simulink model "MATLAB_TEST"  (R2019b)
settings: Solver=FixedStepDiscrete  StartTime=0  StopTime=50  FixedStep=0.0025  RelTol=1e-3
undefined symbols (not defined in the file): BCM_COM_PROC_P20, BCM_COM_PROC_P20_SFW_R2018b, BCM_COM_PROC_P2_5, BCM_COM_PROC_P2_5_SFW_R2018b, BCM_COM_PROC_P5, BCM_COM_PROC_P5_SFW_R2018b, BCMA_ACCU_PT_Conf_Flt, BCMA_ACCU_PT_Unconf_Flt, BCMA_Antiskid_Off_Sanction, BCMA_Avionics_Conf_Flt, BCMA_BCM_CCDL_Conf_Flt, BCMA_BCM_CCDL_Unconf_Flt, BCMA_BCM_DBCU_INHIBITION_Conf_Flt, BCMA_BCM_DBCU_INHIBITION_Unconf_Flt, BCMA_BCP_ALT_Disp_Sw_Conf_Flt, BCMA_BCP_ALT_Disp_Sw_Unconf_Flt, BCMA_BCP_ALT_SW_ON_CMD_Conf_Flt, BCMA_BCP_ALT_SW_ON_CMD_Unconf_Flt, BCMA_BCP_PARK_OFF_SW_CMD_Conf_Flt, BCMA_BCP_PARK_OFF_SW_CMD_Unconf_Flt, BCMA_CF_BSELV_JCL, BCMA_CF_BSELV_JOP, BCMA_CF_BSELV_OC, BCMA_CF_BSELV_SC, BCMA_CF_LH_SV_JCL, BCMA_CF_LH_SV_JOP, BCMA_CF_LH_SV_OC, BCMA_CF_LH_SV_SC, BCMA_CF_PARK_BRK, BCMA_CF_RESIDUAL_PRESS, BCMA_CF_RH_SV_JCL, BCMA_CF_RH_SV_JOP, BCMA_CF_RH_SV_OC, BCMA_CF_RH_SV_SC, BCMA_CF_SELV_JCL, BCMA_CF_SELV_JOP, BCMA_CF_SELV_OC, BCMA_CF_SELV_SC, BCMA_CF_SV_DRIFT, BCMA_DBCU_ALT_MODE_Conf_Flt, BCMA_DBCU_ALT_MODE_Unconf_Flt, BCMA_DBCU_BRK_ORDER_FAIL_Conf_Flt, BCMA_DBCU_BRK_ORDER_FAIL_Unconf_Flt, BCMA_DBCU_Conf_Flt, BCMA_DBCU_DISPATCH_SW_ON_Conf_Flt, BCMA_DBCU_DISPATCH_SW_ON_Unconf_Flt, BCMA_DBCU_FAILED_Conf_Flt, BCMA_DBCU_FAILED_Unconf_Flt, BCMA_DFCS1_Capsule_Validity, BCMA_DFCS1_Label202_Corrupted, BCMA_DFCS1_Label202_Not_Refreshed, BCMA_DFCS1_Label204_Corrupted, BCMA_DFCS1_Label204_Not_Refreshed, BCMA_DFCS1_Label205_Corrupted, BCMA_DFCS1_Label205_Not_Refreshed, BCMA_DFCS1_Label206_Corrupted, BCMA_DFCS1_Label206_Not_Refreshed, BCMA_DFCS1_Label207_Corrupted, BCMA_DFCS1_Label207_Not_Refreshed, BCMA_DFCS3_Capsule_Validity ... (+762)
libraries: simulink x73, lib_MBD_Control x5
(part 2 of 16)

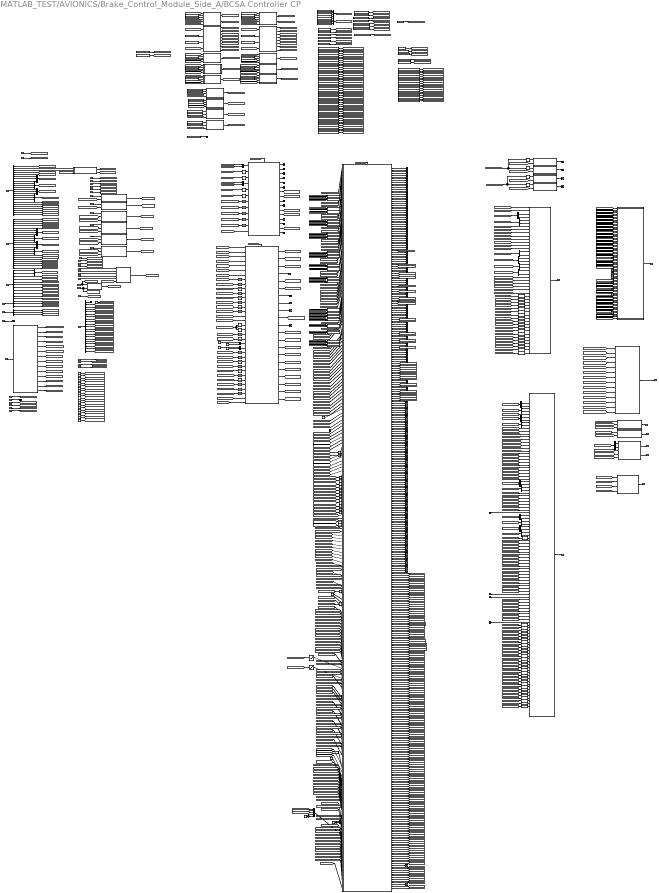
== system MATLAB_TEST/AVIONICS/Brake_Control_Module_Side_A/BCSA Controller CP ==
  note: Wheel speed order:
      | 1) Left outer
      | 2) Left inner
      | 3) Right inner
      | 4) Right outer
  note: MEX P2_5
  note: MEX P20
  note: Temporary
      | Flt computation
  note: Validity
  note: Temporary inputs
  note: Functional test
  note: MEX P5
  note: Outputs connected
  note: COM CAN MON
  note: INPUTS
  note: OUTPUTS
  note: LABEL202
  note: LABEL204
  note: LABEL205
  note: LABEL206
  note: LABEL207
  note: DFCS1
  note: DFCS3
  note: GenIO
  note: LABEL021
  note: LABEL022
  note: LABEL272
  note: LABEL273
  note: SOFTWARE
  note: Capsule validity
  note: DFCS
  note: GenIO
  note: Ethernet
  note: Only BCM A
  note: Only BCM A
  note: CAN
  note: ToDo 27439:
      | a temporary fix was implemented for MEX4
      | The data is transformed from mV into bar
      | To be deleted for future MEX release if relevant
  note: ToDo 27975
      | Fix to force the validity of SP to true inside CP
  note: MON CAN COM
  BCP_ALT_SW_ON_CMD_BCM_A_GND : Inport  Tag=ToConnect
  BCP_PARK_OFF_SW_CMD_BCM_A_GND : Inport  Tag=ToConnect  Port=2
  BUS_A429_DFCS1_BCMA : Inport  Tag=ToConnect  Port=3
  BUS_A429_DFCS3_BCMA : Inport  Tag=ToConnect  Port=4
  BUS_A429_GenIO_1A_GPHS : Inport  Tag=ToConnect  Port=5
  BUS_A429_LH_WRDC_BCM : Inport  Tag=ToConnect  Port=6
  BUS_A429_RH_WRDC_BCM : Inport  Tag=ToConnect  Port=7
  BUS_ETH_MMS_BCMA : Inport  Tag=ToConnect  Port=8
  BUS_CAN_BCM_CCDL_RX : Inport  Tag=ToConnect  Port=9
  LGCH_LG_LEVER_UP_1 : Inport  Tag=ToConnect  Port=10
  LH_ESC_WOnWdiscrete : Inport  Tag=ToConnect  Port=11
  LMLG_DOWN_LOCKED_BCM_1 : Inport  Tag=ToConnect  Port=12
  MP_MAINT_MODE_CMD_BCM_A_28V : Inport  Tag=ToConnect  Port=13
  MP_MAINT_MODE_CMD_BCM_A_GND : Inport  Tag=ToConnect  Port=14
  RMLG_DOWN_LOCKED_BCM_1 : Inport  Tag=ToConnect  Port=15
  ACCU_PT_PRESSURE : Inport  Tag=ToConnect  Port=16
  BCMB_DBCU_INHIBITION : Inport  Tag=ToConnect  Port=17
  DBCU_ALTERNATE_MODE_1 : Inport  Tag=ToConnect  Port=18
  DBCU_BRK_ORDER_FAIL_BCMA : Inport  Tag=ToConnect  Port=19
  DBCU_FAILED_BCMA : Inport  Tag=ToConnect  Port=20
  LH_DBCU_BRK_CMD_FEEDBACK : Inport  Tag=ToConnect  Port=21
  LH_HASV_PT_PRESSURE : Inport  Tag=ToConnect  Port=22
  LH_IN_WHEEL_SPEED_COIL1 : Inport  Tag=ToConnect  Port=23
  LH_OUT_BTS_TEMP : Inport  Tag=ToConnect  Port=24
  LH_OUT_WHEEL_SPEED_COIL1 : Inport  Tag=ToConnect  Port=25
  PBSELV_ON_POS : Inport  Tag=ToConnect  Port=26
  RH_DBCU_BRK_CMD_FEEDBACK : Inport  Tag=ToConnect  Port=27
  RH_HASV_PT_PRESSURE : Inport  Tag=ToConnect  Port=28
  RH_IN_WHEEL_SPEED_COIL1 : Inport  Tag=ToConnect  Port=29
  RH_OUT_BTS_TEMP : Inport  Tag=ToConnect  Port=30
  RH_OUT_WHEEL_SPEED_COIL1 : Inport  Tag=ToConnect  Port=31
  FTI_BCMA_switch_1 : Inport  Tag=ToConnect  Port=32
  FTI_BCMA_switch_2 : Inport  Tag=ToConnect  Port=33
  FTI_BCMA_switch_3 : Inport  Tag=ToConnect  Port=34
  FTI_BCMA_switch_4 : Inport  Tag=ToConnect  Port=35
  FTI_BCMA_switch_5 : Inport  Tag=ToConnect  Port=36
  PIN_PROG_BCMA_1 : Inport  Tag=ToConnect  Port=37
  PIN_PROG_BCMA_2 : Inport  Tag=ToConnect  Port=38
  PIN_PROG_BCMA_3 : Inport  Tag=ToConnect  Port=39
  MON_CAN_COM : Inport  Tag=ToConnect  Port=40
  Control_Path_Start_Up : Inport  Tag=ToConnect  Port=41
  LH_HASV_CURRENT_COIL1_Readback : Inport  Tag=ToConnect  Port=42  OutDataTypeStr=double
  RH_HASV_CURRENT_COIL1_Readback : Inport  Tag=ToConnect  Port=43  OutDataTypeStr=double
  HASELV_CMD_Readback : Inport  Tag=ToConnect  Port=44  OutDataTypeStr=double
  BCM Config Computation : Subsystem
  BCMA_COM_UF_LOCKED_WHEEL_W{1..4} (4 alike) : Constant  Value=0  OutDataTypeStr=boolean
  BCM_COM_PROC_P20 : Subsystem  SystemSampleTime=0.02
  BCM_COM_PROC_P2_5 : Subsystem  SystemSampleTime=0.0025
  BCM_COM_PROC_P5 : Subsystem  SystemSampleTime=0.005
  BUS_A429_BCMA_DFCS13_TX : Subsystem
  BUS_A429_BCMA_GenIO_2_TX : Subsystem
  BUS_CAN_BCM_CCDL_RX_ : Subsystem
  BUS_CAN_BCM_CCDL_TX : Subsystem
  BUS_ETH_BCMA_MMS_TX : Subsystem
  Bus Selector : BusSelector  OutputSignals=BUS_A429_DFCS1_BCMA_LABEL_206_Ground_Speed,BUS_A429_DFCS1_BCMA_LABEL_202_DFCS_LH_Braking_Cmd,BUS_A429_DFCS1_BCMA_LABEL_202_DFCS_RH_Braking_Cmd,BUS_A429_DFCS1_BCMA_LABEL_205_Longitudinal_Acceleration,BUS_A429_DFCS1_BCMA_LABEL_207_Pitch_Angle,BUS_A429_DFCS1_BCMA_LABEL_204_DATA_BIT_14_WOW1_Validity,BUS_A429_DFCS1_BCMA_LABEL_204_DATA_BIT_18_WOW2_Validity,BUS_A429_DFCS1_BCMA_LABEL_204_DATA_BIT_22_WOW3_Validity,BUS_A429_DFCS1_BCMA_LABEL_204_DATA_BIT_12_WOW1_LMLG,BUS_A429_DFCS1_BCMA_LABEL_204_DATA_BIT_16_WOW2_LMLG,BUS_A429_DFCS1_BCMA_LABEL_204_DATA_BIT_20_WOW3_LMLG,BUS_A429_DFCS1_BCMA_LABEL_204_DATA_BIT_13_WOW1_RMLG,BUS_A429_DFCS1_BCMA_LABEL_204_DATA_BIT_17_WOW2_RMLG,BUS_A429_DFCS1_BCMA_LABEL_204_DATA_BIT_21_WOW3_RMLG,BUS_A429_DFCS1_BCMA_LABEL_204_DATA_BIT_11_WOW1_NLG,BUS_A429_DFCS1_BCMA_LABEL_204_DATA_BIT_15_WOW2_NLG,BUS_A429_DFCS1_BCMA_LABEL_204_DATA_BIT_19_WOW3_NLG,BUS_A429_DFCS1_BCMA_LABEL_204_DATA_BIT_24_Decel_Law_Inhibition,BUS_A429_DFCS1_BCMA_LABEL_204_DATA_BIT_27_TLA_Above_Idle,BUS_A429_DFCS1_BCMA_LABEL_202_SSM,BUS_A429_DFCS1_BCMA_LABEL_204_SSM,BUS_A429_DFCS1_BCMA_LABEL_205_SSM,BUS_A429_DFCS1_BCMA_LABEL_206_SSM,BUS_A429_DFCS1_BCMA_LABEL_207_SSM
  Bus Selector1 : BusSelector  OutputSignals=BUS_A429_DFCS3_BCMA_LABEL_206_Ground_Speed,BUS_A429_DFCS3_BCMA_LABEL_202_DFCS_LH_Braking_Cmd,BUS_A429_DFCS3_BCMA_LABEL_202_DFCS_RH_Braking_Cmd,BUS_A429_DFCS3_BCMA_LABEL_205_Longitudinal_Acceleration,BUS_A429_DFCS3_BCMA_LABEL_207_Pitch_Angle,BUS_A429_DFCS3_BCMA_LABEL_204_DATA_BIT_14_WOW1_Validity,BUS_A429_DFCS3_BCMA_LABEL_204_DATA_BIT_18_WOW2_Validity,BUS_A429_DFCS3_BCMA_LABEL_204_DATA_BIT_22_WOW3_Validity,BUS_A429_DFCS3_BCMA_LABEL_204_DATA_BIT_12_WOW1_LMLG,BUS_A429_DFCS3_BCMA_LABEL_204_DATA_BIT_16_WOW2_LMLG,BUS_A429_DFCS3_BCMA_LABEL_204_DATA_BIT_20_WOW3_LMLG,BUS_A429_DFCS3_BCMA_LABEL_204_DATA_BIT_13_WOW1_RMLG,BUS_A429_DFCS3_BCMA_LABEL_204_DATA_BIT_17_WOW2_RMLG,BUS_A429_DFCS3_BCMA_LABEL_204_DATA_BIT_21_WOW3_RMLG,BUS_A429_DFCS3_BCMA_LABEL_204_DATA_BIT_11_WOW1_NLG,BUS_A429_DFCS3_BCMA_LABEL_204_DATA_BIT_15_WOW2_NLG,BUS_A429_DFCS3_BCMA_LABEL_204_DATA_BIT_19_WOW3_NLG,BUS_A429_DFCS3_BCMA_LABEL_204_DATA_BIT_24_Decel_Law_Inhibition,BUS_A429_DFCS3_BCMA_LABEL_204_DATA_BIT_27_TLA_Above_Idle,BUS_A429_DFCS3_BCMA_LABEL_202_SSM,BUS_A429_DFCS3_BCMA_LABEL_204_SSM,BUS_A429_DFCS3_BCMA_LABEL_205_SSM,BUS_A429_DFCS3_BCMA_LABEL_206_SSM,BUS_A429_DFCS3_BCMA_LABEL_207_SSM
  Bus Selector2 : BusSelector  OutputSignals=BUS_A429_GenIO_1A_GPHS_LABEL_272_ENG1_Engine_Running,BUS_A429_GenIO_1A_GPHS_LABEL_273_ENG2_Engine_Running,BUS_A429_GenIO_1A_GPHS_LABEL_022_HCM_SYS_A_PRESSURE,BUS_A429_GenIO_1A_GPHS_LABEL_021_HCM_SYS_B_PRESSURE,BUS_A429_GenIO_1A_GPHS_LABEL_150_UTC_time_hours_2,BUS_A429_GenIO_1A_GPHS_LABEL_150_UTC_time_minutes_2,BUS_A429_GenIO_1A_GPHS_LABEL_150_UTC_time_seconds_2,BUS_A429_GenIO_1A_GPHS_LABEL_021_SSM,BUS_A429_GenIO_1A_GPHS_LABEL_022_SSM,BUS_A429_GenIO_1A_GPHS_LABEL_272_SSM,BUS_A429_GenIO_1A_GPHS_LABEL_273_SSM
  Bus Selector3 : BusSelector  OutputSignals=V_BCMA_MON_BCM_Validity_SP,V_BCMA_MON_A429_SSM_DFCS_Label_121,V_BCMA_MON_A429_SSM_DFCS_Label_122,V_BCMA_MON_A429_SSM_DFCS_Label_123,V_BCMA_MON_A429_SSM_DFCS_Label_124,V_BCMA_MON_A429_SSM_DFCS_Label_125,V_BCMA_MON_A429_SSM_DFCS_Label_126,V_BCMA_MON_A429_SSM_DFCS_Label_127,V_BCMA_MON_A429_SSM_DFCS_Label_130,V_BCMA_MON_A429_SSM_DFCS_Label_131,V_BCMA_MON_A429_SSM_DFCS_Label_150,V_BCMA_MON_A429_SSM_DFCS_Label_151,V_BCMA_MON_A429_SP_Wheel_Speed_W12,V_BCMA_MON_A429_SP_Wheel_Speed_W34,V_BCMA_MON_A429_SP_SV_PT_PSI,V_BCMA_MON_A429_SP_LH_Brkg_Cmd_Fdbk,V_BCMA_MON_A429_SP_RH_Brkg_Cmd_Fdbk,V_BCMA_MON_A429_SP_DFCS_A_Caps_Fail,V_BCMA_MON_A429_SP_DFCS_B_Caps_Fail,V_BCMA_MON_A429_SP_BCM_Passivated,V_BCMA_MON_A429_SP_BCM_Failed
  Bus Selector4 : BusSelector  OutputSignals=BUS_A429_LH_WRDC_BCM_LABEL_300_TyrePressure_W_1_R_LN,BUS_A429_LH_WRDC_BCM_LABEL_301_TyrePressure_W_2_R_LN,BUS_A429_LH_WRDC_BCM_LABEL_302_TyrePressure_W_3_R_LN
  Bus Selector5 : BusSelector  OutputSignals=BUS_A429_RH_WRDC_BCM_LABEL_300_TyrePressure_W_1_R_LN,BUS_A429_RH_WRDC_BCM_LABEL_301_TyrePressure_W_2_R_LN,BUS_A429_RH_WRDC_BCM_LABEL_302_TyrePressure_W_3_R_LN
  COM_CAN_MON_TX : Subsystem
  Constant{,35..36,44,87,94,97,100..101,104,107..118} (22 alike) : Constant  Value=0  OutDataTypeStr=boolean
  Constant1 : Constant  Value=BCMA_DFCS1_Label206_Not_Refreshed  OutDataTypeStr=boolean  SampleTime=Inf
  Constant10 : Constant  Value=BCMA_DFCS1_Label202_Not_Refreshed  OutDataTypeStr=boolean  SampleTime=Inf
  Constant11 : Constant  Value=BCMA_DFCS1_Label204_Not_Refreshed  OutDataTypeStr=boolean  SampleTime=Inf
  Constant119 : Constant  Value=BCMA_UTC_Time_Seconds_Unconf_Flt
  Constant12 : Constant  Value=BCMA_DFCS1_Label205_Not_Refreshed  OutDataTypeStr=boolean  SampleTime=Inf
  Constant120 : Constant  Value=BCMA_DBCU_BRK_ORDER_FAIL_Conf_Flt
  Constant121 : Constant  Value=BCMA_DBCU_BRK_ORDER_FAIL_Unconf_Flt
  Constant122 : Constant  Value=BCMA_DBCU_DISPATCH_SW_ON_Conf_Flt
  Constant123 : Constant  Value=BCMA_DBCU_DISPATCH_SW_ON_Unconf_Flt
  Constant124 : Constant  Value=BCMA_LH_DBCU_BRK_CMD_FDBK_Conf_Flt
  Constant125 : Constant  Value=BCMA_LH_DBCU_BRK_CMD_FDBK_Unconf_Flt
  Constant126 : Constant  Value=BCMA_RH_DBCU_BRK_CMD_FDBK_Conf_Flt
  Constant127 : Constant  Value=BCMA_RH_DBCU_BRK_CMD_FDBK_Unconf_Flt
  Constant128 : Constant  Value=BCMA_DBCU_FAILED_Conf_Flt
  Constant129 : Constant  Value=BCMA_BCM_CCDL_Unconf_Flt
  Constant13 : Constant  Value=BCMA_DFCS1_Label205_Corrupted  OutDataTypeStr=boolean  SampleTime=Inf
  Constant130 : Constant  Value=BCMA_DBCU_FAILED_Unconf_Flt
  Constant131 : Constant  Value=BCMA_DBCU_ALT_MODE_Conf_Flt
  Constant132 : Constant  Value=BCMA_DBCU_ALT_MODE_Unconf_Flt
  Constant133 : Constant  Value=BCMA_ACCU_PT_Conf_Flt
  Constant134 : Constant  Value=BCMA_ACCU_PT_Unconf_Flt
  Constant135 : Constant  Value=BCMA_LH_BTS_Conf_Flt
  Constant136 : Constant  Value=BCMA_LH_BTS_Unconf_Flt
  Constant137 : Constant  Value=BCMA_RH_BTS_Conf_Flt
  Constant138 : Constant  Value=BCMA_RH_BTS_Unconf_Flt
  Constant139 : Constant  Value=BCMA_BCP_PARK_OFF_SW_CMD_Conf_Flt
  Constant14 : Constant  Value=BCMA_DFCS1_Label207_Not_Refreshed  OutDataTypeStr=boolean  SampleTime=Inf
  Constant140 : Constant  Value=BCMA_BCM_DBCU_INHIBITION_Conf_Flt
  Constant141 : Constant  Value=BCMA_BCP_PARK_OFF_SW_CMD_Unconf_Flt
  Constant142 : Constant  Value=BCMA_LNLG_Tire_Press_Conf_Flt
  Constant143 : Constant  Value=BCMA_LNLG_Tire_Press_Unconf_Flt
  Constant144 : Constant  Value=BCMA_RNLG_Tire_Press_Conf_Flt
  Constant145 : Constant  Value=BCMA_RNLG_Tire_Press_Unconf_Flt
  Constant146 : Constant  Value=BCMA_LMLG_Outboard_Tire_Press_Conf_Flt
  Constant147 : Constant  Value=BCMA_LMLG_Outboard_Tire_Press_Unconf_Flt
  Constant148 : Constant  Value=BCMA_LMLG_Inboard_Tire_Press_Conf_Flt
  Constant149 : Constant  Value=BCMA_LMLG_Inboard_Tire_Press_Unconf_Flt
  Constant15 : Constant  Value=BCMA_DFCS1_Label206_Corrupted  OutDataTypeStr=boolean  SampleTime=Inf
  Constant150 : Constant  Value=BCMA_RMLG_Inboard_Tire_Press_Conf_Flt
  Constant151 : Constant  Value=BCMA_BCM_DBCU_INHIBITION_Unconf_Flt
  Constant152 : Constant  Value=BCMA_RMLG_Inboard_Tire_Press_Unconf_Flt
  Constant153 : Constant  Value=BCMA_RMLG_Outboard_Tire_Press_Conf_Flt
  Constant154 : Constant  Value=BCMA_RMLG_Outboard_Tire_Press_Unconf_Flt
  Constant155 : Constant  Value=BCMA_Avionics_Conf_Flt
  Constant156 : Constant  Value=BCMA_DFCS_A_Conf_Flt
  Constant157 : Constant  Value=BCMA_DFCS_B_Conf_Flt
  Constant158 : Constant  Value=BCMA_DBCU_Conf_Flt
  Constant159 : Constant  Value=BCMA_LH_SV_PT_Conf_Flt
  Constant16 : Constant  Value=BCMA_Tacho1_Conf_Flt  OutDataTypeStr=boolean  SampleTime=Inf
  Constant160 : Constant  Value=BCMA_RH_SV_PT_Conf_Flt
  Constant161 : Constant  Value=BCMA_UTC_Time_Hours_Conf_Flt
  Constant162 : Constant  Value=BCMA_UTC_Time_Hours_Unconf_Flt
  Constant163 : Constant  Value=BCMA_UTC_Time_Minutes_Conf_Flt
  Constant164 : Constant  Value=BCMA_UTC_Time_Minutes_Unconf_Flt
  Constant165 : Constant  Value=BCMA_UTC_Time_Seconds_Conf_Flt
  Constant17 : Constant  Value=BCMA_DFCS1_Label207_Corrupted  OutDataTypeStr=boolean  SampleTime=Inf
  Constant18 : Constant  Value=BCMA_DFCS3_Label205_Corrupted  OutDataTypeStr=boolean  SampleTime=Inf
  Constant19 : Constant  Value=BCMA_DFCS3_Label202_Not_Refreshed  OutDataTypeStr=boolean  SampleTime=Inf
  Constant2 : Constant  Value=BCMA_Tacho1_Unconf_Flt  OutDataTypeStr=boolean  SampleTime=Inf
  Constant20 : Constant  Value=BCMA_DFCS3_Label206_Not_Refreshed  OutDataTypeStr=boolean  SampleTime=Inf
  Constant21 : Constant  Value=BCMA_DFCS3_Label202_Corrupted  OutDataTypeStr=boolean  SampleTime=Inf
  Constant22 : Constant  Value=BCMA_DFCS3_Label206_Corrupted  OutDataTypeStr=boolean  SampleTime=Inf
  Constant23 : Constant  Value=BCMA_DFCS3_Label207_Not_Refreshed  OutDataTypeStr=boolean  SampleTime=Inf
  Constant24 : Constant  Value=BCMA_DFCS3_Label207_Corrupted  OutDataTypeStr=boolean  SampleTime=Inf
  Constant25 : Constant  Value=BCMA_Off_Sanction  OutDataTypeStr=boolean  SampleTime=Inf
  Constant26 : Constant  OutDataTypeStr=boolean
  Constant27 : Constant  Value=BCMA_SP_TO_CP_Link_Validity  OutDataTypeStr=boolean  SampleTime=Inf
  Constant29 : Constant  Value=BCMA_BCP_ALT_SW_ON_CMD_Unconf_Flt  OutDataTypeStr=boolean  SampleTime=Inf
  Constant3 : Constant  Value=BCMA_DFCS3_Label204_Not_Refreshed  OutDataTypeStr=boolean  SampleTime=Inf
  Constant30 : Constant  Value=BCMA_BCM_CCDL_Conf_Flt
  Constant31 : Constant  Value=BCMA_GenIO_1A_Label021_Not_Refreshed  OutDataTypeStr=boolean  SampleTime=Inf
  Constant32 : Constant  Value=BCMA_GenIO_1A_Label021_Corrupted  OutDataTypeStr=boolean  SampleTime=Inf
  Constant33 : Constant  Value=BCMA_GenIO_1A_Label022_Not_Refreshed  OutDataTypeStr=boolean  SampleTime=Inf
  Constant34 : Constant  Value=BCMA_GenIO_1A_Label022_Corrupted  OutDataTypeStr=boolean  SampleTime=Inf
  Constant37 : Constant  Value=BCMA_GenIO_1A_Label272_Not_Refreshed  OutDataTypeStr=boolean  SampleTime=Inf
  Constant38 : Constant  Value=BCMA_LG_Lever_Up_Unconf_Flt  OutDataTypeStr=boolean  SampleTime=Inf
  Constant39 : Constant  Value=BCMA_LG_Lever_Up_Conf_Flt  OutDataTypeStr=boolean  SampleTime=Inf
  Constant4 : Constant  Value=BCMA_DFCS1_Label202_Corrupted  OutDataTypeStr=boolean  SampleTime=Inf
  Constant40 : Constant  Value=BCMA_LMLG_Downlock_Unconf_Flt  OutDataTypeStr=boolean  SampleTime=Inf
  Constant41 : Constant  Value=BCMA_LMLG_Downlock_Conf_Flt  OutDataTypeStr=boolean  SampleTime=Inf
  Constant42 : Constant  Value=BCMA_RMLG_Downlock_Unconf_Flt  OutDataTypeStr=boolean  SampleTime=Inf
  Constant43 : Constant  Value=BCMA_RMLG_Downlock_Conf_Flt  OutDataTypeStr=boolean  SampleTime=Inf
  Constant45 : Constant  Value=BCMA_CF_LH_SV_SC
  Constant46 : Constant  Value=BCMA_BCP_ALT_SW_ON_CMD_Conf_Flt  OutDataTypeStr=boolean  SampleTime=Inf
  Constant47 : Constant  Value=BCMA_BCP_ALT_Disp_Sw_Unconf_Flt  OutDataTypeStr=boolean  SampleTime=Inf
  Constant48 : Constant  Value=BCMA_BCP_ALT_Disp_Sw_Conf_Flt  OutDataTypeStr=boolean  SampleTime=Inf
  Constant49 : Constant  Value=BCMA_GenIO_1A_Label272_Corrupted  OutDataTypeStr=boolean  SampleTime=Inf
  Constant5 : Constant  Value=BCMA_DFCS3_Label204_Corrupted  OutDataTypeStr=boolean  SampleTime=Inf
  Constant50 : Constant  Value=BCMA_Antiskid_Off_Sanction  OutDataTypeStr=boolean  SampleTime=Inf
  Constant51 : Constant  Value=BCMA_Norm_Brk_Off_Sanction  OutDataTypeStr=boolean  SampleTime=Inf
  Constant52 : Constant  Value=0  OutDataTypeStr=int32  SampleTime=Inf
  Constant54 : Constant  Value=BCMA_Tacho2_Conf_Flt  OutDataTypeStr=boolean  SampleTime=Inf
  Constant55 : Constant  Value=BCMA_GenIO_1A_Label273_Not_Refreshed  OutDataTypeStr=boolean  SampleTime=Inf
  Constant56 : Constant  Value=BCMA_GenIO_1A_Label273_Corrupted  OutDataTypeStr=boolean  SampleTime=Inf
  Constant57 : Constant  Value=BCMA_CF_RESIDUAL_PRESS
  Constant58 : Constant  Value=BCMA_CF_BSELV_OC
  Constant59 : Constant  Value=BCMA_CF_BSELV_SC
  Constant6 : Constant  Value=BCMA_DFCS1_Label204_Corrupted  OutDataTypeStr=boolean  SampleTime=Inf
  Constant60 : Constant  Value=BCMA_CF_BSELV_JCL
  Constant61 : Constant  Value=BCMA_CF_BSELV_JOP
  Constant62 : Constant  Value=BCMA_PPRG_Fault
  Constant63 : Constant  Value=BCMA_CF_SV_DRIFT
  Constant64 : Constant  Value=BCMA_CF_LH_SV_JCL
  Constant65 : Constant  Value=BCMA_CF_LH_SV_JOP
  Constant67 : Constant  Value=BCMA_CF_LH_SV_OC
  Constant68 : Constant  Value=BCMA_CF_RH_SV_JCL
  Constant69 : Constant  Value=BCMA_CF_RH_SV_JOP
  Constant7 : Constant  Value=BCMA_DFCS3_Label205_Not_Refreshed  OutDataTypeStr=boolean  SampleTime=Inf
  Constant70 : Constant  Value=BCMA_CF_RH_SV_SC
  Constant71 : Constant  Value=BCMA_CF_RH_SV_OC
  Constant72 : Constant  Value=BCMA_Tacho3_Conf_Flt  OutDataTypeStr=boolean  SampleTime=Inf
  Constant73 : Constant  Value=BCMA_Tacho4_Conf_Flt  OutDataTypeStr=boolean  SampleTime=Inf
  Constant74 : Constant  Value=BCMA_Tacho2_Unconf_Flt  OutDataTypeStr=boolean  SampleTime=Inf
  Constant75 : Constant  Value=BCMA_Tacho3_Unconf_Flt  OutDataTypeStr=boolean  SampleTime=Inf
  Constant76 : Constant  Value=BCMA_Tacho4_Unconf_Flt  OutDataTypeStr=boolean  SampleTime=Inf
  Constant77 : Constant  Value=BCMA_CF_SELV_SC
  Constant78 : Constant  Value=BCMA_CF_SELV_OC
  Constant79 : Constant  Value=BCMA_CF_SELV_JOP
  Constant8 : Constant  Value=BCMA_DFCS1_Capsule_Validity  OutDataTypeStr=boolean  SampleTime=Inf
  Constant80 : Constant  Value=BCMA_LH_ALT_BRK_LOSS_Manual  OutDataTypeStr=boolean  SampleTime=Inf
  Constant81 : Constant  Value=BCMA_RH_ALT_BRK_LOSS_Manual  OutDataTypeStr=boolean  SampleTime=Inf
  Constant82 : Constant  Value=BCMA_PBSELV_ON_POS_Unconf_Flt  OutDataTypeStr=boolean  SampleTime=Inf
  Constant83 : Constant  Value=BCMA_PBSELV_ON_POS_Conf_Flt  OutDataTypeStr=boolean  SampleTime=Inf
  Constant84 : Constant  Value=BCMA_CF_SELV_JCL
  Constant85 : Constant  Value=BCMA_CF_PARK_BRK
  Constant88 : Constant  Value=BCMA_LH_SV_PT_Unconf_Flt  OutDataTypeStr=boolean  SampleTime=Inf
  Constant9 : Constant  Value=BCMA_DFCS3_Capsule_Validity  OutDataTypeStr=boolean  SampleTime=Inf
  Constant90 : Constant  Value=BCMA_RH_SV_PT_Unconf_Flt  OutDataTypeStr=boolean  SampleTime=Inf
  DBCU Inhibition Failure Mode : Subsystem
  DFCS1_Label204_Validity : Subsystem
  DFCS1_Label205_Validity : Subsystem
  DFCS1_Label206_Validity : Subsystem
  DFCS1_Label207_Validity : Subsystem
  DFCS3_Label204_Validity : Subsystem
  DFCS3_Label205_Validity : Subsystem
  DFCS3_Label206_Validity : Subsystem
  DFCS3_Label207_Validity : Subsystem
  DFCSA_DCL_Inhibition_Comp : Subsystem
  DFCSA_Ground_Speed_Comp : Subsystem
  DFCSA_LH_Braking_Cmd_Comp : Subsystem
  DFCSA_LMLG_WOWs_Comp : Subsystem
  DFCSA_Label202_Validity : Subsystem
  DFCSA_Long_Accel_Comp : Subsystem
  DFCSA_NLG_WOWs_Comp : Subsystem
  DFCSA_Pitch_Angle_Comp : Subsystem
  DFCSA_RH_Braking_Cmd_Comp : Subsystem
  DFCSA_RMLG_WOWs_Comp : Subsystem
  DFCSA_TLA_Above_Idle_Comp : Subsystem
  DFCSA_WOWs_Val_Comp : Subsystem
  DFCSB_DCL_Inhibition_Comp : Subsystem
  DFCSB_Ground_Speed_Comp : Subsystem
  DFCSB_LH_Braking_Cmd_Comp : Subsystem
  DFCSB_LMLG_WOWs_Comp : Subsystem
  DFCSB_Label202_Validity1 : Subsystem
  DFCSB_Long_Accel_Comp : Subsystem
  DFCSB_NLG_WOWs_Comp : Subsystem
  DFCSB_Pitch_Angle_Comp : Subsystem
  DFCSB_RH_Braking_Cmd_Comp : Subsystem
  DFCSB_RMLG_WOWs_Comp : Subsystem
  DFCSB_TLA_Above_Idle_Comp : Subsystem
  DFCSB_WOWs_Val_Comp : Subsystem
  Data Type Conversion{,1..49} (50 alike) : DataTypeConversion  OutDataTypeStr=uint32
  Demux{,1..16} (17 alike) : Demux  Outputs=2
  GenIO_Label021_Validity : Subsystem
  GenIO_Label022_Validity : Subsystem
  GenIO_Label272_Validity : Subsystem
  GenIO_Label273_Validity : Subsystem
  Ground{,1..7,76,87..91,105..108} (18 alike) : Ground
  Inadvertent Braking Order BSELV Failure Mode : Subsystem
  Inadvertent Braking Order DBSMA Failure Mode : Subsystem
  Inadvertent Braking Order Failure Mode : Subsystem
  Left Inner Wheel Speed Emission Failure Mode : Subsystem
  Left Inner Wheel Speed Failure Modes : Subsystem
  Left Outer Wheel Speed Emission Failure Mode : Subsystem
  Left Outer Wheel Speed Failure Modes : Subsystem
  Left Pressure Transducer Failure Mode : Subsystem
  Logical Operator1 : Logic  Operator=NOT  AllPortsSameDT=off  OutDataTypeStr=boolean
  Logical Operator2 : Logic  Operator=NOT  AllPortsSameDT=off  OutDataTypeStr=boolean
  Mux{,3,8..10,15,17} (7 alike) : Mux  Inputs=2
  Mux{1..2,4..5,11..14} (8 alike) : Mux  Inputs=3
  Mux16 : Mux  Inputs=5
  Mux24 : Mux
  Mux25 : Mux
  Pin_Prog : Constant  Value=0  OutDataTypeStr=boolean
  Right Inner Wheel Speed Emission Failure Mode : Subsystem
  Right Inner Wheel Speed Failure Modes : Subsystem
  Right Outer Wheel Speed Emission Failure Mode : Subsystem
  Right Outer Wheel Speed Failure Modes : Subsystem
  Right Pressure Transducer Failure Mode : Subsystem
  Selector : Selector  InputPortWidth=4  IndexOptions=Index vector (dialog)  Indices=[1 2]  OutputSizes=1
  Selector1 : Selector  InputPortWidth=4  IndexOptions=Index vector (dialog)  Indices=[3 4]  OutputSizes=1
  Selector2 : Selector  InputPortWidth=4  IndexOptions=Index vector (dialog)  Indices=[1 2]  OutputSizes=1
  Selector3 : Selector  InputPortWidth=4  IndexOptions=Index vector (dialog)  Indices=[3 4]  OutputSizes=1
  Selector4 : Selector  InputPortWidth=2  IndexOptions=Index vector (dialog)  Indices=2  OutputSizes=1
  Selector5 : Selector  InputPortWidth=2  IndexOptions=Index vector (dialog)  Indices=1  OutputSizes=1
  Selector6 : Selector  InputPortWidth=2  IndexOptions=Index vector (dialog)  Indices=1  OutputSizes=1
  Selector7 : Selector  InputPortWidth=2  IndexOptions=Index vector (dialog)  Indices=2  OutputSizes=1
  Selector8 : Selector  InputPortWidth=4  IndexOptions=Index vector (dialog)  Indices=[1 2]  OutputSizes=1
  Selector9 : Selector  InputPortWidth=4  IndexOptions=Index vector (dialog)  Indices=[3 4]  OutputSizes=1
  "Temperature Sensor Conversion Law mV -> °C" : Lookup_n-D  NumberOfTableDimensions=1  BreakpointsForDimension1=BRK_TEMP_Table_mV  Table=BRK_TEMP_Table_C  InternalRulePriority=Speed  RndMeth=Simplest  InputSameDT=on
  "Temperature Sensor Conversion Law mV -> °C1" : Lookup_n-D  NumberOfTableDimensions=1  BreakpointsForDimension1=BRK_TEMP_Table_mV  Table=BRK_TEMP_Table_C  InternalRulePriority=Speed  RndMeth=Simplest  InputSameDT=on
  Terminator{,1..24,26..28,30..36,38,40..78,80..81,83..84,86..111,113..120,122..226,254,388} (220 alike) : Terminator
  Tuning Management : Subsystem
  Unit Delay{,1..39,42} (41 alike) : UnitDelay  SampleTime=-1  HasFrameUpgradeWarning=on
  V_BCM_COM_SELV_High_Side_Readback_Val : Constant  OutDataTypeStr=boolean
  V_BCM_COM_SV_Current_Readback_Val : Constant  OutDataTypeStr=boolean
  BUS_A429_BCMA_DFCS13 : Outport  Tag=ToConnect  OutputWhenDisabled=reset  InitialOutput=0  VectorParamsAs1DForOutWhenUnconnected=off
      settings: AttributesFormatString=|
      | OutputWhenDisabled %<OutputWhenDisabled>
      | InitialOutput %<InitialOutput>
  BUS_A429_BCMA_GenIO_2 : Outport  Tag=ToConnect  Port=2  OutputWhenDisabled=reset  InitialOutput=0  VectorParamsAs1DForOutWhenUnconnected=off
      settings: AttributesFormatString=|
      | OutputWhenDisabled %<OutputWhenDisabled>
      | InitialOutput %<InitialOutput>
  BUS_ETH_BCMA_MMS : Outport  Tag=ToConnect  Port=3  OutputWhenDisabled=reset  InitialOutput=0  VectorParamsAs1DForOutWhenUnconnected=off
      settings: AttributesFormatString=|
      | OutputWhenDisabled %<OutputWhenDisabled>
      | InitialOutput %<InitialOutput>
  BUS_CAN_BCM_CCDL : Outport  Tag=ToConnect  Port=4  OutputWhenDisabled=reset  InitialOutput=0  VectorParamsAs1DForOutWhenUnconnected=off
      settings: AttributesFormatString=|
      | OutputWhenDisabled %<OutputWhenDisabled>
      | InitialOutput %<InitialOutput>
  BCMA_DBCU_INHIBITION : Outport  Tag=ToConnect  Port=5  OutputWhenDisabled=reset  InitialOutput=0  VectorParamsAs1DForOutWhenUnconnected=off
      settings: AttributesFormatString=|
      | OutputWhenDisabled %<OutputWhenDisabled>
      | InitialOutput %<InitialOutput>
  HASELV_CMD : Outport  Tag=ToConnect  Port=6  OutputWhenDisabled=reset  InitialOutput=0  VectorParamsAs1DForOutWhenUnconnected=off
      settings: AttributesFormatString=|
      | OutputWhenDisabled %<OutputWhenDisabled>
      | InitialOutput %<InitialOutput>
  LH_HASV_CURRENT : Outport  Tag=ToConnect  Port=7  OutputWhenDisabled=reset  InitialOutput=0  VectorParamsAs1DForOutWhenUnconnected=off
      settings: AttributesFormatString=|
      | OutputWhenDisabled %<OutputWhenDisabled>
      | InitialOutput %<InitialOutput>
  RH_HASV_CURRENT : Outport  Tag=ToConnect  Port=8  OutputWhenDisabled=reset  InitialOutput=0  VectorParamsAs1DForOutWhenUnconnected=off
      settings: AttributesFormatString=|
      | OutputWhenDisabled %<OutputWhenDisabled>
      | InitialOutput %<InitialOutput>
  COM_CAN_MON : Outport  Tag=ToConnect  Port=9  OutputWhenDisabled=reset  InitialOutput=0  VectorParamsAs1DForOutWhenUnconnected=off
      settings: AttributesFormatString=|
      | OutputWhenDisabled %<OutputWhenDisabled>
      | InitialOutput %<InitialOutput>
  wires:
  BCP_ALT_SW_ON_CMD_BCM_A_GND/1 -> [BCP_ALT_SW_ON_CMD]
  BCP_PARK_OFF_SW_CMD_BCM_A_GND/1 -> [BCP_PARK_OFF_SW_CMD]
  BUS_A429_DFCS1_BCMA/1 -> Bus Selector/1
  BUS_A429_GenIO_1A_GPHS/1 -> Bus Selector2/1
  LGCH_LG_LEVER_UP_1/1 -> [LG_Lever_Up]
  LH_ESC_WOnWdiscrete/1 -> Terminator6/1
  LMLG_DOWN_LOCKED_BCM_1/1 -> [LMLG_Downlock]
  MP_MAINT_MODE_CMD_BCM_A_28V/1 -> [MP_MAINT_MODE_CMD_BCM_28V]
  MP_MAINT_MODE_CMD_BCM_A_GND/1 -> [MP_MAINT_MODE_CMD_BCM_GND]
  RMLG_DOWN_LOCKED_BCM_1/1 -> [RMLG_Downlock]
  BCMB_DBCU_INHIBITION/1 -> [BCMB_DBCU_INHIBITION]
  DBCU_ALTERNATE_MODE_1/1 -> [DBCU_ALTERNATE_MODE]
  DBCU_BRK_ORDER_FAIL_BCMA/1 -> [DBCU_BRK_ORDER_FAIL]
  DBCU_FAILED_BCMA/1 -> [DBCU_FAILED]
  LH_DBCU_BRK_CMD_FEEDBACK/1 -> [LH_DBCU_BRK_CMD_FEEDBACK]
  LH_OUT_BTS_TEMP/1 -> [LH_BTS_TEMP]
  RH_DBCU_BRK_CMD_FEEDBACK/1 -> [RH_DBCU_BRK_CMD_FEEDBACK]
  ACCU_PT_PRESSURE/1 -> [ACCU_PT_PRESSURE]
  PBSELV_ON_POS/1 -> [PBSELV_ON_POS]
  RH_OUT_BTS_TEMP/1 -> [RH_BTS_TEMP]
  BUS_ETH_MMS_BCMA/1 -> Terminator27/1
  BUS_A429_BCMA_DFCS13_TX/1(BUS_A429_BCMA_DFCS13) -> BUS_A429_BCMA_DFCS13/1
  FTI_BCMA_switch_1/1 -> Tuning Management/1(FTI_switch_1)
  FTI_BCMA_switch_2/1 -> Tuning Management/2(FTI_switch_2)
  FTI_BCMA_switch_3/1 -> Tuning Management/3(FTI_switch_3)
  FTI_BCMA_switch_4/1 -> Tuning Management/4(FTI_switch_4)
  FTI_BCMA_switch_5/1 -> Tuning Management/5(FTI_switch_5)
  PIN_PROG_BCMA_1/1 -> [PIN_PROG_BCM_1], BCM Config Computation/1(PINPROG_BCM_1)
  PIN_PROG_BCMA_2/1 -> [PIN_PROG_BCM_2], BCM Config Computation/2(PINPROG_BCM_2)
  PIN_PROG_BCMA_3/1 -> [PIN_PROG_BCM_3]
  MON_CAN_COM/1 -> Bus Selector3/1
  BUS_A429_BCMA_GenIO_2_TX/1(BUS_A429_BCMA_GenIO_2) -> BUS_A429_BCMA_GenIO_2/1
  BUS_A429_LH_WRDC_BCM/1 -> Bus Selector4/1
  BUS_A429_RH_WRDC_BCM/1 -> Bus Selector5/1
  Mux/1 -> BCM_COM_PROC_P2_5/1(V_BCM_COM_Tacho_Acq_W12)
  Mux3/1 -> BCM_COM_PROC_P2_5/4(V_BCM_COM_Tacho_Acq_W34)
  [RH_OUT_WHEEL_SPEED] -> Mux3/2
  [RH_IN_WHEEL_SPEED] -> Mux3/1
  BCM_COM_PROC_P2_5/1(V_BCM_COM_Wheel_Speed_Cons_W12) -> Terminator22/1  "V_BCMA_COM_LG_Wheel_Speed_Cons_W12"
  BCM_COM_PROC_P2_5/2(V_BCM_COM_Wheel_Speed_W12) -> Terminator8/1  "V_BCMA_COM_Wheel_Speed_W12"
  BCM_COM_PROC_P2_5/3(V_BCM_COM_Wheel_Speed_Val_W12) -> Terminator17/1  "V_BCMA_COM_Wheel_Speed_Val_W12"
  BCM_COM_PROC_P2_5/4(V_BCM_COM_Wheel_Speed_Cons_W34) -> Terminator9/1  "V_BCMA_COM_Wheel_Speed_Cons_W34"
  BCM_COM_PROC_P2_5/5(V_BCM_COM_Wheel_Speed_W34) -> Terminator7/1  "V_BCMA_COM_Wheel_Speed_W34"
  BCM_COM_PROC_P2_5/6(V_BCM_COM_Wheel_Speed_Val_W34) -> Terminator10/1  "V_BCMA_COM_Wheel_Speed_Val_W34"
  BCM_COM_PROC_P2_5/7(V_BCM_COM_Whl_Filt_Spd_For_AS_W12) -> [LG_Whl_Filt_Spd_For_AS]  "V_BCMA_COM_Whl_Filt_Spd_For_AS_W12"
  BCM_COM_PROC_P2_5/8(V_BCM_COM_Wheel_Filtered_Speed_W12) -> [V_BCM_COM_Wheel_Filtered_Speed_W12]  "V_BCMA_COM_Wheel_Filtered_Speed_W12"
  BCM_COM_PROC_P2_5/9(V_BCM_COM_Min_Last_8_Whl_Spd_W12) -> Terminator44/1  "V_BCMA_COM_Min_Last_8_Whl_Spd_W12"
  BCM_COM_PROC_P2_5/10(V_BCM_COM_Max_Last_8_Whl_Spd_W12) -> Terminator45/1  "V_BCMA_COM_Max_Last_8_Whl_Spd_W12"
  BCM_COM_PROC_P2_5/11(V_BCM_COM_Whl_Filt_Spd_For_AS_W34) -> [RG_Whl_Filt_Spd_For_AS]  "V_BCMA_COM_Whl_Filt_Spd_For_AS_W34"
  BCM_COM_PROC_P2_5/12(V_BCM_COM_Wheel_Filtered_Speed_W34) -> [V_BCM_COM_Wheel_Filtered_Speed_W34]  "V_BCMA_COM_Wheel_Filtered_Speed_W34"
  BCM_COM_PROC_P2_5/13(V_BCM_COM_Min_Last_8_Whl_Spd_W34) -> Terminator48/1  "V_BCMA_COM_Min_Last_8_Whl_Spd_W34"
  BCM_COM_PROC_P2_5/14(V_BCM_COM_Max_Last_8_Whl_Spd_W34) -> Terminator49/1  "V_BCMA_COM_Max_Last_8_Whl_Spd_W34"
  [LH_OUT_WHEEL_SPEED] -> Mux/1
  [LH_IN_WHEEL_SPEED] -> Mux/2
  Mux24/1 -> [Tacho_Conf_Flt]
  [Tacho_Conf_Flt] -> Selector/1
  Selector/1 -> BCM_COM_PROC_P2_5/3(V_BCM_COM_Tacho_Conf_Flt_W12)
  [Tacho_Conf_Flt] -> Selector1/1
  Selector1/1 -> BCM_COM_PROC_P2_5/6(V_BCM_COM_Tacho_Conf_Flt_W34)
  [Tacho_Conf_Flt] -> BCM_COM_PROC_P20/1(V_BCM_COM_Tachometers_Conf_Flt)
  [Tacho_Unconf_Flt] -> Selector2/1
  Selector2/1 -> BCM_COM_PROC_P2_5/2(V_BCM_COM_Tacho_Unconf_Flt_W12)
  [Tacho_Unconf_Flt] -> Selector3/1
  Selector3/1 -> BCM_COM_PROC_P2_5/5(V_BCM_COM_Tacho_Unconf_Flt_W34)
  Bus Selector/1 -> [DFCSA_Gnd_Spd]  "<BUS_A429_DFCS1_BCMA_LABEL_206_Ground_Speed>"
  BUS_A429_DFCS3_BCMA/1 -> Bus Selector1/1
  Bus Selector1/1 -> [DFCSB_Gnd_Spd]  "<BUS_A429_DFCS3_BCMA_LABEL_206_Ground_Speed>"
  Bus Selector1/2 -> [DFCSB_LH_Braking_Cmd]  "<BUS_A429_DFCS3_BCMA_LABEL_202_DFCS_LH_Braking_Cmd>"
  Bus Selector1/3 -> [DFCSB_RH_Braking_Cmd]  "<BUS_A429_DFCS3_BCMA_LABEL_202_DFCS_RH_Braking_Cmd>"
  [DFCSA_Gnd_Spd_Val] -> BCM_COM_PROC_P20/4(V_BCM_COM_DFCS_A_Gnd_Spd_Val)
  [DFCSB_Gnd_Spd_Val] -> BCM_COM_PROC_P20/5(V_BCM_COM_DFCS_B_Gnd_Spd_Val)
  Bus Selector/4 -> [DFCSA_Long_Accel]  "<BUS_A429_DFCS1_BCMA_LABEL_205_Longitudinal_Acceleration>"
  Bus Selector1/4 -> [DFCSB_Long_Accel]  "<BUS_A429_DFCS3_BCMA_LABEL_205_Longitudinal_Acceleration>"
  [DFCSA_Long_Accel_Val] -> BCM_COM_PROC_P20/8(V_BCM_COM_DFCS_A_AC_Long_Accel_Val)
  [DFCSB_Long_Accel_Val] -> BCM_COM_PROC_P20/9(V_BCM_COM_DFCS_B_AC_Long_Accel_Val)
  Bus Selector/5 -> [DFCSA_Pitch_Ang]  "<BUS_A429_DFCS1_BCMA_LABEL_207_Pitch_Angle>"
  Bus Selector1/5 -> [DFCSB_Pitch_Ang]  "<BUS_A429_DFCS3_BCMA_LABEL_207_Pitch_Angle>"
  [DFCSB_Pitch_Ang_Val] -> BCM_COM_PROC_P20/13(V_BCM_COM_DFCS_B_AC_Pitch_Angle_Val)
  [DFCSA_Pitch_Ang_Val] -> BCM_COM_PROC_P20/12(V_BCM_COM_DFCS_A_AC_Pitch_Angle_Val)
  Bus Selector/6 -> Mux1/1  "<BUS_A429_DFCS1_BCMA_LABEL_204_DATA_BIT_14_WOW1_Validity>"
  Bus Selector/7 -> Mux1/2  "<BUS_A429_DFCS1_BCMA_LABEL_204_DATA_BIT_18_WOW2_Validity>"
  Bus Selector/8 -> Mux1/3  "<BUS_A429_DFCS1_BCMA_LABEL_204_DATA_BIT_22_WOW3_Validity>"
  Bus Selector/9 -> Mux2/1  "<BUS_A429_DFCS1_BCMA_LABEL_204_DATA_BIT_12_WOW1_LMLG>"
  Bus Selector/10 -> Mux2/2  "<BUS_A429_DFCS1_BCMA_LABEL_204_DATA_BIT_16_WOW2_LMLG>"
  Bus Selector/11 -> Mux2/3  "<BUS_A429_DFCS1_BCMA_LABEL_204_DATA_BIT_20_WOW3_LMLG>"
  Bus Selector/12 -> Mux4/1  "<BUS_A429_DFCS1_BCMA_LABEL_204_DATA_BIT_13_WOW1_RMLG>"
  Bus Selector/13 -> Mux4/2  "<BUS_A429_DFCS1_BCMA_LABEL_204_DATA_BIT_17_WOW2_RMLG>"
  Bus Selector/14 -> Mux4/3  "<BUS_A429_DFCS1_BCMA_LABEL_204_DATA_BIT_21_WOW3_RMLG>"
  Bus Selector/15 -> Mux5/1  "<BUS_A429_DFCS1_BCMA_LABEL_204_DATA_BIT_11_WOW1_NLG>"
  Bus Selector/16 -> Mux5/2  "<BUS_A429_DFCS1_BCMA_LABEL_204_DATA_BIT_15_WOW2_NLG>"
  Bus Selector/17 -> Mux5/3  "<BUS_A429_DFCS1_BCMA_LABEL_204_DATA_BIT_19_WOW3_NLG>"
  Mux1/1 -> [DFCSA_WOWs_Val_Acq]
  [DFCSB_WOWs_Val_Val] -> BCM_COM_PROC_P20/17(V_BCM_COM_DFCS_B_WOWs_Val_Val)
  [DFCSA_WOWs_Val_Val] -> BCM_COM_PROC_P20/16(V_BCM_COM_DFCS_A_WOWs_Val_Val)
  Mux2/1 -> [DFCSA_LMLG_WOWs]
  Mux4/1 -> [DFCSA_RMLG_WOWs]
  Mux5/1 -> [DFCSA_NLG_WOWs]
  DFCSA_RMLG_WOWs_Comp/1(RMLG_WOWs_out) -> BCM_COM_PROC_P20/24(V_BCM_COM_DFCS_A_RMLG_WOWs_Acq)
  DFCSA_NLG_WOWs_Comp/1(NLG_WOWs_out) -> BCM_COM_PROC_P20/28(V_BCM_COM_DFCS_A_NLG_WOWs_Acq)
  Bus Selector1/6 -> Mux11/1  "<BUS_A429_DFCS3_BCMA_LABEL_204_DATA_BIT_14_WOW1_Validity>"
  Bus Selector1/7 -> Mux11/2  "<BUS_A429_DFCS3_BCMA_LABEL_204_DATA_BIT_18_WOW2_Validity>"
  Bus Selector1/8 -> Mux11/3  "<BUS_A429_DFCS3_BCMA_LABEL_204_DATA_BIT_22_WOW3_Validity>"
  Bus Selector1/9 -> Mux12/1  "<BUS_A429_DFCS3_BCMA_LABEL_204_DATA_BIT_12_WOW1_LMLG>"
  Bus Selector1/10 -> Mux12/2  "<BUS_A429_DFCS3_BCMA_LABEL_204_DATA_BIT_16_WOW2_LMLG>"
  Bus Selector1/12 -> Mux13/1  "<BUS_A429_DFCS3_BCMA_LABEL_204_DATA_BIT_13_WOW1_RMLG>"
  Bus Selector1/11 -> Mux12/3  "<BUS_A429_DFCS3_BCMA_LABEL_204_DATA_BIT_20_WOW3_LMLG>"
  Bus Selector1/13 -> Mux13/2  "<BUS_A429_DFCS3_BCMA_LABEL_204_DATA_BIT_17_WOW2_RMLG>"
  Bus Selector1/14 -> Mux13/3  "<BUS_A429_DFCS3_BCMA_LABEL_204_DATA_BIT_21_WOW3_RMLG>"
  Bus Selector1/15 -> Mux14/1  "<BUS_A429_DFCS3_BCMA_LABEL_204_DATA_BIT_11_WOW1_NLG>"
  Bus Selector1/16 -> Mux14/2  "<BUS_A429_DFCS3_BCMA_LABEL_204_DATA_BIT_15_WOW2_NLG>"
  Bus Selector1/17 -> Mux14/3  "<BUS_A429_DFCS3_BCMA_LABEL_204_DATA_BIT_19_WOW3_NLG>"
  Mux11/1 -> [DFCSB_WOWs_Val_Acq]
  Mux12/1 -> [DFCSB_LMLG_WOWs]
  Mux13/1 -> [DFCSB_RMLG_WOWs]
  Mux14/1 -> [DFCSB_NLG_WOWs]
  DFCSB_LMLG_WOWs_Comp/1(LMLG_WOWs_out) -> BCM_COM_PROC_P20/21(V_BCM_COM_DFCS_B_LMLG_WOWs_Acq)
  DFCSB_RMLG_WOWs_Comp/1(RMLG_WOWs_out) -> BCM_COM_PROC_P20/25(V_BCM_COM_DFCS_B_RMLG_WOWs_Acq)
  DFCSB_NLG_WOWs_Comp/1(NLG_WOWs_out) -> BCM_COM_PROC_P20/29(V_BCM_COM_DFCS_B_NLG_WOWs_Acq)
  [DFCSA_LMLG_WOWs_Val] -> BCM_COM_PROC_P20/18(V_BCM_COM_DFCS_A_LMLG_WOWs_Val)  "DFCSA_LMLG_WOWs_Val"
  [DFCSB_LMLG_WOWs_Val] -> BCM_COM_PROC_P20/19(V_BCM_COM_DFCS_B_LMLG_WOWs_Val)
  [DFCSA_RMLG_WOWs_Val] -> BCM_COM_PROC_P20/22(V_BCM_COM_DFCS_A_RMLG_WOWs_Val)
  [DFCSB_RMLG_WOWs_Val] -> BCM_COM_PROC_P20/23(V_BCM_COM_DFCS_B_RMLG_WOWs_Val)
  [DFCSA_NLG_WOWs_Val] -> BCM_COM_PROC_P20/26(V_BCM_COM_DFCS_A_NLG_WOWs_Val)
  [DFCSB_NLG_WOWs_Val] -> BCM_COM_PROC_P20/27(V_BCM_COM_DFCS_B_NLG_WOWs_Val)
  [V_BCM_COM_RH_Decel_Law_Brkg_Press_Cmd] -> BCM_COM_PROC_P20/30(V_BCM_COM_RH_Decel_Law_Brkg_Press_Cmd)
  [V_BCM_COM_LH_Decel_Law_Brkg_Press_Cmd] -> BCM_COM_PROC_P20/31(V_BCM_COM_LH_Decel_Law_Brkg_Press_Cmd)
  [DFCSA_LH_Braking_Cmd_Val] -> BCM_COM_PROC_P20/34(V_BCM_COM_DFCS_A_LH_Braking_Cmd_Val)
  [DFCSA_RH_Braking_Cmd_Val] -> BCM_COM_PROC_P20/35(V_BCM_COM_DFCS_A_RH_Braking_Cmd_Val)
  [DFCSB_LH_Braking_Cmd_Val] -> BCM_COM_PROC_P20/36(V_BCM_COM_DFCS_B_LH_Braking_Cmd_Val)
  [DFCSB_RH_Braking_Cmd_Val] -> BCM_COM_PROC_P20/37(V_BCM_COM_DFCS_B_RH_Braking_Cmd_Val)
  DFCSB_LH_Braking_Cmd_Comp/1(Braking_Cmd_out) -> BCM_COM_PROC_P20/40(V_BCM_COM_DFCS_B_DFCS_LH_Braking_Cmd_Acq)
  DFCSB_RH_Braking_Cmd_Comp/1(Braking_Cmd_out) -> BCM_COM_PROC_P20/41(V_BCM_COM_DFCS_B_DFCS_RH_Braking_Cmd_Acq)
  Bus Selector/18 -> [DFCSA_DCL_Inhibition]  "<BUS_A429_DFCS1_BCMA_LABEL_204_DATA_BIT_24_Decel_Law_Inhibition>"
  Bus Selector/19 -> [DFCSA_TLA_Above_Idle]  "<BUS_A429_DFCS1_BCMA_LABEL_204_DATA_BIT_27_TLA_Above_Idle>"
  Bus Selector1/19 -> [DFCSB_TLA_Above_Idle]  "<BUS_A429_DFCS3_BCMA_LABEL_204_DATA_BIT_27_TLA_Above_Idle>"
  Bus Selector1/18 -> [DFCSB_DCL_Inhibition]  "<BUS_A429_DFCS3_BCMA_LABEL_204_DATA_BIT_24_Decel_Law_Inhibition>"
  DFCSB_DCL_Inhibition_Comp/1(DCL_Inhibition_out) -> BCM_COM_PROC_P20/45(V_BCM_COM_DFCS_B_Decel_Law_Inhib_Acq)
  [DFCSA_DCL_Inhibition_Val] -> BCM_COM_PROC_P20/42(V_BCM_COM_DFCS_A_Decel_Law_Inhib_Val)
  [DFCSB_DCL_Inhibition_Val] -> BCM_COM_PROC_P20/44(V_BCM_COM_DFCS_B_Decel_Law_Inhib_Val)
  [DFCSB_TLA_Above_Idle_Val] -> BCM_COM_PROC_P20/47(V_BCM_COM_DFCS_B_TLA_Above_Idle_Val)
  [DFCSA_TLA_Above_Idle_Val] -> BCM_COM_PROC_P20/46(V_BCM_COM_DFCS_A_TLA_Above_Idle_Val)
  [LG_Lever_Up] -> BCM_COM_PROC_P20/50(V_BCM_COM_LG_Lever_Up_Acq)
  Constant38/1 -> [LG_Lever_Up_Unconf_Flt]
  Constant39/1 -> [LG_Lever_Up_Conf_Flt]
  [LG_Lever_Up_Unconf_Flt] -> BCM_COM_PROC_P20/51(V_BCM_COM_LG_Lever_Up_Unconf_Flt)
  [LG_Lever_Up_Conf_Flt] -> BCM_COM_PROC_P20/52(V_BCM_COM_LG_Lever_Up_Conf_Flt)
  [LMLG_Downlock] -> BCM_COM_PROC_P20/53(V_BCM_COM_LMLG_Downlock_Acq)
  [RMLG_Downlock] -> BCM_COM_PROC_P20/54(V_BCM_COM_RMLG_Downlock_Acq)
  Constant41/1 -> [LMLG_Downlock_Conf_Flt]
  Constant40/1 -> [LMLG_Downlock_Unconf_Flt]
  Constant42/1 -> [RMLG_Downlock_Unconf_Flt]
  Constant43/1 -> [RMLG_Downlock_Conf_Flt]
  [LMLG_Downlock_Unconf_Flt] -> BCM_COM_PROC_P20/55(V_BCM_COM_LMLG_Dnlk_Unconf_Flt)
  [LMLG_Downlock_Conf_Flt] -> BCM_COM_PROC_P20/56(V_BCM_COM_LMLG_Dnlk_Conf_Flt)
  [RMLG_Downlock_Unconf_Flt] -> BCM_COM_PROC_P20/57(V_BCM_COM_RMLG_Dnlk_Unconf_Flt)
  [RMLG_Downlock_Conf_Flt] -> BCM_COM_PROC_P20/58(V_BCM_COM_RMLG_Dnlk_Conf_Flt)
  Bus Selector2/1 -> Mux15/1  "<BUS_A429_GenIO_1A_GPHS_LABEL_272_ENG1_Engine_Running>"
  Bus Selector2/2 -> Mux15/2  "<BUS_A429_GenIO_1A_GPHS_LABEL_273_ENG2_Engine_Running>"
  [Engine_Running] -> BCM_COM_PROC_P20/59(V_BCM_COM_Engine_Running_Acq)
  Bus Selector2/3 -> [Hyd_A_Press]  "<BUS_A429_GenIO_1A_GPHS_LABEL_022_HCM_SYS_A_PRESSURE>"
  [PBSELV_ON_POS] -> BCM_COM_PROC_P20/60(V_BCM_COM_PBSELV_ON_POS_Acq)
  [Maint_Itv_Function_Req] -> BCM_COM_PROC_P20/63(V_BCM_COM_Maint_Itv_Function_Req)
  [BCM_Config] -> BCM_COM_PROC_P20/64(V_BCM_COM_BCM_Config)
  Constant52/1 -> [Maint_Itv_Function_Req]
  BCM Config Computation/1(BCM_Config) -> [BCM_Config]  "BCMA_Config"
  Mux15/1 -> [Engine_Running]
  Constant16/1 -> Mux24/1
  Constant54/1 -> Mux24/2
  Constant72/1 -> Mux24/3
  Constant73/1 -> Mux24/4
  Constant76/1 -> Mux25/4
  Constant75/1 -> Mux25/3
  Constant74/1 -> Mux25/2
  Constant2/1 -> Mux25/1
  Mux25/1 -> [Tacho_Unconf_Flt]
  Bus Selector/2 -> Inadvertent Braking Order Failure Mode/1(DFCSA_LH_Braking_Cmd_in)  "<BUS_A429_DFCS1_BCMA_LABEL_202_DFCS_LH_Braking_Cmd>"
  Bus Selector/3 -> Inadvertent Braking Order Failure Mode/2(DFCSA_RH_Braking_Cmd_in)  "<BUS_A429_DFCS1_BCMA_LABEL_202_DFCS_RH_Braking_Cmd>"
  [BCM_Tuning] -> BCM_COM_PROC_P2_5/12(BCM_Tuning)
  [BCM_Tuning] -> BCM_COM_PROC_P20/213(BCM_Tuning)
  [BCM_Config] -> Tuning Management/6(BCM_Config)
  Tuning Management/1(BCM_Tuning) -> [BCM_Tuning]
  [BCM_Tuning] -> BCM_COM_PROC_P5/35(BCM_Tuning)
  Constant25/1 -> [BCM_Off_Sanction]
  [BCM_Off_Sanction] -> BCM_COM_PROC_P20/65(V_BCM_COM_BCM_Off_Sanction)
  [BCM_Validity_By_SP] -> BCM_COM_PROC_P20/66(V_BCM_COM_BCM_Validity_By_SP)
  [BCP_ALT_SW_ON_CMD] -> BCM_COM_PROC_P20/67(V_BCM_COM_BCP_BCM_Alt_Sw_On_Cmd_Acq)
  Constant46/1 -> [BCP_ALT_SW_ON_CMD_Conf_Flt]
  Constant29/1 -> [BCP_ALT_SW_ON_CMD_Unconf_Flt]
  [BCP_ALT_SW_ON_CMD_Unconf_Flt] -> BCM_COM_PROC_P20/69(V_BCM_COM_BCP_BCM_Alt_Sw_On_Cmd_Unconf_Flt)
  [BCP_ALT_SW_ON_CMD_Conf_Flt] -> BCM_COM_PROC_P20/68(V_BCM_COM_BCP_BCM_Alt_Sw_On_Cmd_Conf_Flt)
  Constant47/1 -> [BCP_ALT_SW_Disp_Sw_Unconf_Flt]
  Constant48/1 -> [BCP_ALT_SW_Disp_Sw_Conf_Flt]
  [BCP_ALT_SW_Disp_Sw_Unconf_Flt] -> BCM_COM_PROC_P20/71(V_BCM_COM_MP_BCMA_Alt_Disp_Sw_Unconf_Flt)
  [BCP_ALT_SW_Disp_Sw_Conf_Flt] -> BCM_COM_PROC_P20/70(V_BCM_COM_MP_BCMA_Alt_Disp_Sw_Conf_Flt)
  Constant/1 -> BCM_COM_PROC_P20/72(V_BCM_COM_MP_BCMA_Alt_Disp_Sw_Acq)
  Constant50/1 -> [Antiskid_Off_Sanction]
  [Antiskid_Off_Sanction] -> BCM_COM_PROC_P20/73(V_BCM_COM_Antiskid_Off_Sanction)
  Constant51/1 -> [Norm_Brk_Off_Sanction]
  [Norm_Brk_Off_Sanction] -> BCM_COM_PROC_P20/74(V_BCM_COM_Norm_Brkg_Off_Sanc)
  Constant80/1 -> [LH_ALT_BRK_LOSS]
  [LH_ALT_BRK_LOSS] -> BCM_COM_PROC_P20/75(V_BCM_COM_CF_LH_ALT_BRK_LOSS)
  [RH_ALT_BRK_LOSS] -> BCM_COM_PROC_P20/77(V_BCM_COM_CF_RH_ALT_BRK_LOSS)
  Constant81/1 -> [RH_ALT_BRK_LOSS]
  Ground/1 -> BCM_COM_PROC_P20/76(V_BCM_COM_CF_DBCU_FAILED)
  BCM_COM_PROC_P5/6(V_BCM_COM_SV_PT_Filt) -> [V_BCM_COM_SV_PT_Filt]  "V_BCMA_COM_SV_PT_Filt"
  [V_BCM_COM_SV_PT_Filt] -> BCM_COM_PROC_P20/78(V_BCM_COM_SV_PT_Filt)
  Constant83/1 -> [PBSELV_ON_POS_Conf_Flt]
  Constant82/1 -> [PBSELV_ON_POS_Unconf_Flt]
  [PBSELV_ON_POS_Unconf_Flt] -> BCM_COM_PROC_P20/61(V_BCM_COM_PBSELV_ON_POS_Unconf_Flt)
  [PBSELV_ON_POS_Conf_Flt] -> BCM_COM_PROC_P20/62(V_BCM_COM_PBSELV_ON_POS_Conf_Flt)
  Bus Selector2/4 -> [Hyd_B_Press]  "<BUS_A429_GenIO_1A_GPHS_LABEL_021_HCM_SYS_B_PRESSURE>"
  [LHSV_PT_PRESSURE] -> BCM_COM_PROC_P5/1(V_BCM_COM_LH_SV_PT_Acq)
  [RHSV_PT_PRESSURE] -> BCM_COM_PROC_P5/2(V_BCM_COM_RH_SV_PT_Acq)
  Constant88/1 -> [LH_SV_PT_Unconf_Flt]
  Constant90/1 -> [RH_SV_PT_Unconf_Flt]
  [LH_SV_PT_Unconf_Flt] -> BCM_COM_PROC_P5/3(V_BCM_COM_LH_SV_PT_Unconf_Flt)
  [LH_SV_PT_Conf_Flt] -> BCM_COM_PROC_P5/5(V_BCM_COM_LH_SV_PT_Conf_Flt)
  [RH_SV_PT_Unconf_Flt] -> BCM_COM_PROC_P5/4(V_BCM_COM_RH_SV_PT_Unconf_Flt)
  [RH_SV_PT_Conf_Flt] -> BCM_COM_PROC_P5/6(V_BCM_COM_RH_SV_PT_Conf_Flt)
  [BCM_Config] -> BCM_COM_PROC_P5/7(V_BCM_COM_BCM_Config)
  [Brkg_On_Wheels] -> Unit Delay7/1
  [SELV_High_Side_Cmd_Order] -> Unit Delay1/1
  [Press_Cmd_Rate_Lim] -> Unit Delay/1
  [PBSELV_State_Cons] -> Unit Delay2/1
  [Braking_State] -> Unit Delay3/1
  [LH_Press_Reg_FT_Act_Cond] -> Unit Delay4/1
  [RH_Press_Reg_FT_Act_Cond] -> Unit Delay5/1
  [Braking_Mode] -> Unit Delay6/1
  BCM_COM_PROC_P5/1(V_BCM_COM_SV_PT_Cons) -> [V_BCM_COM_SV_PT_Cons]  "V_BCMA_COM_SV_PT_Cons"
  BCM_COM_PROC_P5/2(V_BCM_COM_SV_PT_Cons_Val) -> [V_BCM_COM_SV_PT_Cons_Val]  "V_BCMA_COM_SV_PT_Cons_Val"
  BCM_COM_PROC_P5/4(V_BCM_COM_SV_Curr_AS_Protect) -> Terminator81/1  "V_BCMA_COM_SV_Curr_AS_Protect"
  BCM_COM_PROC_P5/5(V_BCM_COM_SV_Current_Order) -> [V_BCM_COM_SV_Current_Order]  "V_BCMA_COM_SV_Current_Order"
  BCM_COM_PROC_P5/3(V_BCM_COM_SV_Current) -> [V_BCM_COM_SV_Current]  "V_BCMA_COM_SV_Current"
  [V_BCM_COM_SV_Current_Order] -> Demux/1
  BCM_COM_PROC_P5/7(V_BCM_COM_Corr_Press_Cmd) -> Terminator97/1  "V_BCMA_COM_Corr_Press_Cmd"
  BCM_COM_PROC_P5/8(V_BCM_COM_SV_Drift) -> Terminator103/1  "V_BCMA_COM_SV_Drift"
  BCM_COM_PROC_P5/9(V_BCM_COM_PCL_State) -> Terminator111/1  "V_BCMA_COM_PCL_State"
  BCM_COM_PROC_P5/10(V_BCM_COM_Whl_AS_Activity) -> [V_BCM_COM_Whl_AS_Activity]  "V_BCMA_COM_Whl_AS_Activity"
  BCM_COM_PROC_P5/11(V_BCM_COM_Press_Reg_Act_Cond) -> Terminator122/1  "V_BCMA_COM_Press_Reg_Act_Cond"
  Unit Delay/1 -> BCM_COM_PROC_P5/9(V_BCM_COM_Press_Cmd_Rate_Lim)
  Unit Delay1/1 -> BCM_COM_PROC_P5/10(V_BCM_COM_SELV_High_Side_Cmd_Order)
  Unit Delay2/1 -> BCM_COM_PROC_P5/11(V_BCM_COM_PBSELV_State_Cons)
  Unit Delay3/1 -> BCM_COM_PROC_P5/12(V_BCM_COM_Braking_State)
  Unit Delay4/1 -> BCM_COM_PROC_P5/13(V_BCM_COM_LH_Press_Reg_FT_Act_Cond)
  Unit Delay5/1 -> BCM_COM_PROC_P5/14(V_BCM_COM_RH_Press_Reg_FT_Act_Cond)
  Unit Delay6/1 -> BCM_COM_PROC_P5/15(V_BCM_COM_Braking_Mode)
  Unit Delay7/1 -> BCM_COM_PROC_P5/8(V_BCM_COM_Brkg_On_Wheels)
  [Hyd_A_Press] -> BCM_COM_PROC_P20/32(V_BCM_COM_Hyd_A_Press_Acq)
  [Hyd_B_Press] -> BCM_COM_PROC_P20/33(V_BCM_COM_Hyd_B_Press_Acq)
  [V_BCM_COM_A429_LH_Brkg_Cmd_Fdbk] -> BUS_A429_BCMA_DFCS13_TX/1(BCMCP_LH_Braking_Cmd_Feedback)
  [V_BCM_COM_A429_RH_Brkg_Cmd_Fdbk] -> BUS_A429_BCMA_DFCS13_TX/2(BCMCP_RH_Braking_Cmd_Feedback)
  [V_BCM_COM_A429_Wheel_Speed_W34] -> Selector5/1, Selector7/1
  [V_BCM_COM_A429_Wheel_Speed_W12] -> Selector4/1, Selector6/1
  Demux3/1 -> BUS_A429_BCMA_DFCS13_TX/15(BCMCP_LH_Brake_Pressure)
  Demux3/2 -> BUS_A429_BCMA_DFCS13_TX/16(BCMCP_RH_Brake_Pressure)
  [CP_Inadvertent_Braking_Order_Acquisition] -> Inadvertent Braking Order Failure Mode/3(CP_Inadvertent_Braking_Order_Acquisition)
  Inadvertent Braking Order Failure Mode/2(DFCSA_RH_Braking_Cmd) -> [DFCSA_RH_Braking_Cmd]
  Inadvertent Braking Order Failure Mode/1(DFCSA_LH_Braking_Cmd) -> [DFCSA_LH_Braking_Cmd]
  Left Inner Wheel Speed Failure Modes/1(LH_IN_WHEEL_SPEED) -> [LH_IN_WHEEL_SPEED]
  LH_IN_WHEEL_SPEED_COIL1/1 -> Left Inner Wheel Speed Failure Modes/1(LH_IN_WHEEL_SPEED_in)
  LH_OUT_WHEEL_SPEED_COIL1/1 -> Left Outer Wheel Speed Failure Modes/1(LH_OUT_WHEEL_SPEED_in)
  Left Outer Wheel Speed Failure Modes/1(LH_OUT_WHEEL_SPEED) -> [LH_OUT_WHEEL_SPEED]
  RH_OUT_WHEEL_SPEED_COIL1/1 -> Right Outer Wheel Speed Failure Modes/1(RH_OUT_WHEEL_SPEED_in)
  RH_IN_WHEEL_SPEED_COIL1/1 -> Right Inner Wheel Speed Failure Modes/1(RH_IN_WHEEL_SPEED_in)
  Right Inner Wheel Speed Failure Modes/1(RH_IN_WHEEL_SPEED) -> [RH_IN_WHEEL_SPEED]
  [WheelSpeed1_Erroneous_Acquisition] -> Left Outer Wheel Speed Failure Modes/2(Wheel_Speed_1_Erroneous_Acquisition)
  [WheelSpeed2_Erroneous_Acquisition] -> Left Inner Wheel Speed Failure Modes/2(Wheel_Speed_2_Erroneous_Acquisition)
  [WheelSpeed3_Erroneous_Acquisition] -> Right Inner Wheel Speed Failure Modes/2(Wheel_Speed_3_Erroneous_Acquisition)
  [WheelSpeed4_Erroneous_Acquisition] -> Right Outer Wheel Speed Failure Modes/2(Wheel_Speed_4_Erroneous_Acquisition)
  Right Outer Wheel Speed Failure Modes/1(RH_OUT_WHEEL_SPEED) -> [RH_OUT_WHEEL_SPEED]
  [WheelSpeed2_Loss] -> Left Inner Wheel Speed Failure Modes/3(Wheel_Speed_2_Loss)
  [WheelSpeed1_Loss] -> Left Outer Wheel Speed Failure Modes/3(Wheel_Speed_1_Loss)
  [WheelSpeed3_Loss] -> Right Inner Wheel Speed Failure Modes/3(Wheel_Speed_3_Loss)
  [WheelSpeed4_Loss] -> Right Outer Wheel Speed Failure Modes/3(Wheel_Speed_4_Loss)
  LH_HASV_PT_PRESSURE/1 -> Left Pressure Transducer Failure Mode/1(LH_PT_PRESSURE_in)
  Left Pressure Transducer Failure Mode/1(LH_PT_PRESSURE) -> [LHSV_PT_PRESSURE]
  Right Pressure Transducer Failure Mode/1(RH_PT_PRESSURE) -> [RHSV_PT_PRESSURE]
  RH_HASV_PT_PRESSURE/1 -> Right Pressure Transducer Failure Mode/1(RH_PT_PRESSURE_in)
  [LHPT_Erroneous_Acquisition] -> Left Pressure Transducer Failure Mode/2(LH_PT_Erroneous_Acquisition)
  [RHPT_Erroneous_Acquisition] -> Right Pressure Transducer Failure Mode/2(RH_PT_Erroneous_Acquisition)
  [CP_Inadvertent_Braking_Order_BSELV_DBSMA] -> Inadvertent Braking Order BSELV Failure Mode/2(CP_Inadvertent_Braking_Order_BSELV_DBSMA)
  Inadvertent Braking Order BSELV Failure Mode/1(HASELV_CMD) -> HASELV_CMD/1
  [SELV_High_Side_Cmd_Order] -> Inadvertent Braking Order BSELV Failure Mode/1(SELV_High_Side_Cmd_Order)
  Demux/2 -> Inadvertent Braking Order DBSMA Failure Mode/2(RH_HASV_CURRENT_in)
  Demux/1 -> Inadvertent Braking Order DBSMA Failure Mode/1(LH_HASV_CURRENT_in)
  Inadvertent Braking Order DBSMA Failure Mode/2(RH_HASV_CURRENT) -> RH_HASV_CURRENT/1
  Inadvertent Braking Order DBSMA Failure Mode/1(LH_HASV_CURRENT) -> LH_HASV_CURRENT/1
  [CP_Inadvertent_Braking_Order_BSELV_DBSMA] -> Inadvertent Braking Order DBSMA Failure Mode/3(CP_Inadvertent_Braking_Order_BSELV_DBSMA)
  [CP_Erroneous_Current_LH] -> Inadvertent Braking Order DBSMA Failure Mode/4(CP_Erroneous_Current_To_LH)
  [CP_Erroneous_Current_RH] -> Inadvertent Braking Order DBSMA Failure Mode/5(CP_Erroneous_Current_To_RH)
  DBCU Inhibition Failure Mode/1(DBCU_INHIBITION) -> BCMA_DBCU_INHIBITION/1
  [DBCU_Inhib_Order] -> DBCU Inhibition Failure Mode/1(DBCU_Inhib_Order)
  [Erroneous_DBCU_Activation_Off] -> DBCU Inhibition Failure Mode/2(Erroneous_DBCU_Activation_Off)
  [Erroneous_DBCU_Activation_On] -> DBCU Inhibition Failure Mode/3(Erroneous_DBCU_Activation_On)
  Selector4/1 -> Left Inner Wheel Speed Emission Failure Mode/1(LHI_Wheel_Speed_in)
  Left Inner Wheel Speed Emission Failure Mode/1(LHI_Wheel_Speed) -> Terminator/1
  Selector6/1 -> Left Outer Wheel Speed Emission Failure Mode/1(LHO_Wheel_Speed_in)
  Left Outer Wheel Speed Emission Failure Mode/1(LHO_Wheel_Speed) -> Terminator1/1
  Selector5/1 -> Right Inner Wheel Speed Emission Failure Mode/1(RHI_Wheel_Speed_in)
  Selector7/1 -> Right Outer Wheel Speed Emission Failure Mode/1(RHO_Wheel_Speed_in)
  Right Inner Wheel Speed Emission Failure Mode/1(RHI_Wheel_Speed) -> Terminator11/1
  Right Outer Wheel Speed Emission Failure Mode/1(RHO_Wheel_Speed) -> Terminator12/1
  [WheelSpeed3_Erroneous_Emission] -> Right Inner Wheel Speed Emission Failure Mode/2(Wheel_Speed_3_Erroneous_Emission)
  [WheelSpeed4_Erroneous_Emission] -> Right Outer Wheel Speed Emission Failure Mode/2(Wheel_Speed_4_Erroneous_Emission)
  [WheelSpeed2_Erroneous_Emission] -> Left Inner Wheel Speed Emission Failure Mode/2(Wheel_Speed_2_Erroneous_Emission)
  [WheelSpeed1_Erroneous_Emission] -> Left Outer Wheel Speed Emission Failure Mode/2(Wheel_Speed_1_Erroneous_Emission)
  [V_BCM_COM_A429_SV_PT_In_PSI] -> Demux3/1
  Demux4/1 -> BUS_A429_BCMA_GenIO_2_TX/1(BCMCP_LH_outboard_wheel_speed)
  Demux4/2 -> BUS_A429_BCMA_GenIO_2_TX/2(BCMCP_LH_inboard_wheel_speed)
  Demux12/1 -> BUS_A429_BCMA_GenIO_2_TX/6(BCMCP_LH_outboard_tacho_fail)
  Demux12/2 -> BUS_A429_BCMA_GenIO_2_TX/7(BCMCP_LH_inboard_tacho_fail)
  Demux13/1 -> BUS_A429_BCMA_GenIO_2_TX/8(BCMCP_RH_inboard_tacho_fail)
  Demux13/2 -> BUS_A429_BCMA_GenIO_2_TX/9(BCMCP_RH_outboard_tacho_fail)
  [V_BCM_COM_A429_LH_Brake_Temp_Sensor_Fail] -> BUS_A429_BCMA_GenIO_2_TX/10(BCMCP_LH_outboard_brake_temp_sensor_fail)
  [V_BCM_COM_A429_RH_Brake_Temp_Sensor_Fail] -> BUS_A429_BCMA_GenIO_2_TX/11(BCMCP_RH_outboard_brake_temp_sensor_fail)
  [V_BCM_COM_A429_LNLG_Tire_Press_Sensor_Fail] -> BUS_A429_BCMA_GenIO_2_TX/12(BCMCP_left_nose_tire_press_sensor_fail)
  [V_BCM_COM_A429_RNLG_Tire_Press_Sensor_Fail] -> BUS_A429_BCMA_GenIO_2_TX/13(BCMCP_right_nose_tire_press_sensor_fail)
  [V_BCM_COM_A429_LMLG_Tire_Press_Sensor_Fail_W1] -> BUS_A429_BCMA_GenIO_2_TX/14(BCMCP_LH_outboard_tire_press_sensor_fail)
  [V_BCM_COM_A429_LMLG_Tire_Press_Sensor_Fail_W2] -> BUS_A429_BCMA_GenIO_2_TX/15(BCMCP_LH_inboard_tire_press_sensor_fail)
  [V_BCM_COM_A429_RMLG_Tire_Press_Sensor_Fail_W3] -> BUS_A429_BCMA_GenIO_2_TX/16(BCMCP_RH_inboard_tire_press_sensor_fail)
  [V_BCM_COM_A429_RMLG_Tire_Press_Sensor_Fail_W4] -> BUS_A429_BCMA_GenIO_2_TX/17(BCMCP_RH_outboard_tire_press_sensor_fail)
  [V_BCM_COM_A429_TPIS_Fail] -> BUS_A429_BCMA_GenIO_2_TX/18(BCMCP_TPIS_fail)
  [V_BCM_COM_LNLG_Tire_Press] -> BUS_A429_BCMA_GenIO_2_TX/21(LNLG_tire_press)
  [V_BCM_COM_RNLG_Tire_Press] -> BUS_A429_BCMA_GenIO_2_TX/22(RNLG_tire_press)
  [V_BCM_COM_LMLG_Tire_Press_W1] -> BUS_A429_BCMA_GenIO_2_TX/23(LMLG_outboard_tire_press)
  [V_BCM_COM_LMLG_Tire_Press_W2] -> BUS_A429_BCMA_GenIO_2_TX/24(LMLG_inboard_tire_press)
  [V_BCM_COM_RMLG_Tire_Press_W3] -> BUS_A429_BCMA_GenIO_2_TX/25(RMLG_inboard_tire_press)
  [V_BCM_COM_RMLG_Tire_Press_W4] -> BUS_A429_BCMA_GenIO_2_TX/26(RMLG_outboard_tire_press)
  [V_BCM_COM_A429_ACCU_PT] -> BUS_A429_BCMA_GenIO_2_TX/27(BCMCP_accu_press)
  [V_BCM_COM_A429_ACCU_PT_Fail] -> BUS_A429_BCMA_GenIO_2_TX/28(BCMCP_Accu_PT_fail)
  Demux15/1 -> BUS_A429_BCMA_GenIO_2_TX/29(BCMCP_LH_SV_fail)
  Demux15/2 -> BUS_A429_BCMA_GenIO_2_TX/30(BCMCP_RH_SV_fail)
  Demux16/1 -> BUS_A429_BCMA_GenIO_2_TX/31(BCMCP_LH_SVPT_fail)
  Demux16/2 -> BUS_A429_BCMA_GenIO_2_TX/32(BCMCP_RH_SVPT_fail)
  [V_BCM_COM_A429_SELV_Fail] -> BUS_A429_BCMA_GenIO_2_TX/33(BCMCP_SELV_fail)
  [V_BCM_COM_A429_Park_Brake_Fail] -> BUS_A429_BCMA_GenIO_2_TX/35(BCMCP_park_brake_fail)
  [V_BCM_COM_A429_SELV_Disc_Sts_Rdbk] -> BUS_A429_BCMA_GenIO_2_TX/37(BCMCP_SELV_discrete_status_readback)
  [V_BCM_COM_A429_SELV_Disc_Sts_Rdbk_Val] -> BUS_A429_BCMA_GenIO_2_TX/38(BCMCP_SELV_discrete_status_readback_validity)
  [V_BCM_COM_A429_Brk_Residual_Press] -> BUS_A429_BCMA_GenIO_2_TX/39(BCMCP_brake_residual_press)
  [V_BCM_COM_A429_PP_Channel_ID] -> Data Type Conversion38/1
  [V_BCM_COM_A429_Pinprog_4] -> BUS_A429_BCMA_GenIO_2_TX/53(BCMCP_pinprog_4)
  [V_BCM_COM_A429_Pinprog_5] -> BUS_A429_BCMA_GenIO_2_TX/54(BCMCP_pinprog_5)
  [V_BCM_COM_A429_Maint_Mode_Active] -> BUS_A429_BCMA_GenIO_2_TX/56(BCMCP_maintenance_mode_active)
  [V_BCM_COM_A429_Maint_Mode_Req_GND] -> BUS_A429_BCMA_GenIO_2_TX/57(BCMCP_maintenance_mode_request_GND)
  [V_BCM_COM_A429_LH_Brk_Pdl_Ord_Fail] -> BUS_A429_BCMA_GenIO_2_TX/63(BCMCP_DFCS_LH_brake_pedal_order_fail)
  [V_BCM_COM_A429_RH_Brk_Pdl_Ord_Fail] -> BUS_A429_BCMA_GenIO_2_TX/64(BCMCP_DFCS_RH_brake_pedal_order_fail)
  [V_BCM_COM_A429_DFCS_A_Comm_Fail_RX] -> BUS_A429_BCMA_GenIO_2_TX/65(BCMCP_DFCS1_comm_fail_RX)
  [V_BCM_COM_A429_DFCS_B_Comm_Fail_RX] -> BUS_A429_BCMA_GenIO_2_TX/66(BCMCP_DFCS2_comm_fail_RX)
  [V_BCM_COM_A429_Avionics_Comm_Fail_RX] -> BUS_A429_BCMA_GenIO_2_TX/67(BCMCP_Avionics_comm_fail_RX)
  [V_BCM_COM_A429_Norm_Brake_Fail] -> BUS_A429_BCMA_GenIO_2_TX/73(BCMCP_normal_brake_fail)
  [V_BCM_COM_A429_Alternate_Fail] -> BUS_A429_BCMA_GenIO_2_TX/75(BCMCP_alternate_fail)
  [V_BCM_COM_A429_DBCU_Fail] -> BUS_A429_BCMA_GenIO_2_TX/76(BCMCP_DBCU_fail)
  [V_BCM_COM_A429_DBCU_Dispatch_Conf] -> BUS_A429_BCMA_GenIO_2_TX/77(BCMCP_DBCU_dispatch_conf)
  [V_BCM_COM_A429_PLT_Not_Performed] -> BUS_A429_BCMA_GenIO_2_TX/78(BCMCP_PLT_not_performed)
  [V_BCM_COM_Whl_LP_AS_Curr_Order_W12] -> Unit Delay31/1
  BCM_COM_PROC_P5/12(V_BCM_COM_Whl_LP_AS_Curr_Order_W12) -> [V_BCM_COM_Whl_LP_AS_Curr_Order_W12]  "V_BCMA_COM_Whl_LP_AS_Curr_Order_W12"
  [Press_Cmd_Rate_Lim] -> Unit Delay32/1
  BCM_COM_PROC_P5/13(V_BCM_COM_Whl_LP_AS_Curr_Order_W34) -> [V_BCM_COM_Whl_LP_AS_Curr_Order_W34]  "V_BCMA_COM_Whl_LP_AS_Curr_Order_W34"
  [V_BCM_COM_Whl_LP_AS_Curr_Order_W34] -> Unit Delay33/1
  [V_BCM_COM_AC_State] -> Unit Delay8/1
  [V_BCM_COM_AC_Flight_Phase] -> Unit Delay9/1
  [LG_Whl_Filt_Spd_For_AS] -> BCM_COM_PROC_P5/16(V_BCM_COM_Whl_Filt_Spd_For_AS_W12)
  [RG_Whl_Filt_Spd_For_AS] -> BCM_COM_PROC_P5/17(V_BCM_COM_Whl_Filt_Spd_For_AS_W34)
  [V_BCM_COM_Wheel_Control_Speed_W12] -> Unit Delay10/1
  [V_BCM_COM_Wheel_Control_Speed_W34] -> Unit Delay11/1
  Unit Delay9/1 -> BCM_COM_PROC_P5/21(V_BCM_COM_AC_Flight_Phase)
  Unit Delay10/1 -> BCM_COM_PROC_P5/24(V_BCM_COM_Wheel_Control_Speed_W12)
  Unit Delay11/1 -> BCM_COM_PROC_P5/25(V_BCM_COM_Wheel_Control_Speed_W34)
  [V_BCM_COM_Whl_AS_Adp_Gain_W34] -> Unit Delay13/1
  [V_BCM_COM_Whl_AS_Adp_Gain_W12] -> Unit Delay12/1
  Unit Delay12/1 -> BCM_COM_PROC_P5/26(V_BCM_COM_Whl_AS_Adp_Gain_W12)
  Unit Delay13/1 -> BCM_COM_PROC_P5/27(V_BCM_COM_Whl_AS_Adp_Gain_W34)
  BCM_COM_PROC_P5/14(V_BCM_COM_Whl_AS_Inhib_Cond_W12) -> [V_BCM_COM_Whl_AS_Inhib_Cond_W12]  "V_BCMA_COM_Whl_AS_Inhib_Cond_W12"
  BCM_COM_PROC_P5/15(V_BCM_COM_Whl_AS_Inhib_Cond_W34) -> [V_BCM_COM_Whl_AS_Inhib_Cond_W34]  "V_BCMA_COM_Whl_AS_Inhib_Cond_W34"
  BCM_COM_PROC_P5/16(V_BCM_COM_Whl_LP_AS_Curr_Order) -> [V_BCM_COM_Whl_LP_AS_Curr_Order]  "V_BCMA_COM_Whl_LP_AS_Curr_Order"
  BCM_COM_PROC_P5/17(V_BCM_COM_Wheel_Speed_Error_W12) -> [V_BCM_COM_Wheel_Speed_Error_W12]  "V_BCMA_COM_Wheel_Speed_Error_W12"
  BCM_COM_PROC_P5/18(V_BCM_COM_Wheel_Speed_Error_W34) -> [V_BCM_COM_Wheel_Speed_Error_W34]  "V_BCMA_COM_Wheel_Speed_Error_W34"
  BCM_COM_PROC_P5/19(V_BCM_COM_Whl_AS_Curr_Order) -> [V_BCM_COM_Whl_AS_Curr_Order]  "V_BCMA_COM_Whl_AS_Curr_Order"
  [V_BCM_COM_Whl_AS_Inhib_Cond_W12] -> BCM_COM_PROC_P20/79(V_BCM_COM_Whl_AS_Inhib_Cond_W12)
  [V_BCM_COM_Whl_AS_Inhib_Cond_W34] -> BCM_COM_PROC_P20/80(V_BCM_COM_Whl_AS_Inhib_Cond_W34)
  [V_BCM_COM_Whl_LP_AS_Curr_Order] -> BCM_COM_PROC_P20/81(V_BCM_COM_Whl_LP_AS_Curr_Order)
  [V_BCM_COM_SV_PT_Cons] -> BCM_COM_PROC_P20/82(V_BCM_COM_SV_PT_Cons)
  [V_BCM_COM_Wheel_Speed_Error_W12] -> BCM_COM_PROC_P20/85(V_BCM_COM_Wheel_Speed_Error_W12)
  [V_BCM_COM_Wheel_Speed_Error_W34] -> BCM_COM_PROC_P20/86(V_BCM_COM_Wheel_Speed_Error_W34)
  [V_BCM_COM_Whl_LP_AS_Curr_Order_W12] -> BCM_COM_PROC_P20/87(V_BCM_COM_Whl_LP_AS_Curr_Order_W12)
  [V_BCM_COM_Whl_LP_AS_Curr_Order_W34] -> BCM_COM_PROC_P20/88(V_BCM_COM_Whl_LP_AS_Curr_Order_W34)
  [V_BCM_COM_SV_Current] -> BCM_COM_PROC_P20/89(V_BCM_COM_SV_Current)
  [V_BCM_COM_SV_PT_Cons_Val] -> BCM_COM_PROC_P20/90(V_BCM_COM_SV_PT_Cons_Val)
  BUS_CAN_BCM_CCDL_TX/1(BUS_CAN_BCM_CCDL) -> BUS_CAN_BCM_CCDL/1
  BUS_CAN_BCM_CCDL_RX/1 -> BUS_CAN_BCM_CCDL_RX_/1(BUS_CAN_BCM_CCDL_RX)
  BUS_CAN_BCM_CCDL_RX_/1(V_BCM_COM_Big_Gamma_Trig_Out_W12) -> [V_BCM_COM_Big_Gamma_Trig_Out_W12_Opposite]
  BUS_CAN_BCM_CCDL_RX_/2(V_BCM_COM_Big_Gamma_Trig_Out_W34) -> [V_BCM_COM_Big_Gamma_Trig_Out_W34_Opposite]
  BUS_CAN_BCM_CCDL_RX_/3(V_BCM_COM_Big_Slip_Trig_Out_W12) -> [V_BCM_COM_Big_Slip_Trig_Out_W12_Opposite]
  BUS_CAN_BCM_CCDL_RX_/4(V_BCM_COM_Big_Slip_Trig_Out_W34) -> [V_BCM_COM_Big_Slip_Trig_Out_W34_Opposite]
  BUS_CAN_BCM_CCDL_RX_/5(V_BCM_COM_Big_Slip_WD_In_Mon_W12) -> [V_BCM_COM_Big_Slip_WD_Trig_Out_W12_Opposite]
  BUS_CAN_BCM_CCDL_RX_/6(V_BCM_COM_Big_Slip_WD_In_Mon_W34) -> [V_BCM_COM_Big_Slip_WD_Trig_Out_W34_Opposite]
  BUS_CAN_BCM_CCDL_RX_/7(V_BCM_COM_Small_Slip_Trig_Out_W12) -> [V_BCM_COM_Small_Slip_Trig_Out_W12_Opposite]
  BUS_CAN_BCM_CCDL_RX_/8(V_BCM_COM_Small_Slip_Trig_Out_W34) -> [V_BCM_COM_Small_Slip_Trig_Out_W34_Opposite]
  BUS_CAN_BCM_CCDL_RX_/9(V_BCM_COM_Target_Speed_Out_W12) -> [V_BCM_COM_Target_Speed_Out_W12_Opposite]
  BUS_CAN_BCM_CCDL_RX_/10(V_BCM_COM_Target_Speed_Out_W34) -> [V_BCM_COM_Target_Speed_Out_W34_Opposite]
  BUS_CAN_BCM_CCDL_RX_/11(V_BCM_COM_Adhesion_Out_W12) -> [V_BCM_COM_Adhesion_Out_W12_Opposite]
  BUS_CAN_BCM_CCDL_RX_/12(V_BCM_COM_Adhesion_Out_W34) -> [V_BCM_COM_Adhesion_Out_W34_Opposite]
  BUS_CAN_BCM_CCDL_RX_/13(V_BCM_COM_Opt_Adhesion_Out_W12) -> [V_BCM_COM_Opt_Adhesion_Out_W12_Opposite]
  BUS_CAN_BCM_CCDL_RX_/14(V_BCM_COM_Opt_Adhesion_Out_W34) -> [V_BCM_COM_Opt_Adhesion_Out_W34_Opposite]
  [V_BCM_COM_Big_Gamma_Trig_Out_W12_Opposite] -> Unit Delay22/1
  [V_BCM_COM_Big_Gamma_Trig_Out_W34_Opposite] -> Unit Delay23/1
  [V_BCM_COM_Small_Slip_Trig_Out_W12_Opposite] -> Unit Delay24/1
  [V_BCM_COM_Small_Slip_Trig_Out_W34_Opposite] -> Unit Delay25/1
  [V_BCM_COM_Big_Slip_WD_Trig_Out_W12_Opposite] -> Unit Delay20/1
  [V_BCM_COM_Big_Slip_WD_Trig_Out_W34_Opposite] -> Unit Delay21/1
  [V_BCM_COM_Target_Speed_Out_W12_Opposite] -> Unit Delay18/1
  [V_BCM_COM_Target_Speed_Out_W34_Opposite] -> Unit Delay19/1
  [V_BCM_COM_Opt_Adhesion_Out_W12_Opposite] -> Unit Delay14/1
  [V_BCM_COM_Opt_Adhesion_Out_W34_Opposite] -> Unit Delay15/1
  [V_BCM_COM_Adhesion_Out_W12_Opposite] -> Unit Delay16/1
  [V_BCM_COM_Adhesion_Out_W34_Opposite] -> Unit Delay17/1
  [V_BCM_COM_Big_Slip_Trig_Out_W34_Opposite] -> Unit Delay27/1
  [V_BCM_COM_Big_Slip_Trig_Out_W12_Opposite] -> Unit Delay26/1
  [V_BCM_COM_Wheel_Filtered_Speed_W34] -> Unit Delay29/1
  [V_BCM_COM_Wheel_Filtered_Speed_W12] -> Unit Delay28/1
  Selector8/1 -> BCM_COM_PROC_P5/18(V_BCM_COM_Tacho_Conf_Flt_W12)
  Selector9/1 -> BCM_COM_PROC_P5/19(V_BCM_COM_Tacho_Conf_Flt_W34)
  BCMA_COM_UF_LOCKED_WHEEL_W1/1 -> Mux8/1
  BCMA_COM_UF_LOCKED_WHEEL_W2/1 -> Mux8/2
  Mux8/1 -> BCM_COM_PROC_P5/22(V_BCM_COM_UF_LOCKED_WHEEL_W12)
  BCMA_COM_UF_LOCKED_WHEEL_W3/1 -> Mux9/1
  BCMA_COM_UF_LOCKED_WHEEL_W4/1 -> Mux9/2
  Mux9/1 -> BCM_COM_PROC_P5/23(V_BCM_COM_UF_LOCKED_WHEEL_W34)
  Unit Delay14/1 -> BCM_COM_PROC_P20/91(V_BCM_COM_Opt_Adhesion_In_Acq_W12)
  Unit Delay15/1 -> BCM_COM_PROC_P20/92(V_BCM_COM_Opt_Adhesion_In_Acq_W34)
  Unit Delay16/1 -> BCM_COM_PROC_P20/93(V_BCM_COM_Adhesion_In_Acq_W12)
  Unit Delay17/1 -> BCM_COM_PROC_P20/94(V_BCM_COM_Adhesion_In_Acq_W34)
  Unit Delay18/1 -> BCM_COM_PROC_P20/95(V_BCM_COM_Target_Speed_In_Acq_W12)
  Unit Delay19/1 -> BCM_COM_PROC_P20/96(V_BCM_COM_Target_Speed_In_Acq_W34)
  Unit Delay20/1 -> BCM_COM_PROC_P20/105(V_BCM_COM_Big_Slip_WD_Trig_In_Acq_W12)
  Unit Delay21/1 -> BCM_COM_PROC_P20/106(V_BCM_COM_Big_Slip_WD_Trig_In_Acq_W34)
  Unit Delay22/1 -> BCM_COM_PROC_P20/97(V_BCM_COM_Big_Gamma_Trig_In_Acq_W12)
  Unit Delay23/1 -> BCM_COM_PROC_P20/98(V_BCM_COM_Big_Gamma_Trig_In_Acq_W34)
  Unit Delay24/1 -> BCM_COM_PROC_P20/99(V_BCM_COM_Small_Slip_Trig_In_Acq_W12)
  Unit Delay25/1 -> BCM_COM_PROC_P20/100(V_BCM_COM_Small_Slip_Trig_In_Acq_W34)
  Unit Delay26/1 -> BCM_COM_PROC_P20/101(V_BCM_COM_Big_Slip_Trig_In_Acq_W12)
  Unit Delay27/1 -> BCM_COM_PROC_P20/102(V_BCM_COM_Big_Slip_Trig_In_Acq_W34)
  Unit Delay29/1 -> BCM_COM_PROC_P20/84(V_BCM_COM_Wheel_Filtered_Speed_W34)
  Unit Delay28/1 -> BCM_COM_PROC_P20/83(V_BCM_COM_Wheel_Filtered_Speed_W12)
  Unit Delay31/1 -> BCM_COM_PROC_P2_5/7(V_BCM_COM_Whl_LP_AS_Curr_Order_W12)
  Unit Delay32/1 -> BCM_COM_PROC_P2_5/8(V_BCM_COM_Press_Cmd_Rate_Lim)
  Unit Delay33/1 -> BCM_COM_PROC_P2_5/9(V_BCM_COM_Whl_LP_AS_Curr_Order_W34)
  [V_BCM_COM_A429_Wheel_Speed_W12] -> Demux4/1
  Demux1/1 -> BUS_A429_BCMA_GenIO_2_TX/3(BCMCP_RH_inboard_wheel_speed)
  Demux1/2 -> BUS_A429_BCMA_GenIO_2_TX/4(BCMCP_RH_outboard_wheel_speed)
  [V_BCM_COM_A429_Global_Wheel_Spd] -> BUS_A429_BCMA_GenIO_2_TX/5(BCMCP_global_wheel_speed)
  [V_BCM_COM_A429_Park_Brake_ON] -> BUS_A429_BCMA_GenIO_2_TX/34(BCMCP_park_brake_ON)
  [V_BCM_COM_A429_Antiskid_Activity] -> BUS_A429_BCMA_GenIO_2_TX/36(BCMCP_antiskid_activity)
  Demux6/1 -> BUS_A429_BCMA_GenIO_2_TX/41(BCMCP_LH_current_order_before_antiskid)
  Demux6/2 -> BUS_A429_BCMA_GenIO_2_TX/42(BCMCP_RH_current_order_before_antiskid)
  [V_BCM_COM_A429_Curr_Ord_Before_AS] -> Demux6/1
  [V_BCM_COM_A429_SV_Current_Readback] -> Demux8/1
  Demux8/1 -> BUS_A429_BCMA_GenIO_2_TX/45(BCMCP_LH_SV_current_readback)
  Demux8/2 -> BUS_A429_BCMA_GenIO_2_TX/46(BCMCP_RH_SV_current_readback)
  [V_BCM_COM_A429_SV_PT_In_Bar] -> Demux9/1
  [V_BCM_COM_A429_Pinprog_1] -> BUS_A429_BCMA_GenIO_2_TX/50(BCMCP_pinprog_1)
  [V_BCM_COM_A429_Pinprog_2] -> BUS_A429_BCMA_GenIO_2_TX/51(BCMCP_pinprog_2)
  [V_BCM_COM_A429_Pinprog_3] -> BUS_A429_BCMA_GenIO_2_TX/52(BCMCP_pinprog_3)
  [V_BCM_COM_A429_Maint_Mode_Req_28V] -> BUS_A429_BCMA_GenIO_2_TX/58(BCMCP_maintenance_mode_request_28V)
  [V_BCM_COM_A429_DBCU_LH_Brk_Cmd_Fdbk] -> BUS_A429_BCMA_GenIO_2_TX/60(BCMCP_DBCU_LH_brake_command_feedback)
  [V_BCM_COM_A429_DBCU_RH_Brk_Cmd_Fdbk] -> BUS_A429_BCMA_GenIO_2_TX/61(BCMCP_DBCU_RH_brake_command_feedback)
  [V_BCM_COM_A429_DBCU_Alt_Mode] -> BUS_A429_BCMA_GenIO_2_TX/59(BCMCP_DBCU_alternate_mode)
  [V_BCM_COM_A429_DBCU_Inhib_Opp_Side] -> BUS_A429_BCMA_GenIO_2_TX/62(BCMCP_DBCU_inhibition_opposite_side)
  [V_BCM_COM_A429_DFCS_Decel_Law_Inhib] -> BUS_A429_BCMA_GenIO_2_TX/68(DFCS_Decel_Law_Inhibition)
  [V_BCM_COM_A429_BCM_Fail] -> BUS_A429_BCMA_GenIO_2_TX/74(BCMCP_BCM_fail)
  [V_BCM_COM_A429_Antiskid_Activity] -> BUS_A429_BCMA_DFCS13_TX/14(BCMCP_Antiskid_Active)
  Demux5/1 -> BUS_A429_BCMA_DFCS13_TX/5(BCMCP_RHI_Wheel_Speed)
  Demux5/2 -> BUS_A429_BCMA_DFCS13_TX/6(BCMCP_RHO_Wheel_Speed)
  Control_Path_Start_Up/1 -> [Control_Path_Start_Up]
  [Control_Path_Start_Up] -> BCM_COM_PROC_P2_5/Enable
  [Control_Path_Start_Up] -> BCM_COM_PROC_P5/Enable
  [Control_Path_Start_Up] -> BCM_COM_PROC_P20/Enable
  Ground1/1 -> BUS_A429_BCMA_GenIO_2_TX/79(BCMCP_Minor_Fault)
  Ground4/1 -> BUS_A429_BCMA_GenIO_2_TX/70(BCMCP_Alternate_Switch)
  Ground2/1 -> BUS_A429_BCMA_GenIO_2_TX/69(BCMCP_Park_Switch)
  Ground3/1 -> BUS_A429_BCMA_GenIO_2_TX/40(BCMCP_Engine_Run_Up)
  Constant8/1 -> [DFCSA_Capsule_Validity]
  Constant9/1 -> [DFCSB_Capsule_Validity]
  DFCS1_Label204_Validity/2(LMLG_WOWs_Val) -> [DFCSA_LMLG_WOWs_Val]
  DFCS1_Label204_Validity/1(WOWs_Val_Val) -> [DFCSA_WOWs_Val_Val]
  DFCS1_Label204_Validity/3(RMLG_WOWs_Val) -> [DFCSA_RMLG_WOWs_Val]
  DFCS1_Label204_Validity/4(NLG_WOWs_Val) -> [DFCSA_NLG_WOWs_Val]
  DFCS1_Label204_Validity/5(TLA_Above_Idle_Val) -> [DFCSA_TLA_Above_Idle_Val]
  DFCS1_Label204_Validity/6(DCL_Inhibition_Val) -> [DFCSA_DCL_Inhibition_Val]
  [DFCSA_Capsule_Validity] -> DFCS1_Label204_Validity/1(Capsule_Validity)
  Constant11/1 -> DFCS1_Label204_Validity/2(Label204_Not_Refreshed)
  DFCSA_Label202_Validity/2(RH_Braking_Cmd_Val) -> [DFCSA_RH_Braking_Cmd_Val]
  DFCSA_Label202_Validity/1(LH_Braking_Cmd_Val) -> [DFCSA_LH_Braking_Cmd_Val]
  [DFCSA_Capsule_Validity] -> DFCSA_Label202_Validity/1(Capsule_Validity)
  Constant10/1 -> DFCSA_Label202_Validity/2(Label202_Not_Refreshed)
  DFCS1_Label205_Validity/1(Long_Accel_Val) -> [DFCSA_Long_Accel_Val]
  [DFCSA_Capsule_Validity] -> DFCS1_Label205_Validity/1(Capsule_Validity)
  Constant12/1 -> DFCS1_Label205_Validity/2(Label205_Not_Refreshed)
  DFCS1_Label207_Validity/1(Pitch_Ang_Val) -> [DFCSA_Pitch_Ang_Val]
  [DFCSA_Capsule_Validity] -> DFCS1_Label206_Validity/1(Capsule_Validity)
  Constant1/1 -> DFCS1_Label206_Validity/2(Label206_Not_Refreshed)
  Constant14/1 -> DFCS1_Label207_Validity/2(Label207_Not_Refreshed)
  [DFCSA_Capsule_Validity] -> DFCS1_Label207_Validity/1(Capsule_Validity)
  Constant4/1 -> DFCSA_Label202_Validity/3(Label202_Corrupted)
  Constant6/1 -> DFCS1_Label204_Validity/3(Label204_Corrupted)
  Constant13/1 -> DFCS1_Label205_Validity/3(Label205_Corrupted)
  Constant15/1 -> DFCS1_Label206_Validity/3(Label206_Corrupted)
  Constant17/1 -> DFCS1_Label207_Validity/3(Label207_Corrupted)
  Bus Selector/20 -> [DFCSA_Label202_SSM]  "<BUS_A429_DFCS1_BCMA_LABEL_202_SSM>"
  Bus Selector/21 -> [DFCSA_Label204_SSM]  "<BUS_A429_DFCS1_BCMA_LABEL_204_SSM>"
  Bus Selector/22 -> [DFCSA_Label205_SSM]  "<BUS_A429_DFCS1_BCMA_LABEL_205_SSM>"
  Bus Selector/23 -> [DFCSA_Label206_SSM]  "<BUS_A429_DFCS1_BCMA_LABEL_206_SSM>"
  Bus Selector/24 -> [DFCSA_Label207_SSM]  "<BUS_A429_DFCS1_BCMA_LABEL_207_SSM>"
  [DFCSA_Label202_SSM] -> DFCSA_Label202_Validity/4(Label202_SSM)
  [DFCSA_Label204_SSM] -> DFCS1_Label204_Validity/4(Label204_SSM)
  [DFCSA_Label205_SSM] -> DFCS1_Label205_Validity/4(Label205_SSM)
  [DFCSA_Label206_SSM] -> DFCS1_Label206_Validity/4(Label206_SSM)
  [DFCSA_Label207_SSM] -> DFCS1_Label207_Validity/4(Label207_SSM)
  [DFCSB_Label202_SSM] -> DFCSB_Label202_Validity1/4(Label202_SSM)
  Constant21/1 -> DFCSB_Label202_Validity1/3(Label202_Corrupted)
  Constant19/1 -> DFCSB_Label202_Validity1/2(Label202_Not_Refreshed)
  [DFCSB_Capsule_Validity] -> DFCSB_Label202_Validity1/1(Capsule_Validity)
  DFCSB_Label202_Validity1/1(LH_Braking_Cmd_Val) -> [DFCSB_LH_Braking_Cmd_Val]
  DFCSB_Label202_Validity1/2(RH_Braking_Cmd_Val) -> [DFCSB_RH_Braking_Cmd_Val]
  Bus Selector1/20 -> [DFCSB_Label202_SSM]  "<BUS_A429_DFCS3_BCMA_LABEL_202_SSM>"
  Bus Selector1/21 -> [DFCSB_Label204_SSM]  "<BUS_A429_DFCS3_BCMA_LABEL_204_SSM>"
  Bus Selector1/22 -> [DFCSB_Label205_SSM]  "<BUS_A429_DFCS3_BCMA_LABEL_205_SSM>"
  Bus Selector1/23 -> [DFCSB_Label206_SSM]  "<BUS_A429_DFCS3_BCMA_LABEL_206_SSM>"
  Bus Selector1/24 -> [DFCSB_Label207_SSM]  "<BUS_A429_DFCS3_BCMA_LABEL_207_SSM>"
  [DFCSB_Label204_SSM] -> DFCS3_Label204_Validity/4(Label204_SSM)
  Constant5/1 -> DFCS3_Label204_Validity/3(Label204_Corrupted)
  Constant3/1 -> DFCS3_Label204_Validity/2(Label204_Not_Refreshed)
  [DFCSB_Capsule_Validity] -> DFCS3_Label204_Validity/1(Capsule_Validity)
  DFCS3_Label204_Validity/1(WOWs_Val_Val) -> [DFCSB_WOWs_Val_Val]
  DFCS3_Label204_Validity/2(LMLG_WOWs_Val) -> [DFCSB_LMLG_WOWs_Val]
  DFCS3_Label204_Validity/3(RMLG_WOWs_Val) -> [DFCSB_RMLG_WOWs_Val]
  DFCS3_Label204_Validity/4(NLG_WOWs_Val) -> [DFCSB_NLG_WOWs_Val]
  DFCS3_Label204_Validity/5(TLA_Above_Idle_Val) -> [DFCSB_TLA_Above_Idle_Val]
  DFCS3_Label204_Validity/6(DCL_Inhibition_Val) -> [DFCSB_DCL_Inhibition_Val]
  [DFCSB_Label205_SSM] -> DFCS3_Label205_Validity/4(Label205_SSM)
  Constant18/1 -> DFCS3_Label205_Validity/3(Label205_Corrupted)
  Constant7/1 -> DFCS3_Label205_Validity/2(Label205_Not_Refreshed)
  [DFCSB_Capsule_Validity] -> DFCS3_Label205_Validity/1(Capsule_Validity)
  DFCS3_Label205_Validity/1(Long_Accel_Val) -> [DFCSB_Long_Accel_Val]
  [DFCSB_Label206_SSM] -> DFCS3_Label206_Validity/4(Label206_SSM)
  Constant22/1 -> DFCS3_Label206_Validity/3(Label206_Corrupted)
  Constant20/1 -> DFCS3_Label206_Validity/2(Label206_Not_Refreshed)
  [DFCSB_Capsule_Validity] -> DFCS3_Label206_Validity/1(Capsule_Validity)
  [DFCSB_Label207_SSM] -> DFCS3_Label207_Validity/4(Label207_SSM)
  Constant24/1 -> DFCS3_Label207_Validity/3(Label207_Corrupted)
  [DFCSB_Capsule_Validity] -> DFCS3_Label207_Validity/1(Capsule_Validity)
  Constant23/1 -> DFCS3_Label207_Validity/2(Label207_Not_Refreshed)
  DFCS3_Label207_Validity/1(Pitch_Ang_Val) -> [DFCSB_Pitch_Ang_Val]
  Constant31/1 -> GenIO_Label021_Validity/1(Label021_Not_Refreshed)
  Constant32/1 -> GenIO_Label021_Validity/2(Label021_Corrupted)
  Bus Selector2/8 -> [GenIO_Label021_SSM]  "<BUS_A429_GenIO_1A_GPHS_LABEL_021_SSM>"
  Bus Selector2/9 -> [GenIO_Label022_SSM]  "<BUS_A429_GenIO_1A_GPHS_LABEL_022_SSM>"
  Bus Selector2/10 -> [GenIO_Label272_SSM]  "<BUS_A429_GenIO_1A_GPHS_LABEL_272_SSM>"
  Bus Selector2/11 -> [GenIO_Label273_SSM]  "<BUS_A429_GenIO_1A_GPHS_LABEL_273_SSM>"
  [GenIO_Label021_SSM] -> GenIO_Label021_Validity/3(Label021_SSM)
  GenIO_Label021_Validity/1(Hyd_B_Press_Val) -> [Hyd_B_Press_Val]
  [GenIO_Label022_SSM] -> GenIO_Label022_Validity/3(Label022_SSM)
  Constant34/1 -> GenIO_Label022_Validity/2(Label022_Corrupted)
  Constant33/1 -> GenIO_Label022_Validity/1(Label022_Not_Refreshed)
  GenIO_Label022_Validity/1(Hyd_A_Press_Val) -> [Hyd_A_Press_Val]
  GenIO_Label272_Validity/1(Engine1_Running_Val) -> [Engine1_Running_Val]
  [GenIO_Label272_SSM] -> GenIO_Label272_Validity/3(Label272_SSM)
  Constant49/1 -> GenIO_Label272_Validity/2(Label272_Corrupted)
  Constant37/1 -> GenIO_Label272_Validity/1(Label272_Not_Refreshed)
  Constant55/1 -> GenIO_Label273_Validity/1(Label273_Not_Refreshed)
  Constant56/1 -> GenIO_Label273_Validity/2(Label273_Corrupted)
  [GenIO_Label273_SSM] -> GenIO_Label273_Validity/3(Label273_SSM)
  GenIO_Label273_Validity/1(Engine2_Running_Val) -> [Engine2_Running_Val]
  [Hyd_A_Press] -> GenIO_Label022_Validity/4(Hyd_A_Press)
  [Hyd_B_Press] -> GenIO_Label021_Validity/4(Hyd_B_Press)
  [DFCSA_LH_Braking_Cmd] -> DFCSA_Label202_Validity/5(DFCSA_LH_Braking_Cmd)
  [DFCSA_RH_Braking_Cmd] -> DFCSA_Label202_Validity/6(DFCSA_RH_Braking_Cmd)
  [DFCSB_LH_Braking_Cmd] -> DFCSB_Label202_Validity1/5(DFCSB_LH_Braking_Cmd)
  [DFCSB_RH_Braking_Cmd] -> DFCSB_Label202_Validity1/6(DFCSB_RH_Braking_Cmd)
  [DFCSA_Gnd_Spd] -> DFCS1_Label206_Validity/5(DFCSA_Gnd_Spd)
  [DFCSB_Gnd_Spd] -> DFCS3_Label206_Validity/5(DFCSB_Gnd_Spd)
  [DFCSA_Pitch_Ang] -> DFCS1_Label207_Validity/5(DFCSA_Pitch_Ang)
  [DFCSB_Pitch_Ang] -> DFCS3_Label207_Validity/5(DFCSB_Pitch_Ang)
  [DFCSA_Long_Accel] -> DFCS1_Label205_Validity/5(DFCSA_Long_Accel)
  [DFCSB_Long_Accel] -> DFCS3_Label205_Validity/5(DFCSB_Long_Accel)
  DFCSA_LH_Braking_Cmd_Comp/1(Braking_Cmd_out) -> BCM_COM_PROC_P20/38(V_BCM_COM_DFCS_A_DFCS_LH_Braking_Cmd_Acq)
  [DFCSA_LH_Braking_Cmd] -> DFCSA_LH_Braking_Cmd_Comp/1(Braking_Cmd)
  [DFCSA_LH_Braking_Cmd_Val] -> DFCSA_LH_Braking_Cmd_Comp/2(Braking_Cmd_Val)
  DFCSA_RH_Braking_Cmd_Comp/1(Braking_Cmd_out) -> BCM_COM_PROC_P20/39(V_BCM_COM_DFCS_A_DFCS_RH_Braking_Cmd_Acq)
  [DFCSA_RH_Braking_Cmd] -> DFCSA_RH_Braking_Cmd_Comp/1(Braking_Cmd)
  [DFCSA_RH_Braking_Cmd_Val] -> DFCSA_RH_Braking_Cmd_Comp/2(Braking_Cmd_Val)
  [DFCSB_LH_Braking_Cmd] -> DFCSB_LH_Braking_Cmd_Comp/1(Braking_Cmd)
  [DFCSB_LH_Braking_Cmd_Val] -> DFCSB_LH_Braking_Cmd_Comp/2(Braking_Cmd_Val)
  [DFCSB_RH_Braking_Cmd] -> DFCSB_RH_Braking_Cmd_Comp/1(Braking_Cmd)
  [DFCSB_RH_Braking_Cmd_Val] -> DFCSB_RH_Braking_Cmd_Comp/2(Braking_Cmd_Val)
  DFCSA_Ground_Speed_Comp/1(Ground_Speed_out) -> BCM_COM_PROC_P20/2(V_BCM_COM_DFCS_A_Gnd_Spd_Acq)
  [DFCSA_Gnd_Spd_Val] -> DFCSA_Ground_Speed_Comp/2(Ground_Speed_Val)
  [DFCSA_Gnd_Spd] -> DFCSA_Ground_Speed_Comp/1(Ground_Speed)
  DFCSB_Ground_Speed_Comp/1(Ground_Speed_out) -> BCM_COM_PROC_P20/3(V_BCM_COM_DFCS_B_Gnd_Spd_Acq)
  [DFCSB_Gnd_Spd_Val] -> DFCSB_Ground_Speed_Comp/2(Ground_Speed_Val)
  [DFCSB_Gnd_Spd] -> DFCSB_Ground_Speed_Comp/1(Ground_Speed)
  DFCSA_Long_Accel_Comp/1(Long_Accel_out) -> BCM_COM_PROC_P20/6(V_BCM_COM_DFCS_A_Long_Accel_Acq)
  [DFCSA_Long_Accel_Val] -> DFCSA_Long_Accel_Comp/2(Long_Accel_Val)
  [DFCSA_Long_Accel] -> DFCSA_Long_Accel_Comp/1(Long_Accel)
  DFCSB_Long_Accel_Comp/1(Long_Accel_out) -> BCM_COM_PROC_P20/7(V_BCM_COM_DFCS_B_Long_Accel_Acq)
  [DFCSB_Long_Accel_Val] -> DFCSB_Long_Accel_Comp/2(Long_Accel_Val)
  [DFCSB_Long_Accel] -> DFCSB_Long_Accel_Comp/1(Long_Accel)
  DFCSA_Pitch_Angle_Comp/1(Pitch_Angle_out) -> BCM_COM_PROC_P20/10(V_BCM_COM_DFCS_A_Pitch_Ang_Acq)
  [DFCSA_Pitch_Ang_Val] -> DFCSA_Pitch_Angle_Comp/2(Pitch_Angle_Val)
  [DFCSA_Pitch_Ang] -> DFCSA_Pitch_Angle_Comp/1(Pitch_Angle)
  DFCSB_Pitch_Angle_Comp/1(Pitch_Angle_out) -> BCM_COM_PROC_P20/11(V_BCM_COM_DFCS_B_Pitch_Ang_Acq)
  [DFCSB_Pitch_Ang_Val] -> DFCSB_Pitch_Angle_Comp/2(Pitch_Angle_Val)
  [DFCSB_Pitch_Ang] -> DFCSB_Pitch_Angle_Comp/1(Pitch_Angle)
  DFCSA_WOWs_Val_Comp/1(WOWs_Val_Acq_out) -> BCM_COM_PROC_P20/14(V_BCM_COM_DFCS_A_WOWs_Val_Acq)
  [DFCSA_WOWs_Val_Val] -> DFCSA_WOWs_Val_Comp/2(WOWs_Val_Val)
  [DFCSA_WOWs_Val_Acq] -> DFCSA_WOWs_Val_Comp/1(WOWs_Val_Acq)
  DFCSB_WOWs_Val_Comp/1(WOWs_Val_Acq_out) -> BCM_COM_PROC_P20/15(V_BCM_COM_DFCS_B_WOWs_Val_Acq)
  [DFCSB_WOWs_Val_Val] -> DFCSB_WOWs_Val_Comp/2(WOWs_Val_Val)
  [DFCSB_WOWs_Val_Acq] -> DFCSB_WOWs_Val_Comp/1(WOWs_Val_Acq)
  [DFCSA_LMLG_WOWs] -> DFCSA_LMLG_WOWs_Comp/1(LMLG_WOWs)
  [DFCSA_LMLG_WOWs_Val] -> DFCSA_LMLG_WOWs_Comp/2(LMLG_WOWs_Val)
  DFCSA_LMLG_WOWs_Comp/1(LMLG_WOWs_out) -> BCM_COM_PROC_P20/20(V_BCM_COM_DFCS_A_LMLG_WOWs_Acq)
  [DFCSB_LMLG_WOWs] -> DFCSB_LMLG_WOWs_Comp/1(LMLG_WOWs)
  [DFCSB_LMLG_WOWs_Val] -> DFCSB_LMLG_WOWs_Comp/2(LMLG_WOWs_Val)
  [DFCSB_RMLG_WOWs_Val] -> DFCSB_RMLG_WOWs_Comp/2(RMLG_WOWs_Val)
  [DFCSA_RMLG_WOWs] -> DFCSA_RMLG_WOWs_Comp/1(RMLG_WOWs)
  [DFCSB_RMLG_WOWs] -> DFCSB_RMLG_WOWs_Comp/1(RMLG_WOWs)
  [DFCSA_RMLG_WOWs_Val] -> DFCSA_RMLG_WOWs_Comp/2(RMLG_WOWs_Val)
  [DFCSA_NLG_WOWs_Val] -> DFCSA_NLG_WOWs_Comp/2(NLG_WOWs_Val)
  [DFCSB_NLG_WOWs] -> DFCSB_NLG_WOWs_Comp/1(NLG_WOWs)
  [DFCSA_NLG_WOWs] -> DFCSA_NLG_WOWs_Comp/1(NLG_WOWs)
  [DFCSB_NLG_WOWs_Val] -> DFCSB_NLG_WOWs_Comp/2(NLG_WOWs_Val)
  DFCSA_DCL_Inhibition_Comp/1(DCL_Inhibition_out) -> BCM_COM_PROC_P20/43(V_BCM_COM_DFCS_A_Decel_Law_Inhib_Acq)
  [DFCSA_DCL_Inhibition] -> DFCSA_DCL_Inhibition_Comp/1(DCL_Inhibition)
  [DFCSA_DCL_Inhibition_Val] -> DFCSA_DCL_Inhibition_Comp/2(DCL_Inhibition_Val)
  [DFCSB_DCL_Inhibition_Val] -> DFCSB_DCL_Inhibition_Comp/2(DCL_Inhibition_Val)
  [DFCSB_DCL_Inhibition] -> DFCSB_DCL_Inhibition_Comp/1(DCL_Inhibition)
  [DFCSA_TLA_Above_Idle_Val] -> DFCSA_TLA_Above_Idle_Comp/2(TLA_Above_Idle_Val)
  [DFCSA_TLA_Above_Idle] -> DFCSA_TLA_Above_Idle_Comp/1(TLA_Above_Idle)
  DFCSA_TLA_Above_Idle_Comp/1(TLA_Above_Idle_out) -> BCM_COM_PROC_P20/48(V_BCM_COM_DFCS_A_TLA_Above_Idle_Acq)
  [DFCSB_TLA_Above_Idle] -> DFCSB_TLA_Above_Idle_Comp/1(TLA_Above_Idle)
  [DFCSB_TLA_Above_Idle_Val] -> DFCSB_TLA_Above_Idle_Comp/2(TLA_Above_Idle_Val)
  DFCSB_TLA_Above_Idle_Comp/1(TLA_Above_Idle_out) -> BCM_COM_PROC_P20/49(V_BCM_COM_DFCS_B_TLA_Above_Idle_Acq)
  BUS_ETH_BCMA_MMS_TX/1(BUS_ETH_BCMA_MMS) -> BUS_ETH_BCMA_MMS/1
  [ETH_AC_State] -> BUS_ETH_BCMA_MMS_TX/1(AC_state)
  [ETH_AC_Flight_Phase] -> BUS_ETH_BCMA_MMS_TX/2(AC_flight_phase)
  [ETH_Braking_Mode] -> BUS_ETH_BCMA_MMS_TX/3(Braking_mode)
  [ETH_Braking_Norm_FT_Seq] -> BUS_ETH_BCMA_MMS_TX/4(Sequence_preland_test)
  [ETH_Braking_Alt_FT_Seq] -> BUS_ETH_BCMA_MMS_TX/5(Sequence_alternate_test)
  [ETH_FB_BCM_FAIL] -> BUS_ETH_BCMA_MMS_TX/6(BCM_FAIL)
  [ETH_FB_BCM_DBCU_MODE_DIS] -> BUS_ETH_BCMA_MMS_TX/7(BCM_DBCU_MODE_DIS)
  [ETH_FB_DBCU_SIMULT_ACT] -> BUS_ETH_BCMA_MMS_TX/8(BCM_DBCU_SIMULTANEOUS_ACTIVITY)
  [ETH_FB_DBCU_FAIL] -> BUS_ETH_BCMA_MMS_TX/9(DBCU_FAIL)
  [ETH_FB_DBCU_BRK_ORDER_FAIL] -> BUS_ETH_BCMA_MMS_TX/10(DBCU_BRK_ORDER_FAIL)
  [ETH_FB_INHIB_FAIL] -> BUS_ETH_BCMA_MMS_TX/11(DBCU_INHIBITION_FAIL)
  [ETH_FB_HYD_A_LOW_PRESS] -> BUS_ETH_BCMA_MMS_TX/12(HYD_A_LOW_PRESSURE)
  [ETH_FB_HYD_B_LOW_PRESS] -> BUS_ETH_BCMA_MMS_TX/13(HYD_B_LOW_PRESSURE)
  [ETH_FB_ACCU_LOW_PRESS] -> BUS_ETH_BCMA_MMS_TX/14(ACCU_LOW_PRESSURE)
  [ETH_FB_ACCU_PT_FAIL] -> BUS_ETH_BCMA_MMS_TX/15(ACCU_PT_FAIL)
  [ETH_FB_DFCS_A_RX] -> BUS_ETH_BCMA_MMS_TX/16(DFCS_A_RX)
  [ETH_FB_DFCS_B_RX] -> BUS_ETH_BCMA_MMS_TX/17(DFCS_B_RX)
  [ETH_FB_BSELV_CMD_FAIL] -> BUS_ETH_BCMA_MMS_TX/18(BSELV_CMD_FAIL)
  [ETH_FB_BSELV_JCL] -> BUS_ETH_BCMA_MMS_TX/19(BSELV_JCL)
  [ETH_FB_BSELV_JOP] -> BUS_ETH_BCMA_MMS_TX/20(BSELV_JOP)
  [ETH_FB_LH_SV_PT_FAIL] -> BUS_ETH_BCMA_MMS_TX/21(LH_SV_PT_FAIL)
  [ETH_FB_LH_SV_CMD_FAIL] -> BUS_ETH_BCMA_MMS_TX/22(LH_SV_CMD_FAIL)
  [ETH_FB_LH_SV_JCL] -> BUS_ETH_BCMA_MMS_TX/23(LH_SV_JCL)
  [ETH_FB_LH_SV_JOP] -> BUS_ETH_BCMA_MMS_TX/24(LH_SV_JOP)
  [ETH_FB_RH_SV_PT_FAIL] -> BUS_ETH_BCMA_MMS_TX/25(RH_SV_PT_FAIL)
  [ETH_FB_RH_SV_CMD_FAIL] -> BUS_ETH_BCMA_MMS_TX/26(RH_SV_CMD_FAIL)
  [ETH_FB_RH_SV_JCL] -> BUS_ETH_BCMA_MMS_TX/27(RH_SV_JCL)
  [ETH_FB_RH_SV_JOP] -> BUS_ETH_BCMA_MMS_TX/28(RH_SV_JOP)
  [ETH_FB_LH_OUT_TACHO_FAIL] -> BUS_ETH_BCMA_MMS_TX/29(LH_OUT_TACHO_FAIL)
  [ETH_FB_LH_IN_TACHO_FAIL] -> BUS_ETH_BCMA_MMS_TX/30(LH_IN_TACHO_FAIL)
  [ETH_FB_RH_IN_TACHO_FAIL] -> BUS_ETH_BCMA_MMS_TX/31(RH_IN_TACHO_FAIL)
  [ETH_FB_RH_OUT_TACHO_FAIL] -> BUS_ETH_BCMA_MMS_TX/32(RH_OUT_TACHO_FAIL)
  [ETH_FB_LG_LEVER_FAIL] -> BUS_ETH_BCMA_MMS_TX/33(LG_LEVER_FAIL)
  [ETH_FB_LMLG_DWNLOCK_FAIL] -> BUS_ETH_BCMA_MMS_TX/34(LMLG_DWNLOCK_FAIL)
  [ETH_FB_RMLG_DWNLOCK_FAIL] -> BUS_ETH_BCMA_MMS_TX/35(RMLG_DWNLOCK_FAIL)
  Ground76/1 -> BUS_ETH_BCMA_MMS_TX/36(ESC_WOW_FAIL)
  [ETH_FB_PARK_BRK_STATUS_DIS] -> BUS_ETH_BCMA_MMS_TX/37(PARK_BRK_STATUS_DIS)
  [ETH_FB_MAINT_MODE_DIS] -> BUS_ETH_BCMA_MMS_TX/38(MAINTENANCE_MODE_DIS)
  [ETH_TT_in_progress_id] -> BUS_ETH_BCMA_MMS_TX/39(TT_inprogress_id)
  [ETH_TT_rejection_cause] -> BUS_ETH_BCMA_MMS_TX/40(TT_rejection_cause)
  [ETH_TT_rejected] -> BUS_ETH_BCMA_MMS_TX/41(TT_rejected)
  [ETH_TT_completed] -> BUS_ETH_BCMA_MMS_TX/42(TT_completed)
  [ETH_TT_result_significant] -> BUS_ETH_BCMA_MMS_TX/43(TT_result_significant)
  Ground88/1 -> BUS_ETH_BCMA_MMS_TX/44(LH_HASV_CURRENT_TEST_ENABLED_ECHO)
  Ground89/1 -> BUS_ETH_BCMA_MMS_TX/45(LH_HASV_CURRENT_TEST_CMD_ECHO)
  Ground90/1 -> BUS_ETH_BCMA_MMS_TX/46(RH_HASV_CURRENT_TEST_ENABLED_ECHO)
  Ground91/1 -> BUS_ETH_BCMA_MMS_TX/47(RH_HASV_CURRENT_TEST_CMD_ECHO)
  Ground87/1 -> BUS_ETH_BCMA_MMS_TX/48(HASELV_CMD_TEST_ENABLED_ECHO)
  Ground105/1 -> BUS_ETH_BCMA_MMS_TX/49(HASELV_CMD_TEST_CMD_ECHO)
  Ground106/1 -> BUS_ETH_BCMA_MMS_TX/50(BCMA_DBCU_INHIBITION_TEST_ENABLED_ECHO)
  Ground107/1 -> BUS_ETH_BCMA_MMS_TX/51(BCMA_DBCU_INHIBITION_TEST_CMD_ECHO)
  [ETH_Invalid_Config] -> BUS_ETH_BCMA_MMS_TX/52(DEFAULT_BECAUSE_WRONG_PIN_PROG)
  Ground108/1 -> BUS_ETH_BCMA_MMS_TX/53(DEFAULT_BECAUSE_SWAP)
  BCM_COM_PROC_P20/33(V_BCM_COM_LH_Braking_Cmd_Cons) -> Terminator21/1  "V_BCMA_COM_LH_Braking_Cmd_Cons"
  BCM_COM_PROC_P20/34(V_BCM_COM_RH_Braking_Cmd_Cons) -> Terminator15/1  "V_BCMA_COM_RH_Braking_Cmd_Cons"
  BCM_COM_PROC_P20/35(V_BCM_COM_Decel_Law_Inhib_Cons) -> Terminator20/1  "V_BCMA_COM_Decel_Law_Inhib_Cons"
  BCM_COM_PROC_P20/48(V_BCM_COM_SELV_High_Side_Cmd_Order) -> [SELV_High_Side_Cmd_Order]  "V_BCMA_COM_SELV_High_Side_Cmd_Order"
  BCM_COM_PROC_P20/58(V_BCM_COM_Global_Wheel_Spd) -> Terminator226/1  "V_BCMA_COM_Global_Wheel_Spd"
  BCM_COM_PROC_P20/61(V_BCM_COM_AC_State) -> [V_BCM_COM_AC_State]  "V_BCMA_COM_AC_State"
  BCM_COM_PROC_P20/62(V_BCM_COM_AC_Flight_Phase) -> [V_BCM_COM_AC_Flight_Phase]  "V_BCMA_COM_AC_Flight_Phase"
  BCM_COM_PROC_P20/63(V_BCM_COM_Braking_Mode) -> [Braking_Mode]  "V_BCMA_COM_Braking_Mode"
  BCM_COM_PROC_P20/71(V_BCM_COM_Braking_Alt_FT_Seq) -> [V_BCM_COM_Braking_Alt_FT_Seq]  "V_BCMA_COM_Braking_Alt_FT_Seq"
  BCM_COM_PROC_P20/75(V_BCM_COM_LH_Press_Reg_FT_Act_Cond) -> [LH_Press_Reg_FT_Act_Cond]  "V_BCMA_COM_LH_Press_Reg_FT_Act_Cond"
  BCM_COM_PROC_P20/76(V_BCM_COM_RH_Press_Reg_FT_Act_Cond) -> [RH_Press_Reg_FT_Act_Cond]  "V_BCMA_COM_RH_Press_Reg_FT_Act_Cond"
  BCM_COM_PROC_P20/88(V_BCM_COM_BCM_Validity) -> [V_BCM_COM_BCM_Validity]  "V_BCMA_COM_BCM_Validity"
  BCM_COM_PROC_P20/87(V_BCM_COM_DBCU_Inhib_Order) -> [DBCU_Inhib_Order]  "V_BCMA_COM_DBCU_Inhib_Order"
  BCM_COM_PROC_P20/95(V_BCM_COM_Braking_State) -> [Braking_State]  "V_BCMA_COM_Braking_State"
  BCM_COM_PROC_P20/94(V_BCM_COM_BCP_BCM_Alt_Sw_On_Cmd_Conf) -> Terminator225/1  "V_BCMA_COM_BCP_BCM_Alt_Sw_On_Cmd_Conf"
  BCM_COM_PROC_P20/99(V_BCM_COM_Press_Cmd) -> [Press_Cmd_Rate_Lim]  "V_BCMA_COM_Press_Cmd"
  BCM_COM_PROC_P20/100(V_BCM_COM_Brkg_On_Wheels) -> [Brkg_On_Wheels]  "V_BCMA_COM_Brkg_On_Wheels"
  BCM_COM_PROC_P20/103(V_BCM_COM_PBSELV_State_Cons) -> [PBSELV_State_Cons]  "V_BCMA_COM_PBSELV_State_Cons"
  BCM_COM_PROC_P20/112(V_BCM_COM_Wheel_Control_Speed_W12) -> [V_BCM_COM_Wheel_Control_Speed_W12]  "V_BCMA_COM_Wheel_Control_Speed_W12"
  BCM_COM_PROC_P20/113(V_BCM_COM_Wheel_Control_Speed_W34) -> [V_BCM_COM_Wheel_Control_Speed_W34]  "V_BCMA_COM_Wheel_Control_Speed_W34"
  BCM_COM_PROC_P20/114(V_BCM_COM_Big_Gamma_Trig_Out_W12) -> [V_BCM_COM_Big_Gamma_Trig_Out_W12]  "V_BCMA_COM_Big_Gamma_Trig_Out_W12"
  BCM_COM_PROC_P20/115(V_BCM_COM_Big_Gamma_Trig_Out_W34) -> [V_BCM_COM_Big_Gamma_Trig_Out_W34]  "V_BCMA_COM_Big_Gamma_Trig_Out_W34"
  BCM_COM_PROC_P20/116(V_BCM_COM_Big_Slip_Trig_Out_W12) -> [V_BCM_COM_Big_Slip_Trig_Out_W12]  "V_BCMA_COM_Big_Slip_Trig_Out_W12"
  BCM_COM_PROC_P20/117(V_BCM_COM_Big_Slip_Trig_Out_W34) -> [V_BCM_COM_Big_Slip_Trig_Out_W34]  "V_BCMA_COM_Big_Slip_Trig_Out_W34"
  BCM_COM_PROC_P20/118(V_BCM_COM_Big_Slip_WD_Trig_Out_W12) -> [V_BCM_COM_Big_Slip_WD_Trig_Out_W12]  "V_BCMA_COM_Big_Slip_WD_Trig_Out_W12"
  BCM_COM_PROC_P20/119(V_BCM_COM_Big_Slip_WD_Trig_Out_W34) -> [V_BCM_COM_Big_Slip_WD_Trig_Out_W34]  "V_BCMA_COM_Big_Slip_WD_Trig_Out_W34"
  BCM_COM_PROC_P20/120(V_BCM_COM_Small_Slip_Trig_Out_W12) -> [V_BCM_COM_Small_Slip_Trig_Out_W12]  "V_BCMA_COM_Small_Slip_Trig_Out_W12"
  BCM_COM_PROC_P20/121(V_BCM_COM_Small_Slip_Trig_Out_W34) -> [V_BCM_COM_Small_Slip_Trig_Out_W34]  "V_BCMA_COM_Small_Slip_Trig_Out_W34"
  BCM_COM_PROC_P20/124(V_BCM_COM_Target_Speed_Out_W12) -> [V_BCM_COM_Target_Speed_Out_W12]  "V_BCMA_COM_Target_Speed_Out_W12"
  BCM_COM_PROC_P20/125(V_BCM_COM_Target_Speed_Out_W34) -> [V_BCM_COM_Target_Speed_Out_W34]  "V_BCMA_COM_Target_Speed_Out_W34"
  BCM_COM_PROC_P20/128(V_BCM_COM_Adhesion_Out_W12) -> [V_BCM_COM_Adhesion_Out_W12]  "V_BCMA_COM_Adhesion_Out_W12"
  BCM_COM_PROC_P20/129(V_BCM_COM_Adhesion_Out_W34) -> [V_BCM_COM_Adhesion_Out_W34]  "V_BCMA_COM_Adhesion_Out_W34"
  BCM_COM_PROC_P20/130(V_BCM_COM_Opt_Adhesion_Out_W12) -> [V_BCM_COM_Opt_Adhesion_Out_W12]  "V_BCMA_COM_Opt_Adhesion_Out_W12"
  BCM_COM_PROC_P20/131(V_BCM_COM_Opt_Adhesion_Out_W34) -> [V_BCM_COM_Opt_Adhesion_Out_W34]  "V_BCMA_COM_Opt_Adhesion_Out_W34"
  BCM_COM_PROC_P20/132(V_BCM_COM_Whl_AS_Adp_Gain_W12) -> [V_BCM_COM_Whl_AS_Adp_Gain_W12]  "V_BCMA_COM_Whl_AS_Adp_Gain_W12"
  BCM_COM_PROC_P20/133(V_BCM_COM_Whl_AS_Adp_Gain_W34) -> [V_BCM_COM_Whl_AS_Adp_Gain_W34]  "V_BCMA_COM_Whl_AS_Adp_Gain_W34"
  BCM_COM_PROC_P20/1(V_BCM_COM_Whl_Spun_Up_State_W12) -> Terminator34/1  "V_BCMA_COM_Whl_Spun_Up_State_W12"
  BCM_COM_PROC_P20/2(V_BCM_COM_Whl_Ref_Speed_W12) -> Terminator16/1  "V_BCMA_COM_Whl_Ref_Speed_W12"
  BCM_COM_PROC_P20/3(V_BCM_COM_Whl_Spun_Up_State_W34) -> Terminator35/1  "V_BCMA_COM_Whl_Spun_Up_State_W34"
  BCM_COM_PROC_P20/4(V_BCM_COM_Whl_Ref_Speed_W34) -> Terminator24/1  "V_BCMA_COM_Whl_Ref_Speed_W34"
  BCM_COM_PROC_P20/5(V_BCM_COM_DFCS_A_Gnd_Spd_Conv) -> Terminator23/1  "V_BCMA_COM_DFCS_A_Gnd_Spd_Conv"
  BCM_COM_PROC_P20/6(V_BCM_COM_DFCS_B_Gnd_Spd_Conv) -> Terminator26/1  "V_BCMA_COM_DFCS_B_Gnd_Spd_Conv"
  BCM_COM_PROC_P20/7(V_BCM_COM_AC_Gnd_Spd_Cons) -> Terminator42/1  "V_BCMA_COM_AC_Gnd_Spd_Cons"
  BCM_COM_PROC_P20/8(V_BCM_COM_AC_Gnd_Spd_Cons_Val) -> Terminator28/1  "V_BCMA_COM_AC_Gnd_Spd_Cons_Val"
  BCM_COM_PROC_P20/9(V_BCM_COM_DFCS_A_Long_Accel_Conv) -> Terminator43/1  "V_BCMA_COM_DFCS_A_Long_Accel_Conv"
  BCM_COM_PROC_P20/10(V_BCM_COM_DFCS_B_Long_Accel_Conv) -> Terminator40/1  "V_BCMA_COM_DFCS_B_Long_Accel_Conv"
  BCM_COM_PROC_P20/11(V_BCM_COM_AC_Long_Accel_Cons) -> Terminator36/1  "V_BCMA_COM_AC_Long_Accel_Cons"
  BCM_COM_PROC_P20/12(V_BCM_COM_AC_Long_Accel_Cons_Val) -> Terminator41/1  "V_BCMA_COM_AC_Long_Accel_Cons_Val"
  BCM_COM_PROC_P20/13(V_BCM_COM_AC_Long_Accel_Filt_Corr) -> Terminator53/1  "V_BCMA_COM_AC_Long_Accel_Filt_Corr"
  BCM_COM_PROC_P20/14(V_BCM_COM_AC_Pitch_Ang_Cons_Val) -> Terminator46/1  "V_BCMA_COM_AC_Pitch_Ang_Cons_Val"
  BCM_COM_PROC_P20/15(V_BCM_COM_AC_Pitch_Ang_Filt) -> Terminator54/1  "V_BCMA_COM_AC_Pitch_Ang_Filt"
  BCM_COM_PROC_P20/16(V_BCM_COM_AC_Pitch_Ang_Cons) -> Terminator50/1  "V_BCMA_COM_AC_Pitch_Ang_Cons"
  BCM_COM_PROC_P20/17(V_BCM_COM_DFCS_A_WOWs_Val_Cons) -> Terminator47/1  "V_BCMA_COM_DFCS_A_WOWs_Val_Cons"
  BCM_COM_PROC_P20/18(V_BCM_COM_DFCS_B_WOWs_Val_Cons) -> Terminator51/1  "V_BCMA_COM_DFCS_B_WOWs_Val_Cons"
  BCM_COM_PROC_P20/19(V_BCM_COM_LMLG_WOWs_Cons) -> Terminator58/1  "V_BCMA_COM_LMLG_WOWs_Cons"
  BCM_COM_PROC_P20/20(V_BCM_COM_LMLG_WOWs_Cons_Val) -> Terminator52/1  "V_BCMA_COM_LMLG_WOWs_Cons_Val"
  BCM_COM_PROC_P20/21(V_BCM_COM_RMLG_WOWs_Cons) -> Terminator59/1  "V_BCMA_COM_RMLG_WOWs_Cons"
  BCM_COM_PROC_P20/22(V_BCM_COM_RMLG_WOWs_Cons_Val) -> Terminator56/1  "V_BCMA_COM_RMLG_WOWs_Cons_Val"
  BCM_COM_PROC_P20/23(V_BCM_COM_NLG_WOWs_Cons) -> Terminator55/1  "V_BCMA_COM_NLG_WOWs_Cons"
  BCM_COM_PROC_P20/24(V_BCM_COM_NLG_WOWs_Cons_Val) -> Terminator57/1  "V_BCMA_COM_NLG_WOWs_Cons_Val"
  BCM_COM_PROC_P20/25(V_BCM_COM_LMLG_On_Gnd_State) -> Terminator65/1  "V_BCMA_COM_LMLG_On_Gnd_State"
  BCM_COM_PROC_P20/26(V_BCM_COM_RMLG_On_Gnd_State) -> Terminator60/1  "V_BCMA_COM_RMLG_On_Gnd_State"
  BCM_COM_PROC_P20/27(V_BCM_COM_LMLG_On_Gnd_State_Val) -> Terminator66/1  "V_BCMA_COM_LMLG_On_Gnd_State_Val"
  BCM_COM_PROC_P20/28(V_BCM_COM_RMLG_On_Gnd_State_Val) -> Terminator62/1  "V_BCMA_COM_RMLG_On_Gnd_State_Val"
  BCM_COM_PROC_P20/29(V_BCM_COM_MLG_On_Gnd_State) -> Terminator61/1  "V_BCMA_COM_MLG_On_Gnd_State"
  BCM_COM_PROC_P20/30(V_BCM_COM_NLG_On_Gnd_State) -> Terminator63/1  "V_BCMA_COM_NLG_On_Gnd_State"
  BCM_COM_PROC_P20/31(V_BCM_COM_NLG_On_Gnd_State_Val) -> Terminator70/1  "V_BCMA_COM_NLG_On_Gnd_State_Val"
  BCM_COM_PROC_P20/32(V_BCM_COM_NLG_On_Gnd_State_Cons) -> Terminator64/1  "V_BCMA_COM_NLG_On_Gnd_State_Cons"
  BCM_COM_PROC_P20/36(V_BCM_COM_Decel_Law_Inhib_Cons_Val) -> Terminator69/1  "V_BCMA_COM_Decel_Law_Inhib_Cons_Val"
  BCM_COM_PROC_P20/37(V_BCM_COM_TLA_State_Cons) -> Terminator90/1  "V_BCMA_COM_TLA_State_Cons"
  BCM_COM_PROC_P20/38(V_BCM_COM_TLA_State_Cons_Val) -> Terminator72/1  "V_BCMA_COM_TLA_State_Cons_Val"
  BCM_COM_PROC_P20/39(V_BCM_COM_LG_Lever_Up_Conf) -> Terminator96/1  "V_BCMA_COM_LG_Lever_Up_Conf"
  BCM_COM_PROC_P20/40(V_BCM_COM_LG_Lever_State_Cons) -> Terminator86/1  "V_BCMA_COM_LG_Lever_State_Cons"
  BCM_COM_PROC_P20/41(V_BCM_COM_LG_Lever_Ste_Cons_Val) -> Terminator73/1  "V_BCMA_COM_LG_Lever_Ste_Cons_Val"
  BCM_COM_PROC_P20/42(V_BCM_COM_LMLG_Downlock_Conf) -> Terminator87/1  "V_BCMA_COM_LMLG_Downlock_Conf"
  BCM_COM_PROC_P20/43(V_BCM_COM_RMLG_Downlock_Conf) -> Terminator110/1  "V_BCMA_COM_RMLG_Downlock_Conf"
  BCM_COM_PROC_P20/44(V_BCM_COM_LMLG_Downlock_State) -> Terminator88/1  "V_BCMA_COM_LMLG_Downlock_State"
  BCM_COM_PROC_P20/45(V_BCM_COM_LMLG_Dnlk_State_Val) -> Terminator119/1  "V_BCMA_COM_LMLG_Dnlk_State_Val"
  BCM_COM_PROC_P20/46(V_BCM_COM_RMLG_Downlock_State) -> Terminator106/1  "V_BCMA_COM_RMLG_Downlock_State"
  BCM_COM_PROC_P20/47(V_BCM_COM_RMLG_Dnlk_State_Val) -> Terminator102/1  "V_BCMA_COM_RMLG_Dnlk_State_Val"
  BCM_COM_PROC_P20/49(V_BCM_COM_SELV_Low_Speed_Logic) -> Terminator143/1  "V_BCMA_COM_SELV_Low_Speed_Logic"
  BCM_COM_PROC_P20/50(V_BCM_COM_Engine_State) -> Terminator67/1  "V_BCMA_COM_Engine_State"
  BCM_COM_PROC_P20/51(V_BCM_COM_Engine_State_Val) -> Terminator146/1  "V_BCMA_COM_Engine_State_Val"
  BCM_COM_PROC_P20/52(V_BCM_COM_LH_Braking_Cmd_State) -> Terminator71/1  "V_BCMA_COM_LH_Braking_Cmd_State"
  BCM_COM_PROC_P20/53(V_BCM_COM_RH_Braking_Cmd_State) -> Terminator68/1  "V_BCMA_COM_RH_Braking_Cmd_State"
  BCM_COM_PROC_P20/54(V_BCM_COM_LH_Regular_Brkg_Press_Cmd) -> Terminator109/1  "V_BCMA_COM_LH_Regular_Brkg_Press_Cmd"
  BCM_COM_PROC_P20/55(V_BCM_COM_RH_Regular_Brkg_Press_Cmd) -> Terminator147/1  "V_BCMA_COM_RH_Regular_Brkg_Press_Cmd"
  BCM_COM_PROC_P20/56(V_BCM_COM_Wheels_Global_Spun_Up_Ste) -> [V_BCM_COM_Wheels_Global_Spun_Up_Ste]  "V_BCMA_COM_Wheels_Global_Spun_Up_Ste"
  BCM_COM_PROC_P20/57(V_BCM_COM_Global_Reference_Spd) -> [V_BCM_COM_Global_Reference_Spd]  "V_BCMA_COM_Global_Reference_Spd"
  BCM_COM_PROC_P20/59(V_BCM_COM_LMLG_Global_Wheel_Spd) -> Terminator30/1  "V_BCMA_COM_LMLG_Global_Wheel_Spd"
  BCM_COM_PROC_P20/60(V_BCM_COM_RMLG_Global_Wheel_Spd) -> Terminator76/1  "V_BCMA_COM_RMLG_Global_Wheel_Spd"
  BCM_COM_PROC_P20/64(v_BCM_COM_FT_Seq) -> Terminator33/1  "V_BCMA_COM_FT_Seq"
  BCM_COM_PROC_P20/65(V_BCM_COM_Start_Norm_FT_Cond) -> Terminator31/1  "V_BCMA_COM_Start_Norm_FT_Cond"
  BCM_COM_PROC_P20/66(V_BCM_COM_Brkg_Norm_FT_Prog_Sts) -> Terminator75/1  "V_BCMA_COM_Brkg_Norm_FT_Prog_Sts"
  BCM_COM_PROC_P20/67(V_BCM_COM_Brkg_Norm_FT_Cond) -> Terminator74/1  "V_BCMA_COM_Brkg_Norm_FT_Cond"
  BCM_COM_PROC_P20/68(V_BCM_COM_Braking_Norm_FT_Seq) -> [V_BCM_COM_Braking_Norm_FT_Seq]  "V_BCMA_COM_Braking_Norm_FT_Seq"
  BCM_COM_PROC_P20/69(V_BCM_COM_Abort_Norm_FT_Cond) -> Terminator32/1  "V_BCMA_COM_Abort_Norm_FT_Cond"
  BCM_COM_PROC_P20/70(V_BCM_COM_Brkg_Alt_FT_Prog_Sts) -> Terminator19/1  "V_BCMA_COM_Brkg_Alt_FT_Prog_Sts"
  BCM_COM_PROC_P20/74(V_BCM_COM_Brkg_Alt_FT_Cond) -> Terminator91/1  "V_BCMA_COM_Brkg_Alt_FT_Cond"
  BCM_COM_PROC_P20/72(V_BCM_COM_Abort_Alt_FT_Cond) -> Terminator89/1  "V_BCMA_COM_Abort_Alt_FT_Cond"
  BCM_COM_PROC_P20/73(V_BCM_COM_Start_Alt_FT_Cond) -> Terminator92/1  "V_BCMA_COM_Start_Alt_FT_Cond"
  BCM_COM_PROC_P20/77(V_BCM_COM_LH_Press_Law_Brkg_Press_Cmd) -> [V_BCM_COM_LH_Press_Law_Brkg_Press_Cmd]  "V_BCMA_COM_LH_Press_Law_Brkg_Press_Cmd"
  BCM_COM_PROC_P20/78(V_BCM_COM_RH_Press_Law_Brkg_Press_Cmd) -> [V_BCM_COM_RH_Press_Law_Brkg_Press_Cmd]  "V_BCMA_COM_RH_Press_Law_Brkg_Press_Cmd"
  BCM_COM_PROC_P20/79(V_BCM_COM_LH_FT_Press_Cmd) -> Terminator84/1  "V_BCMA_COM_LH_FT_Press_Cmd"
  BCM_COM_PROC_P20/80(V_BCM_COM_RH_FT_Press_Cmd) -> Terminator83/1  "V_BCMA_COM_RH_FT_Press_Cmd"
  BCM_COM_PROC_P20/81(V_BCM_COM_LH_Ret_Brkg_Press_Cmd) -> Terminator77/1  "V_BCMA_COM_LH_Ret_Brkg_Press_Cmd"
  BCM_COM_PROC_P20/82(V_BCM_COM_RH_Ret_Brkg_Press_Cmd) -> Terminator80/1  "V_BCMA_COM_RH_Ret_Brkg_Press_Cmd"
  BCM_COM_PROC_P20/83(V_BCM_COM_LH_Eng_Run_Press_Cmd) -> Terminator78/1  "V_BCMA_COM_LH_Eng_Run_Press_Cmd"
  BCM_COM_PROC_P20/84(V_BCM_COM_RH_Eng_Run_Press_Cmd) -> Terminator94/1  "V_BCMA_COM_RH_Eng_Run_Press_Cmd"
  BCM_COM_PROC_P20/85(V_BCM_COM_Brkg_SELV_High_Side_FT_Cmd_Order) -> Terminator93/1  "V_BCMA_COM_Brkg_SELV_High_Side_FT_Cmd_Order"
  BCM_COM_PROC_P20/86(V_BCM_COM_DBCU_FT_Inhib_Order) -> Terminator95/1  "V_BCMA_COM_DBCU_FT_Inhib_Order"
  BCM_COM_PROC_P20/89(V_BCM_COM_Alt_Sw_Cmd_Cons) -> Terminator104/1  "V_BCMA_COM_Alt_Sw_Cmd_Cons"
  BCM_COM_PROC_P20/90(V_BCM_COM_Alt_Sw_Cmd_Cons_Val) -> Terminator100/1  "V_BCMA_COM_Alt_Sw_Cmd_Cons_Val"
  BCM_COM_PROC_P20/91(V_BCM_COM_Disp_Sw_Cmd_Cons) -> Terminator107/1  "V_BCMA_COM_Disp_Sw_Cmd_Cons"
  BCM_COM_PROC_P20/92(V_BCM_COM_Disp_Sw_Cmd_Cons_Val) -> Terminator105/1  "V_BCMA_COM_Disp_Sw_Cmd_Cons_Val"
  BCM_COM_PROC_P20/93(V_BCM_COM_MP_BCMA_Alt_Disp_Sw_Conf) -> Terminator98/1  "V_BCMA_COM_MP_BCMA_Alt_Disp_Sw_Conf"
  BCM_COM_PROC_P20/96(V_BCM_COM_Norm_Brkg_Availability) -> [V_BCM_COM_Norm_Brkg_Availability]  "V_BCMA_COM_Norm_Brkg_Availability"
  BCM_COM_PROC_P20/97(V_BCM_COM_Alt_Brkg_Availability) -> Terminator108/1  "V_BCMA_COM_Alt_Brkg_Availability"
  BCM_COM_PROC_P20/98(V_BCM_COM_Braking_Type) -> Terminator113/1  "V_BCMA_COM_Braking_Type"
  BCM_COM_PROC_P20/102(V_BCM_COM_PBSELV_ON_POS_Conf) -> Terminator101/1  "V_BCMA_COM_PBSELV_ON_POS_Conf"
  BCM_COM_PROC_P20/101(V_BCM_COM_Press_Cmd_Rate_Lim) -> Terminator99/1  "V_BCMA_COM_Press_Cmd_Rate_Lim"
  BCM_COM_PROC_P20/104(V_BCM_COM_PBSELV_State_Cons_Val) -> Terminator118/1  "V_BCMA_COM_PBSELV_State_Cons_Val"
  BCM_COM_PROC_P20/105(V_BCM_COM_Hyd_A_Press_Cons) -> Terminator116/1  "V_BCMA_COM_Hyd_A_Press_Cons"
  BCM_COM_PROC_P20/106(V_BCM_COM_Hyd_B_Press_Cons) -> Terminator123/1  "V_BCMA_COM_Hyd_B_Press_Cons"
  BCM_COM_PROC_P20/107(V_BCM_COM_Hyd_A_Press_Cons_Val) -> Terminator120/1  "V_BCMA_COM_Hyd_A_Press_Cons_Val"
  BCM_COM_PROC_P20/108(V_BCM_COM_Hyd_B_Press_Cons_Val) -> Terminator114/1  "V_BCMA_COM_Hyd_B_Press_Cons_Val"
  BCM_COM_PROC_P20/109(V_BCM_COM_Hyd_A_Press_State) -> Terminator117/1  "V_BCMA_COM_Hyd_A_Press_State"
  BCM_COM_PROC_P20/110(V_BCM_COM_Hyd_B_Press_State) -> Terminator115/1  "V_BCMA_COM_Hyd_B_Press_State"
  BCM_COM_PROC_P20/111(V_BCM_COM_Sys_Sanc_Inhib_During_FT) -> Terminator125/1  "V_BCMA_COM_Sys_Sanc_Inhib_During_FT"
  BCM_COM_PROC_P20/123(V_BCM_COM_Automate_State_W34) -> Terminator126/1  "V_BCMA_COM_Automate_State_W34"
  BCM_COM_PROC_P20/122(V_BCM_COM_Automate_State_W12) -> Terminator124/1  "V_BCMA_COM_Automate_State_W12"
  BCM_COM_PROC_P20/127(V_BCM_COM_Target_Decel_Out_W34) -> Terminator128/1  "V_BCMA_COM_Target_Decel_Out_W34"
  BCM_COM_PROC_P20/126(V_BCM_COM_Target_Decel_Out_W12) -> Terminator127/1  "V_BCMA_COM_Target_Decel_Out_W12"
  BCM_COM_PROC_P20/166(V_BCM_COM_DFCS_A_RMLG_WOWs_Val1) -> Terminator164/1  "V_BCMA_COM_DFCS_A_RMLG_WOWs_Val"
  BCM_COM_PROC_P20/167(V_BCM_COM_DFCS_A_NLG_WOWs_Val1) -> Terminator4/1  "V_BCMA_COM_DFCS_A_NLG_WOWs_Val"
  BCM_COM_PROC_P20/168(V_BCM_COM_DFCS_A_WOWs_Val_Val1) -> Terminator166/1  "V_BCMA_COM_DFCS_A_WOWs_Val_Val"
  BCM_COM_PROC_P20/169(V_BCM_COM_DFCS_B_LMLG_WOWs_Val1) -> Terminator165/1  "V_BCMA_COM_DFCS_B_LMLG_WOWs_Val"
  BCM_COM_PROC_P20/170(V_BCM_COM_DFCS_B_RMLG_WOWs_Val1) -> Terminator2/1  "V_BCMA_COM_DFCS_B_RMLG_WOWs_Val"
  BCM_COM_PROC_P20/171(V_BCM_COM_DFCS_B_NLG_WOWs_Val1) -> Terminator5/1  "V_BCMA_COM_DFCS_B_NLG_WOWs_Val"
  BCM_COM_PROC_P20/172(V_BCM_COM_DFCS_B_WOWs_Val_Val1) -> Terminator3/1  "V_BCMA_COM_DFCS_B_WOWs_Val_Val"
  BCM_COM_PROC_P20/173(V_BCM_COM_DFCS_A_LH_Braking_Cmd_Val1) -> Terminator167/1  "V_BCMA_COM_DFCS_A_LH_Braking_Cmd_Val"
  BCM_COM_PROC_P20/174(V_BCM_COM_DFCS_A_RH_Braking_Cmd_Val1) -> Terminator172/1  "V_BCMA_COM_DFCS_A_RH_Braking_Cmd_Val"
  BCM_COM_PROC_P20/175(V_BCM_COM_DFCS_B_LH_Braking_Cmd_Val1) -> Terminator170/1  "V_BCMA_COM_DFCS_B_LH_Braking_Cmd_Val"
  BCM_COM_PROC_P20/176(V_BCM_COM_DFCS_B_RH_Braking_Cmd_Val1) -> Terminator174/1  "V_BCMA_COM_DFCS_B_RH_Braking_Cmd_Val"
  BCM_COM_PROC_P20/177(V_BCM_COM_DFCS_A_DBCU_Alt_Mode_1_Val) -> Terminator173/1  "V_BCMA_COM_DFCS_A_DBCU_Alt_Mode_1_Val"
  BCM_COM_PROC_P20/178(V_BCM_COM_DFCS_A_DBCU_Alt_Mode_2_Val) -> Terminator168/1  "V_BCMA_COM_DFCS_A_DBCU_Alt_Mode_2_Val"
  BCM_COM_PROC_P20/179(V_BCM_COM_DFCS_B_DBCU_Alt_Mode_1_Val) -> Terminator171/1  "V_BCMA_COM_DFCS_B_DBCU_Alt_Mode_1_Val"
  BCM_COM_PROC_P20/180(V_BCM_COM_DFCS_B_DBCU_Alt_Mode_2_Val) -> Terminator169/1  "V_BCMA_COM_DFCS_B_DBCU_Alt_Mode_2_Val"
  BCM_COM_PROC_P20/181(V_BCM_COM_DFCS_A_TLA_Above_Idle_Val1) -> Terminator175/1  "V_BCMA_COM_DFCS_A_TLA_Above_Idle_Val"
  BCM_COM_PROC_P20/182(V_BCM_COM_DFCS_B_TLA_Above_Idle_Val1) -> Terminator180/1  "V_BCMA_COM_DFCS_B_TLA_Above_Idle_Val"
  BCM_COM_PROC_P20/183(V_BCM_COM_UTC_Time_Hours_Cons) -> Terminator178/1  "V_BCMA_COM_UTC_Time_Hours_Cons"
  BCM_COM_PROC_P20/184(V_BCM_COM_UTC_Time_Hours_Cons_Val) -> Terminator182/1  "V_BCMA_COM_UTC_Time_Hours_Cons_Val"
  BCM_COM_PROC_P20/185(V_BCM_COM_UTC_Time_Minutes_Cons) -> Terminator181/1  "V_BCMA_COM_UTC_Time_Minutes_Cons"
  BCM_COM_PROC_P20/186(V_BCM_COM_UTC_Time_Minutes_Cons_Val) -> Terminator176/1  "V_BCMA_COM_UTC_Time_Minutes_Cons_Val"
  BCM_COM_PROC_P20/187(V_BCM_COM_UTC_Time_Seconds_Cons) -> Terminator179/1  "V_BCMA_COM_UTC_Time_Seconds_Cons"
  BCM_COM_PROC_P20/188(V_BCM_COM_UTC_Time_Seconds_Cons_Val) -> Terminator177/1  "V_BCMA_COM_UTC_Time_Seconds_Cons_Val"
  BCM_COM_PROC_P20/189(V_BCM_COM_DBCU_BRK_ORDER_FAIL_Conf) -> Terminator183/1  "V_BCMA_COM_DBCU_BRK_ORDER_FAIL_Conf"
  BCM_COM_PROC_P20/190(V_BCM_COM_DBCU_DISPATCH_SW_ON_Conf) -> Terminator188/1  "V_BCMA_COM_DBCU_DISPATCH_SW_ON_Conf"
  BCM_COM_PROC_P20/191(V_BCM_COM_LH_DBCU_BRK_CMD_FDBK_Conf) -> Terminator186/1  "V_BCMA_COM_LH_DBCU_BRK_CMD_FDBK_Conf"
  BCM_COM_PROC_P20/192(V_BCM_COM_RH_DBCU_BRK_CMD_FDBK_Conf) -> Terminator190/1  "V_BCMA_COM_RH_DBCU_BRK_CMD_FDBK_Conf"
  BCM_COM_PROC_P20/193(V_BCM_COM_DBCU_FAILED_Conf) -> Terminator189/1  "V_BCMA_COM_DBCU_FAILED_Conf"
  BCM_COM_PROC_P20/194(V_BCM_COM_DBCU_ALT_MODE_Conf) -> Terminator184/1  "V_BCMA_COM_DBCU_ALT_MODE_Conf"
  BCM_COM_PROC_P20/195(V_BCM_COM_DBCU_BRK_ORDER_FAIL_Cons) -> Terminator187/1  "V_BCMA_COM_DBCU_BRK_ORDER_FAIL_Cons"
  BCM_COM_PROC_P20/196(V_BCM_COM_DBCU_BRK_ORDER_FAIL_Cons_Val) -> Terminator185/1  "V_BCMA_COM_DBCU_BRK_ORDER_FAIL_Cons_Val"
  BCM_COM_PROC_P20/197(V_BCM_COM_DBCU_DISPATCH_SW_ON_Cons) -> Terminator191/1  "V_BCMA_COM_DBCU_DISPATCH_SW_ON_Cons"
  BCM_COM_PROC_P20/134(V_BCM_COM_Adhesion_In_Cons_W12) -> Terminator133/1  "V_BCMA_COM_Adhesion_In_Cons_W12"
  BCM_COM_PROC_P20/135(V_BCM_COM_Adhesion_In_Cons_W34) -> Terminator131/1  "V_BCMA_COM_Adhesion_In_Cons_W34"
  BCM_COM_PROC_P20/136(V_BCM_COM_Opt_Adhesion_In_Cons_W12) -> Terminator135/1  "V_BCMA_COM_Opt_Adhesion_In_Cons_W12"
  BCM_COM_PROC_P20/137(V_BCM_COM_Opt_Adhesion_In_Cons_W34) -> Terminator134/1  "V_BCMA_COM_Opt_Adhesion_In_Cons_W34"
  BCM_COM_PROC_P20/138(V_BCM_COM_Target_Speed_In_Cons_W12) -> Terminator129/1  "V_BCMA_COM_Target_Speed_In_Cons_W12"
  BCM_COM_PROC_P20/139(V_BCM_COM_Target_Speed_In_Cons_W34) -> Terminator132/1  "V_BCMA_COM_Target_Speed_In_Cons_W34"
  BCM_COM_PROC_P20/140(V_BCM_COM_Big_Slip_WD_Trig_In_Cons_W12) -> Terminator130/1  "V_BCMA_COM_Big_Slip_WD_Trig_In_Cons_W12"
  BCM_COM_PROC_P20/141(V_BCM_COM_Big_Slip_WD_Trig_In_Cons_W34) -> Terminator136/1  "V_BCMA_COM_Big_Slip_WD_Trig_In_Cons_W34"
  BCM_COM_PROC_P20/142(V_BCM_COM_Big_Gamma_Trig_In_Cons_W12) -> Terminator141/1  "V_BCMA_COM_Big_Gamma_Trig_In_Cons_W12"
  BCM_COM_PROC_P20/143(V_BCM_COM_Big_Gamma_Trig_In_Cons_W34) -> Terminator139/1  "V_BCMA_COM_Big_Gamma_Trig_In_Cons_W34"
  BCM_COM_PROC_P20/144(V_BCM_COM_Small_Slip_Trig_In_Cons_W12) -> Terminator144/1  "V_BCMA_COM_Small_Slip_Trig_In_Cons_W12"
  BCM_COM_PROC_P20/145(V_BCM_COM_Small_Slip_Trig_In_Cons_W34) -> Terminator142/1  "V_BCMA_COM_Small_Slip_Trig_In_Cons_W34"
  BCM_COM_PROC_P20/146(V_BCM_COM_Big_Slip_Trig_In_Cons_W12) -> Terminator137/1  "V_BCMA_COM_Big_Slip_Trig_In_Cons_W12"
  BCM_COM_PROC_P20/147(V_BCM_COM_Big_Slip_Trig_In_Cons_W34) -> Terminator140/1  "V_BCMA_COM_Big_Slip_Trig_In_Cons_W34"
  BCM_COM_PROC_P20/148(V_BCM_COM_CCDL_Data_From_Opp_BCM_Val) -> Terminator138/1  "V_BCMA_COM_CCDL_Data_From_Opp_BCM_Val"
  BCM_COM_PROC_P20/149(V_BCM_COM_DBCU_Inhibition_Order_From_Opp_BCM_Cons) -> Terminator145/1  "V_BCMA_COM_DBCU_Inhibition_Order_From_Opp_BCM_Cons"
  BCM_COM_PROC_P20/150(V_BCM_COM_DBCU_Inhibition_Order_From_Opp_BCM_Cons_Val) -> Terminator152/1  "V_BCMA_COM_DBCU_Inhibition_Order_From_Opp_BCM_Cons_Val"
  BCM_COM_PROC_P20/151(V_BCM_COM_Engine_Running_Conf_Flt) -> Terminator150/1  "V_BCMA_COM_Engine_Running_Conf_Flt"
  BCM_COM_PROC_P20/152(V_BCM_COM_Engine_Running_Unconf_Flt) -> Terminator154/1  "V_BCMA_COM_Engine_Running_Unconf_Flt"
  BCM_COM_PROC_P20/153(V_BCM_COM_Hyd_A_Press_Conf_Flt) -> Terminator153/1  "V_BCMA_COM_Hyd_A_Press_Conf_Flt"
  BCM_COM_PROC_P20/154(V_BCM_COM_Hyd_B_Press_Conf_Flt) -> Terminator148/1  "V_BCMA_COM_Hyd_B_Press_Conf_Flt"
  BCM_COM_PROC_P20/155(V_BCM_COM_Hyd_A_Press_Unconf_Flt) -> Terminator151/1  "V_BCMA_COM_Hyd_A_Press_Unconf_Flt"
  BCM_COM_PROC_P20/156(V_BCM_COM_Hyd_B_Press_Unconf_Flt) -> Terminator149/1  "V_BCMA_COM_Hyd_B_Press_Unconf_Flt"
  BCM_COM_PROC_P20/157(V_BCM_COM_DFCS_A_AC_Gnd_Spd_Val) -> Terminator155/1  "V_BCMA_COM_DFCS_A_AC_Gnd_Spd_Val"
  BCM_COM_PROC_P20/158(V_BCM_COM_DFCS_A_AC_Long_Accel_Val1) -> Terminator160/1  "V_BCMA_COM_DFCS_A_AC_Long_Accel_Val"
  BCM_COM_PROC_P20/159(V_BCM_COM_DFCS_A_AC_Pitch_Angle_Val1) -> Terminator158/1  "V_BCMA_COM_DFCS_A_AC_Pitch_Angle_Val"
  BCM_COM_PROC_P20/160(V_BCM_COM_DFCS_A_Decel_Law_Inhib_Val1) -> Terminator162/1  "V_BCMA_COM_DFCS_A_Decel_Law_Inhib_Val"
  BCM_COM_PROC_P20/161(V_BCM_COM_DFCS_B_Decel_Law_Inhib_Val1) -> Terminator161/1  "V_BCMA_COM_DFCS_B_Decel_Law_Inhib_Val"
  BCM_COM_PROC_P20/162(V_BCM_COM_DFCS_B_AC_Gnd_Spd_Val) -> Terminator156/1  "V_BCMA_COM_DFCS_B_AC_Gnd_Spd_Val"
  BCM_COM_PROC_P20/163(V_BCM_COM_DFCS_B_AC_Long_Accel_Val1) -> Terminator159/1  "V_BCMA_COM_DFCS_B_AC_Long_Accel_Val"
  BCM_COM_PROC_P20/164(V_BCM_COM_DFCS_B_AC_Pitch_Angle_Val1) -> Terminator157/1  "V_BCMA_COM_DFCS_B_AC_Pitch_Angle_Val"
  BCM_COM_PROC_P20/165(V_BCM_COM_DFCS_A_LMLG_WOWs_Val1) -> Terminator163/1  "V_BCMA_COM_DFCS_A_LMLG_WOWs_Val"
  BCM_COM_PROC_P20/230(V_BCM_COM_RMLG_Outboard_Tire_Press_Cons) -> Terminator224/1  "V_BCMA_COM_RMLG_Outboard_Tire_Press_Cons"
  BCM_COM_PROC_P20/231(V_BCM_COM_RMLG_Outboard_Tire_Press_Cons_Val) -> Terminator254/1  "V_BCMA_COM_RMLG_Outboard_Tire_Press_Cons_Val"
  BCM_COM_PROC_P20/232(V_BCM_COM_A429_SSM_Avionics_Label_005) -> [V_BCM_COM_A429_SSM_Avionics_Label_005]  "V_BCMA_COM_A429_SSM_Avionics_Label_005"
  BCM_COM_PROC_P20/233(V_BCM_COM_A429_SSM_Avionics_Label_006) -> [V_BCM_COM_A429_SSM_Avionics_Label_006]  "V_BCMA_COM_A429_SSM_Avionics_Label_006"
  BCM_COM_PROC_P20/234(V_BCM_COM_A429_SSM_Avionics_Label_021) -> [V_BCM_COM_A429_SSM_Avionics_Label_021]  "V_BCMA_COM_A429_SSM_Avionics_Label_021"
  BCM_COM_PROC_P20/235(V_BCM_COM_A429_SSM_Avionics_Label_022) -> [V_BCM_COM_A429_SSM_Avionics_Label_022]  "V_BCMA_COM_A429_SSM_Avionics_Label_022"
  BCM_COM_PROC_P20/236(V_BCM_COM_A429_SSM_Avionics_Label_030) -> [V_BCM_COM_A429_SSM_Avionics_Label_030]  "V_BCMA_COM_A429_SSM_Avionics_Label_030"
  BCM_COM_PROC_P20/237(V_BCM_COM_A429_SSM_Avionics_Label_031) -> [V_BCM_COM_A429_SSM_Avionics_Label_031]  "V_BCMA_COM_A429_SSM_Avionics_Label_031"
  BCM_COM_PROC_P20/238(V_BCM_COM_A429_SSM_Avionics_Label_032) -> [V_BCM_COM_A429_SSM_Avionics_Label_032]  "V_BCMA_COM_A429_SSM_Avionics_Label_032"
  BCM_COM_PROC_P20/239(V_BCM_COM_A429_SSM_Avionics_Label_033) -> [V_BCM_COM_A429_SSM_Avionics_Label_033]  "V_BCMA_COM_A429_SSM_Avionics_Label_033"
  BCM_COM_PROC_P20/240(V_BCM_COM_A429_SSM_Avionics_Label_040) -> [V_BCM_COM_A429_SSM_Avionics_Label_040]  "V_BCMA_COM_A429_SSM_Avionics_Label_040"
  BCM_COM_PROC_P20/241(V_BCM_COM_A429_SSM_Avionics_Label_041) -> [V_BCM_COM_A429_SSM_Avionics_Label_041]  "V_BCMA_COM_A429_SSM_Avionics_Label_041"
  BCM_COM_PROC_P20/242(V_BCM_COM_A429_SSM_Avionics_Label_042) -> [V_BCM_COM_A429_SSM_Avionics_Label_042]  "V_BCMA_COM_A429_SSM_Avionics_Label_042"
  BCM_COM_PROC_P20/243(V_BCM_COM_A429_SSM_Avionics_Label_043) -> [V_BCM_COM_A429_SSM_Avionics_Label_043]  "V_BCMA_COM_A429_SSM_Avionics_Label_043"
  BCM_COM_PROC_P20/244(V_BCM_COM_A429_SSM_Avionics_Label_050) -> [V_BCM_COM_A429_SSM_Avionics_Label_050]  "V_BCMA_COM_A429_SSM_Avionics_Label_050"
  BCM_COM_PROC_P20/245(V_BCM_COM_A429_SSM_DFCS_Label_105) -> [V_BCM_COM_A429_SSM_DFCS_Label_105]  "V_BCMA_COM_A429_SSM_DFCS_Label_105"
  BCM_COM_PROC_P20/246(V_BCM_COM_A429_Wheel_Speed_W12) -> [V_BCM_COM_A429_Wheel_Speed_W12]  "V_BCMA_COM_A429_Wheel_Speed_W12"
  BCM_COM_PROC_P20/247(V_BCM_COM_A429_Wheel_Speed_W34) -> [V_BCM_COM_A429_Wheel_Speed_W34]  "V_BCMA_COM_A429_Wheel_Speed_W34"
  BCM_COM_PROC_P20/248(V_BCM_COM_A429_TACHO_Fail_W12) -> [V_BCM_COM_A429_TACHO_Fail_W12]  "V_BCMA_COM_A429_TACHO_Fail_W12"
  BCM_COM_PROC_P20/249(V_BCM_COM_A429_TACHO_Fail_W34) -> [V_BCM_COM_A429_TACHO_Fail_W34]  "V_BCMA_COM_A429_TACHO_Fail_W34"
  BCM_COM_PROC_P20/250(V_BCM_COM_A429_SSM_Avionics_Label_001) -> [V_BCM_COM_A429_SSM_Avionics_Label_001]  "V_BCMA_COM_A429_SSM_Avionics_Label_001"
  BCM_COM_PROC_P20/251(V_BCM_COM_A429_SSM_Avionics_Label_002) -> [V_BCM_COM_A429_SSM_Avionics_Label_002]  "V_BCMA_COM_A429_SSM_Avionics_Label_002"
  BCM_COM_PROC_P20/252(V_BCM_COM_A429_SSM_Avionics_Label_003) -> [V_BCM_COM_A429_SSM_Avionics_Label_003]  "V_BCMA_COM_A429_SSM_Avionics_Label_003"
  BCM_COM_PROC_P20/253(V_BCM_COM_A429_SSM_Avionics_Label_004) -> [V_BCM_COM_A429_SSM_Avionics_Label_004]  "V_BCMA_COM_A429_SSM_Avionics_Label_004"
  BCM_COM_PROC_P20/254(V_BCM_COM_A429_SSM_DFCS_Label_101) -> [V_BCM_COM_A429_SSM_DFCS_Label_101]  "V_BCMA_COM_A429_SSM_DFCS_Label_101"
  BCM_COM_PROC_P20/255(V_BCM_COM_A429_SSM_DFCS_Label_102) -> [V_BCM_COM_A429_SSM_DFCS_Label_102]  "V_BCMA_COM_A429_SSM_DFCS_Label_102"
  BCM_COM_PROC_P20/256(V_BCM_COM_A429_SSM_DFCS_Label_103) -> [V_BCM_COM_A429_SSM_DFCS_Label_103]  "V_BCMA_COM_A429_SSM_DFCS_Label_103"
  BCM_COM_PROC_P20/257(V_BCM_COM_A429_SSM_DFCS_Label_104) -> [V_BCM_COM_A429_SSM_DFCS_Label_104]  "V_BCMA_COM_A429_SSM_DFCS_Label_104"
  BCM_COM_PROC_P20/258(V_BCM_COM_A429_LH_Brake_Temp) -> [V_BCM_COM_A429_LH_Brake_Temp]  "V_BCMA_COM_A429_LH_Brake_Temp"
  BCM_COM_PROC_P20/259(V_BCM_COM_A429_RH_Brake_Temp) -> [V_BCM_COM_A429_RH_Brake_Temp]  "V_BCMA_COM_A429_RH_Brake_Temp"
  BCM_COM_PROC_P20/260(V_BCM_COM_A429_LH_Brake_Temp_Sensor_Fail) -> [V_BCM_COM_A429_LH_Brake_Temp_Sensor_Fail]  "V_BCMA_COM_A429_LH_Brake_Temp_Sensor_Fail"
  BCM_COM_PROC_P20/261(V_BCM_COM_A429_RH_Brake_Temp_Sensor_Fail) -> [V_BCM_COM_A429_RH_Brake_Temp_Sensor_Fail]  "V_BCMA_COM_A429_RH_Brake_Temp_Sensor_Fail"
  BCM_COM_PROC_P20/294(V_BCM_COM_A429_SELV_Disc_Sts_Rdbk_Val) -> [V_BCM_COM_A429_SELV_Disc_Sts_Rdbk_Val]  "V_BCMA_COM_A429_SELV_Disc_Sts_Rdbk_Val"
  BCM_COM_PROC_P20/295(V_BCM_COM_A429_SELV_Fail) -> [V_BCM_COM_A429_SELV_Fail]  "V_BCMA_COM_A429_SELV_Fail"
  BCM_COM_PROC_P20/296(V_BCM_COM_A429_SSM_Avionics_Label_020) -> [V_BCM_COM_A429_SSM_Avionics_Label_020]  "V_BCMA_COM_A429_SSM_Avionics_Label_020"
  BCM_COM_PROC_P20/297(V_BCM_COM_A429_SSM_Avionics_Label_036) -> [V_BCM_COM_A429_SSM_Avionics_Label_036]  "V_BCMA_COM_A429_SSM_Avionics_Label_036"
  BCM_COM_PROC_P20/298(V_BCM_COM_A429_SSM_Avionics_Label_037) -> [V_BCM_COM_A429_SSM_Avionics_Label_037]  "V_BCMA_COM_A429_SSM_Avionics_Label_037"
  BCM_COM_PROC_P20/299(V_BCM_COM_A429_SSM_DFCS_Label_106) -> [V_BCM_COM_A429_SSM_DFCS_Label_106]  "V_BCMA_COM_A429_SSM_DFCS_Label_106"
  BCM_COM_PROC_P20/300(V_BCM_COM_A429_SSM_DFCS_Label_107) -> [V_BCM_COM_A429_SSM_DFCS_Label_107]  "V_BCMA_COM_A429_SSM_DFCS_Label_107"
  BCM_COM_PROC_P20/301(V_BCM_COM_A429_SSM_Avionics_Label_034) -> [V_BCM_COM_A429_SSM_Avionics_Label_034]  "V_BCMA_COM_A429_SSM_Avionics_Label_034"
  BCM_COM_PROC_P20/302(V_BCM_COM_A429_SSM_Avionics_Label_035) -> [V_BCM_COM_A429_SSM_Avionics_Label_035]  "V_BCMA_COM_A429_SSM_Avionics_Label_035"
  BCM_COM_PROC_P20/303(V_BCM_COM_A429_Park_Brake_ON) -> [V_BCM_COM_A429_Park_Brake_ON]  "V_BCMA_COM_A429_Park_Brake_ON"
  BCM_COM_PROC_P20/304(V_BCM_COM_A429_Park_Brake_Fail) -> [V_BCM_COM_A429_Park_Brake_Fail]  "V_BCMA_COM_A429_Park_Brake_Fail"
  BCM_COM_PROC_P20/305(V_BCM_COM_A429_Norm_FT_In_Progress) -> [V_BCM_COM_A429_Norm_FT_In_Progress]  "V_BCMA_COM_A429_Norm_FT_In_Progress"
  BCM_COM_PROC_P20/306(V_BCM_COM_A429_Alt_FT_In_Progress) -> [V_BCM_COM_A429_Alt_FT_In_Progress]  "V_BCMA_COM_A429_Alt_FT_In_Progress"
  BCM_COM_PROC_P20/307(V_BCM_COM_A429_Alt_FT_DFCS_Brkg_Req) -> [V_BCM_COM_A429_Alt_FT_DFCS_Brkg_Req]  "V_BCMA_COM_A429_Alt_FT_DFCS_Brkg_Req"
  BCM_COM_PROC_P20/308(V_BCM_COM_A429_Brk_Residual_Press) -> [V_BCM_COM_A429_Brk_Residual_Press]  "V_BCMA_COM_A429_Brk_Residual_Press"
  BCM_COM_PROC_P20/309(V_BCM_COM_A429_PLT_Not_Performed) -> [V_BCM_COM_A429_PLT_Not_Performed]  "V_BCMA_COM_A429_PLT_Not_Performed"
  BCM_COM_PROC_P20/310(V_BCM_COM_A429_Avionics_Comm_Fail_RX) -> [V_BCM_COM_A429_Avionics_Comm_Fail_RX]  "V_BCMA_COM_A429_Avionics_Comm_Fail_RX"
  BCM_COM_PROC_P20/311(V_BCM_COM_A429_DFCS_Decel_Law_Inhib) -> [V_BCM_COM_A429_DFCS_Decel_Law_Inhib]  "V_BCMA_COM_A429_DFCS_Decel_Law_Inhib"
  BCM_COM_PROC_P20/312(V_BCM_COM_A429_LH_Brkg_Cmd_Fdbk) -> [V_BCM_COM_A429_LH_Brkg_Cmd_Fdbk]  "V_BCMA_COM_A429_LH_Brkg_Cmd_Fdbk"
  BCM_COM_PROC_P20/313(V_BCM_COM_A429_RH_Brkg_Cmd_Fdbk) -> [V_BCM_COM_A429_RH_Brkg_Cmd_Fdbk]  "V_BCMA_COM_A429_RH_Brkg_Cmd_Fdbk"
  BCM_COM_PROC_P20/314(V_BCM_COM_A429_DFCS_LH_Brk_Pdl_Ord_Fail) -> [V_BCM_COM_A429_LH_Brk_Pdl_Ord_Fail]  "V_BCMA_COM_A429_DFCS_LH_Brk_Pdl_Ord_Fail"
  BCM_COM_PROC_P20/315(V_BCM_COM_A429_DFCS_RH_Brk_Pdl_Ord_Fail) -> [V_BCM_COM_A429_RH_Brk_Pdl_Ord_Fail]  "V_BCMA_COM_A429_DFCS_RH_Brk_Pdl_Ord_Fail"
  BCM_COM_PROC_P20/316(V_BCM_COM_A429_DFCS_A_Comm_Fail_RX) -> [V_BCM_COM_A429_DFCS_A_Comm_Fail_RX]  "V_BCMA_COM_A429_DFCS_A_Comm_Fail_RX"
  BCM_COM_PROC_P20/317(V_BCM_COM_A429_DFCS_B_Comm_Fail_RX) -> [V_BCM_COM_A429_DFCS_B_Comm_Fail_RX]  "V_BCMA_COM_A429_DFCS_B_Comm_Fail_RX"
  BCM_COM_PROC_P20/318(V_BCM_COM_A429_DFCS_A_Capsule_Fail) -> [V_BCM_COM_A429_DFCS_A_Capsule_Fail]  "V_BCMA_COM_A429_DFCS_A_Capsule_Fail"
  BCM_COM_PROC_P20/319(V_BCM_COM_A429_DFCS_B_Capsule_Fail) -> [V_BCM_COM_A429_DFCS_B_Capsule_Fail]  "V_BCMA_COM_A429_DFCS_B_Capsule_Fail"
  BCM_COM_PROC_P20/320(V_BCM_COM_A429_Pinprog_1) -> [V_BCM_COM_A429_Pinprog_1]  "V_BCMA_COM_A429_Pinprog_1"
  BCM_COM_PROC_P20/321(V_BCM_COM_A429_Pinprog_2) -> [V_BCM_COM_A429_Pinprog_2]  "V_BCMA_COM_A429_Pinprog_2"
  BCM_COM_PROC_P20/322(V_BCM_COM_A429_Pinprog_3) -> [V_BCM_COM_A429_Pinprog_3]  "V_BCMA_COM_A429_Pinprog_3"
  BCM_COM_PROC_P20/323(V_BCM_COM_A429_Pinprog_4) -> [V_BCM_COM_A429_Pinprog_4]  "V_BCMA_COM_A429_Pinprog_4"
  BCM_COM_PROC_P20/324(V_BCM_COM_A429_Pinprog_5) -> [V_BCM_COM_A429_Pinprog_5]  "V_BCMA_COM_A429_Pinprog_5"
  BCM_COM_PROC_P20/325(V_BCM_COM_A429_PP_Channel_ID) -> [V_BCM_COM_A429_PP_Channel_ID]  "V_BCMA_COM_A429_PP_Channel_ID"
  BCM_COM_PROC_P20/198(V_BCM_COM_DBCU_DISPATCH_SW_ON_Cons_Val) -> Terminator196/1  "V_BCMA_COM_DBCU_DISPATCH_SW_ON_Cons_Val"
  BCM_COM_PROC_P20/199(V_BCM_COM_LH_DBCU_BRK_CMD_FDBK_Cons) -> Terminator194/1  "V_BCMA_COM_LH_DBCU_BRK_CMD_FDBK_Cons"
  BCM_COM_PROC_P20/200(V_BCM_COM_LH_DBCU_BRK_CMD_FDBK_Cons_Val) -> Terminator198/1  "V_BCMA_COM_LH_DBCU_BRK_CMD_FDBK_Cons_Val"
  BCM_COM_PROC_P20/201(V_BCM_COM_RH_DBCU_BRK_CMD_FDBK_Cons) -> Terminator197/1  "V_BCMA_COM_RH_DBCU_BRK_CMD_FDBK_Cons"
  BCM_COM_PROC_P20/202(V_BCM_COM_RH_DBCU_BRK_CMD_FDBK_Cons_Val) -> Terminator192/1  "V_BCMA_COM_RH_DBCU_BRK_CMD_FDBK_Cons_Val"
  BCM_COM_PROC_P20/203(V_BCM_COM_DBCU_FAILED_Cons) -> Terminator195/1  "V_BCMA_COM_DBCU_FAILED_Cons"
  BCM_COM_PROC_P20/204(V_BCM_COM_DBCU_FAILED_Cons_Val) -> Terminator193/1  "V_BCMA_COM_DBCU_FAILED_Cons_Val"
  BCM_COM_PROC_P20/205(V_BCM_COM_DBCU_ALT_MODE_Cons) -> Terminator199/1  "V_BCMA_COM_DBCU_ALT_MODE_Cons"
  BCM_COM_PROC_P20/206(V_BCM_COM_DBCU_ALT_MODE_Cons_Val) -> Terminator204/1  "V_BCMA_COM_DBCU_ALT_MODE_Cons_Val"
  BCM_COM_PROC_P20/207(V_BCM_COM_ACCU_PT_Cons) -> Terminator202/1  "V_BCMA_COM_ACCU_PT_Cons"
  BCM_COM_PROC_P20/208(V_BCM_COM_ACCU_PT_Cons_Val) -> Terminator206/1  "V_BCMA_COM_ACCU_PT_Cons_Val"
  BCM_COM_PROC_P20/209(V_BCM_COM_ACCU_Pressure_State) -> Terminator205/1  "V_BCMA_COM_ACCU_Pressure_State"
  BCM_COM_PROC_P20/210(V_BCM_COM_LH_Brake_Temp_Cons) -> Terminator200/1  "V_BCMA_COM_LH_Brake_Temp_Cons"
  BCM_COM_PROC_P20/211(V_BCM_COM_LH_Brake_Temp_Cons_Val) -> Terminator203/1  "V_BCMA_COM_LH_Brake_Temp_Cons_Val"
  BCM_COM_PROC_P20/212(V_BCM_COM_RH_Brake_Temp_Cons) -> Terminator201/1  "V_BCMA_COM_RH_Brake_Temp_Cons"
  BCM_COM_PROC_P20/213(V_BCM_COM_RH_Brake_Temp_Cons_Val) -> Terminator207/1  "V_BCMA_COM_RH_Brake_Temp_Cons_Val"
  BCM_COM_PROC_P20/214(V_BCM_COM_BCP_PARK_OFF_SW_CMD_Conf) -> Terminator212/1  "V_BCMA_COM_BCP_PARK_OFF_SW_CMD_Conf"
  BCM_COM_PROC_P20/215(V_BCM_COM_Park_Sw_Cmd_Cons) -> Terminator210/1  "V_BCMA_COM_Park_Sw_Cmd_Cons"
  BCM_COM_PROC_P20/216(V_BCM_COM_Park_Sw_Cmd_Cons_Val) -> Terminator214/1  "V_BCMA_COM_Park_Sw_Cmd_Cons_Val"
  BCM_COM_PROC_P20/217(V_BCM_COM_MP_MAINT_MODE_CMD_28V_Conf) -> Terminator213/1  "V_BCMA_COM_MP_MAINT_MODE_CMD_28V_Conf"
  BCM_COM_PROC_P20/218(V_BCM_COM_MP_MAINT_MODE_CMD_GND_Conf) -> Terminator208/1  "V_BCMA_COM_MP_MAINT_MODE_CMD_GND_Conf"
  BCM_COM_PROC_P20/219(V_BCM_COM_Maint_Mode_State_Cons) -> Terminator211/1  "V_BCMA_COM_Maint_Mode_State_Cons"
  BCM_COM_PROC_P20/220(V_BCM_COM_LNLG_Tire_Press_Cons) -> Terminator209/1  "V_BCMA_COM_LNLG_Tire_Press_Cons"
  BCM_COM_PROC_P20/221(V_BCM_COM_RNLG_Tire_Press_Cons) -> Terminator215/1  "V_BCMA_COM_RNLG_Tire_Press_Cons"
  BCM_COM_PROC_P20/222(V_BCM_COM_LNLG_Tire_Press_Cons_Val) -> Terminator220/1  "V_BCMA_COM_LNLG_Tire_Press_Cons_Val"
  BCM_COM_PROC_P20/223(V_BCM_COM_RNLG_Tire_Press_Cons_Val) -> Terminator218/1  "V_BCMA_COM_RNLG_Tire_Press_Cons_Val"
  BCM_COM_PROC_P20/224(V_BCM_COM_LMLG_Outboard_Tire_Press_Cons) -> Terminator222/1  "V_BCMA_COM_LMLG_Outboard_Tire_Press_Cons"
  BCM_COM_PROC_P20/225(V_BCM_COM_LMLG_Outboard_Tire_Press_Cons_Val) -> Terminator221/1  "V_BCMA_COM_LMLG_Outboard_Tire_Press_Cons_Val"
  BCM_COM_PROC_P20/226(V_BCM_COM_LMLG_Inboard_Tire_Press_Cons) -> Terminator216/1  "V_BCMA_COM_LMLG_Inboard_Tire_Press_Cons"
  BCM_COM_PROC_P20/227(V_BCM_COM_LMLG_Inboard_Tire_Press_Cons_Val) -> Terminator219/1  "V_BCMA_COM_LMLG_Inboard_Tire_Press_Cons_Val"
  BCM_COM_PROC_P20/228(V_BCM_COM_RMLG_Inboard_Tire_Press_Cons) -> Terminator217/1  "V_BCMA_COM_RMLG_Inboard_Tire_Press_Cons"
  BCM_COM_PROC_P20/229(V_BCM_COM_RMLG_Inboard_Tire_Press_Cons_Val) -> Terminator223/1  "V_BCMA_COM_RMLG_Inboard_Tire_Press_Cons_Val"
  BCM_COM_PROC_P20/262(V_BCM_COM_A429_SSM_Avionics_Label_010) -> [V_BCM_COM_A429_SSM_Avionics_Label_010]  "V_BCMA_COM_A429_SSM_Avionics_Label_010"
  BCM_COM_PROC_P20/263(V_BCM_COM_A429_SSM_Avionics_Label_011) -> [V_BCM_COM_A429_SSM_Avionics_Label_011]  "V_BCMA_COM_A429_SSM_Avionics_Label_011"
  BCM_COM_PROC_P20/264(V_BCM_COM_A429_LNLG_Tire_Press) -> [V_BCM_COM_LNLG_Tire_Press]  "V_BCMA_COM_A429_LNLG_Tire_Press"
  BCM_COM_PROC_P20/265(V_BCM_COM_A429_RNLG_Tire_Press) -> [V_BCM_COM_RNLG_Tire_Press]  "V_BCMA_COM_A429_RNLG_Tire_Press"
  BCM_COM_PROC_P20/266(V_BCM_COM_A429_LMLG_Outboard_Tire_Press) -> [V_BCM_COM_LMLG_Tire_Press_W1]  "V_BCMA_COM_A429_LMLG_Outboard_Tire_Press"
  BCM_COM_PROC_P20/267(V_BCM_COM_A429_LMLG_Inboard_Tire_Press) -> [V_BCM_COM_LMLG_Tire_Press_W2]  "V_BCMA_COM_A429_LMLG_Inboard_Tire_Press"
  BCM_COM_PROC_P20/268(V_BCM_COM_A429_RMLG_Inboard_Tire_Press) -> [V_BCM_COM_RMLG_Tire_Press_W3]  "V_BCMA_COM_A429_RMLG_Inboard_Tire_Press"
  BCM_COM_PROC_P20/269(V_BCM_COM_A429_RMLG_Outboard_Tire_Press) -> [V_BCM_COM_RMLG_Tire_Press_W4]  "V_BCMA_COM_A429_RMLG_Outboard_Tire_Press"
  BCM_COM_PROC_P20/270(V_BCM_COM_A429_LNLG_Tire_Press_Sensor_Fail) -> [V_BCM_COM_A429_LNLG_Tire_Press_Sensor_Fail]  "V_BCMA_COM_A429_LNLG_Tire_Press_Sensor_Fail"
  BCM_COM_PROC_P20/271(V_BCM_COM_A429_RNLG_Tire_Press_Sensor_Fail) -> [V_BCM_COM_A429_RNLG_Tire_Press_Sensor_Fail]  "V_BCMA_COM_A429_RNLG_Tire_Press_Sensor_Fail"
  BCM_COM_PROC_P20/272(V_BCM_COM_A429_LMLG_Outboard_Tire_Press_Sensor_Fail) -> [V_BCM_COM_A429_LMLG_Tire_Press_Sensor_Fail_W1]  "V_BCMA_COM_A429_LMLG_Outboard_Tire_Press_Sensor_Fail"
  BCM_COM_PROC_P20/273(V_BCM_COM_A429_LMLG_Inboard_Tire_Press_Sensor_Fail) -> [V_BCM_COM_A429_LMLG_Tire_Press_Sensor_Fail_W2]  "V_BCMA_COM_A429_LMLG_Inboard_Tire_Press_Sensor_Fail"
  BCM_COM_PROC_P20/274(V_BCM_COM_A429_RMLG_Inboard_Tire_Press_Sensor_Fail) -> [V_BCM_COM_A429_RMLG_Tire_Press_Sensor_Fail_W3]  "V_BCMA_COM_A429_RMLG_Inboard_Tire_Press_Sensor_Fail"
  BCM_COM_PROC_P20/275(V_BCM_COM_A429_RMLG_Outboard_Tire_Press_Sensor_Fail) -> [V_BCM_COM_A429_RMLG_Tire_Press_Sensor_Fail_W4]  "V_BCMA_COM_A429_RMLG_Outboard_Tire_Press_Sensor_Fail"
  BCM_COM_PROC_P20/276(V_BCM_COM_A429_TPIS_Fail) -> [V_BCM_COM_A429_TPIS_Fail]  "V_BCMA_COM_A429_TPIS_Fail"
  BCM_COM_PROC_P20/277(V_BCM_COM_A429_SSM_Avionics_Label_012) -> [V_BCM_COM_A429_SSM_Avionics_Label_012]  "V_BCMA_COM_A429_SSM_Avionics_Label_012"
  BCM_COM_PROC_P20/278(V_BCM_COM_A429_SSM_Avionics_Label_013) -> [V_BCM_COM_A429_SSM_Avionics_Label_013]  "V_BCMA_COM_A429_SSM_Avionics_Label_013"
  BCM_COM_PROC_P20/279(V_BCM_COM_A429_SSM_Avionics_Label_014) -> [V_BCM_COM_A429_SSM_Avionics_Label_014]  "V_BCMA_COM_A429_SSM_Avionics_Label_014"
  BCM_COM_PROC_P20/280(V_BCM_COM_A429_SSM_Avionics_Label_015) -> [V_BCM_COM_A429_SSM_Avionics_Label_015]  "V_BCMA_COM_A429_SSM_Avionics_Label_015"
  BCM_COM_PROC_P20/281(V_BCM_COM_A429_SSM_Avionics_Label_016) -> [V_BCM_COM_A429_SSM_Avionics_Label_016]  "V_BCMA_COM_A429_SSM_Avionics_Label_016"
  BCM_COM_PROC_P20/282(V_BCM_COM_A429_SSM_Avionics_Label_017) -> [V_BCM_COM_A429_SSM_Avionics_Label_017]  "V_BCMA_COM_A429_SSM_Avionics_Label_017"
  BCM_COM_PROC_P20/283(V_BCM_COM_A429_Curr_Ord_Before_AS) -> [V_BCM_COM_A429_Curr_Ord_Before_AS]  "V_BCMA_COM_A429_Curr_Ord_Before_AS"
  BCM_COM_PROC_P20/284(V_BCM_COM_A429_AS_Curr_Order) -> [V_BCM_COM_A429_AS_Curr_Order]  "V_BCMA_COM_A429_AS_Curr_Order"
  BCM_COM_PROC_P20/285(V_BCM_COM_A429_SV_Current_Readback) -> [V_BCM_COM_A429_SV_Current_Readback]  "V_BCMA_COM_A429_SV_Current_Readback"
  BCM_COM_PROC_P20/286(V_BCM_COM_A429_SV_PT_In_Bar) -> [V_BCM_COM_A429_SV_PT_In_Bar]  "V_BCMA_COM_A429_SV_PT_In_Bar"
  BCM_COM_PROC_P20/287(V_BCM_COM_A429_SV_PT_In_PSI) -> [V_BCM_COM_A429_SV_PT_In_PSI]  "V_BCMA_COM_A429_SV_PT_In_PSI"
  BCM_COM_PROC_P20/288(V_BCM_COM_A429_Antiskid_Activity) -> [V_BCM_COM_A429_Antiskid_Activity]  "V_BCMA_COM_A429_Antiskid_Activity"
  BCM_COM_PROC_P20/289(V_BCM_COM_A429_ACCU_PT_Fail) -> [V_BCM_COM_A429_ACCU_PT_Fail]  "V_BCMA_COM_A429_ACCU_PT_Fail"
  BCM_COM_PROC_P20/290(V_BCM_COM_A429_SV_PT_Fail) -> [V_BCM_COM_A429_SV_PT_Fail]  "V_BCMA_COM_A429_SV_PT_Fail"
  BCM_COM_PROC_P20/291(V_BCM_COM_A429_SV_Fail) -> [V_BCM_COM_A429_SV_Fail]  "V_BCMA_COM_A429_SV_Fail"
  BCM_COM_PROC_P20/292(V_BCM_COM_A429_ACCU_PT) -> [V_BCM_COM_A429_ACCU_PT]  "V_BCMA_COM_A429_ACCU_PT"
  BCM_COM_PROC_P20/293(V_BCM_COM_A429_SELV_Disc_Sts_Rdbk) -> [V_BCM_COM_A429_SELV_Disc_Sts_Rdbk]  "V_BCMA_COM_A429_SELV_Disc_Sts_Rdbk"
  BCM_COM_PROC_P20/358(V_BCM_COM_ETH_DBCU_FAILED) -> [ETH_DBCU_FAILED]  "V_BCMA_COM_ETH_DBCU_FAILED"
  BCM_COM_PROC_P20/359(V_BCM_COM_ETH_ALT_MODE) -> [ETH_ALT_MODE]  "V_BCMA_COM_ETH_ALT_MODE"
  BCM_COM_PROC_P20/360(V_BCM_COM_ETH_Opp_BCM_DBCU_INHIB) -> [ETH_Opp_BCM_DBCU_INHIB]  "V_BCMA_COM_ETH_Opp_BCM_DBCU_INHIB"
  BCM_COM_PROC_P20/361(V_BCM_COM_ETH_LH_SV_Current_Order) -> [ETH_LH_SV_Current_Order]  "V_BCMA_COM_ETH_LH_SV_Current_Order"
  BCM_COM_PROC_P20/362(V_BCM_COM_ETH_RH_SV_Current_Order) -> [ETH_RH_SV_Current_Order]  "V_BCMA_COM_ETH_RH_SV_Current_Order"
  BCM_COM_PROC_P20/363(V_BCM_COM_ETH_SELV_High_Side_Cmd_Order) -> [ETH_SELV_High_Side_Cmd_Order]  "V_BCMA_COM_ETH_SELV_High_Side_Cmd_Order"
  BCM_COM_PROC_P20/364(V_BCM_COM_ETH_DBCU_Inhib_Order) -> [ETH_DBCU_Inhib_Order]  "V_BCMA_COM_ETH_DBCU_Inhib_Order"
  BCM_COM_PROC_P20/365(V_BCM_COM_ETH_FB_BCM_FAIL) -> [ETH_FB_BCM_FAIL]  "V_BCMA_COM_ETH_FB_BCM_FAIL"
  BCM_COM_PROC_P20/366(V_BCM_COM_ETH_FB_DFCS_A_RX) -> [ETH_FB_DFCS_A_RX]  "V_BCMA_COM_ETH_FB_DFCS_A_RX"
  BCM_COM_PROC_P20/367(V_BCM_COM_ETH_FB_DFCS_B_RX) -> [ETH_FB_DFCS_B_RX]  "V_BCMA_COM_ETH_FB_DFCS_B_RX"
  BCM_COM_PROC_P20/368(V_BCM_COM_ETH_FB_MAINT_MODE_DIS) -> [ETH_FB_MAINT_MODE_DIS]  "V_BCMA_COM_ETH_FB_MAINT_MODE_DIS"
  BCM_COM_PROC_P20/369(V_BCM_COM_ETH_FB_PARK_BRK_STATUS_DIS) -> [ETH_FB_PARK_BRK_STATUS_DIS]  "V_BCMA_COM_ETH_FB_PARK_BRK_STATUS_DIS"
  BCM_COM_PROC_P20/370(V_BCM_COM_ETH_FB_BCM_DBCU_MODE_DIS) -> [ETH_FB_BCM_DBCU_MODE_DIS]  "V_BCMA_COM_ETH_FB_BCM_DBCU_MODE_DIS"
  BCM_COM_PROC_P20/371(V_BCM_COM_ETH_FB_DBCU_SIMULT_ACT) -> [ETH_FB_DBCU_SIMULT_ACT]  "V_BCMA_COM_ETH_FB_DBCU_SIMULT_ACT"
  BCM_COM_PROC_P20/372(V_BCM_COM_ETH_FB_DBCU_FAIL) -> [ETH_FB_DBCU_FAIL]  "V_BCMA_COM_ETH_FB_DBCU_FAIL"
  BCM_COM_PROC_P20/373(V_BCM_COM_ETH_FB_DBCU_BRK_ORDER_FAIL) -> [ETH_FB_DBCU_BRK_ORDER_FAIL]  "V_BCMA_COM_ETH_FB_DBCU_BRK_ORDER_FAIL"
  BCM_COM_PROC_P20/374(V_BCM_COM_ETH_FB_INHIB_FAIL) -> [ETH_FB_INHIB_FAIL]  "V_BCMA_COM_ETH_FB_INHIB_FAIL"
  BCM_COM_PROC_P20/375(V_BCM_COM_ETH_FB_HYD_A_LOW_PRESS) -> [ETH_FB_HYD_A_LOW_PRESS]  "V_BCMA_COM_ETH_FB_HYD_A_LOW_PRESS"
  BCM_COM_PROC_P20/376(V_BCM_COM_ETH_FB_HYD_B_LOW_PRESS) -> [ETH_FB_HYD_B_LOW_PRESS]  "V_BCMA_COM_ETH_FB_HYD_B_LOW_PRESS"
  BCM_COM_PROC_P20/377(V_BCM_COM_ETH_FB_ACCU_LOW_PRESS) -> [ETH_FB_ACCU_LOW_PRESS]  "V_BCMA_COM_ETH_FB_ACCU_LOW_PRESS"
  BCM_COM_PROC_P20/378(V_BCM_COM_ETH_FB_ACCU_PT_FAIL) -> [ETH_FB_ACCU_PT_FAIL]  "V_BCMA_COM_ETH_FB_ACCU_PT_FAIL"
  BCM_COM_PROC_P20/379(V_BCM_COM_ETH_FB_BSELV_CMD_FAIL) -> [ETH_FB_BSELV_CMD_FAIL]  "V_BCMA_COM_ETH_FB_BSELV_CMD_FAIL"
  BCM_COM_PROC_P20/380(V_BCM_COM_ETH_FB_BSELV_JCL) -> [ETH_FB_BSELV_JCL]  "V_BCMA_COM_ETH_FB_BSELV_JCL"
  BCM_COM_PROC_P20/381(V_BCM_COM_ETH_FB_BSELV_JOP) -> [ETH_FB_BSELV_JOP]  "V_BCMA_COM_ETH_FB_BSELV_JOP"
  BCM_COM_PROC_P20/382(V_BCM_COM_ETH_FB_LH_SV_PT_FAIL) -> [ETH_FB_LH_SV_PT_FAIL]  "V_BCMA_COM_ETH_FB_LH_SV_PT_FAIL"
  BCM_COM_PROC_P20/383(V_BCM_COM_ETH_FB_LH_SV_CMD_FAIL) -> [ETH_FB_LH_SV_CMD_FAIL]  "V_BCMA_COM_ETH_FB_LH_SV_CMD_FAIL"
  BCM_COM_PROC_P20/384(V_BCM_COM_ETH_FB_LH_SV_JCL) -> [ETH_FB_LH_SV_JCL]  "V_BCMA_COM_ETH_FB_LH_SV_JCL"
  BCM_COM_PROC_P20/385(V_BCM_COM_ETH_FB_LH_SV_JOP) -> [ETH_FB_LH_SV_JOP]  "V_BCMA_COM_ETH_FB_LH_SV_JOP"
  BCM_COM_PROC_P20/386(V_BCM_COM_ETH_FB_RH_SV_PT_FAIL) -> [ETH_FB_RH_SV_PT_FAIL]  "V_BCMA_COM_ETH_FB_RH_SV_PT_FAIL"
  BCM_COM_PROC_P20/387(V_BCM_COM_ETH_FB_RH_SV_CMD_FAIL) -> [ETH_FB_RH_SV_CMD_FAIL]  "V_BCMA_COM_ETH_FB_RH_SV_CMD_FAIL"
  BCM_COM_PROC_P20/388(V_BCM_COM_ETH_FB_RH_SV_JCL) -> [ETH_FB_RH_SV_JCL]  "V_BCMA_COM_ETH_FB_RH_SV_JCL"
  BCM_COM_PROC_P20/389(V_BCM_COM_ETH_FB_RH_SV_JOP) -> [ETH_FB_RH_SV_JOP]  "V_BCMA_COM_ETH_FB_RH_SV_JOP"
  BCM_COM_PROC_P20/326(V_BCM_COM_A429_DBCU_Dispatch_Conf) -> [V_BCM_COM_A429_DBCU_Dispatch_Conf]  "V_BCMA_COM_A429_DBCU_Dispatch_Conf"
  BCM_COM_PROC_P20/327(V_BCM_COM_A429_Maint_Mode_Active) -> [V_BCM_COM_A429_Maint_Mode_Active]  "V_BCMA_COM_A429_Maint_Mode_Active"
  BCM_COM_PROC_P20/328(V_BCM_COM_A429_Maint_Mode_Req_GND) -> [V_BCM_COM_A429_Maint_Mode_Req_GND]  "V_BCMA_COM_A429_Maint_Mode_Req_GND"
  BCM_COM_PROC_P20/329(V_BCM_COM_A429_Maint_Mode_Req_28V) -> [V_BCM_COM_A429_Maint_Mode_Req_28V]  "V_BCMA_COM_A429_Maint_Mode_Req_28V"
  BCM_COM_PROC_P20/330(V_BCM_COM_A429_Pinprog_Fail) -> [V_BCM_COM_A429_Pinprog_Fail]  "V_BCMA_COM_A429_Pinprog_Fail"
  BCM_COM_PROC_P20/331(V_BCM_COM_A429_Norm_Brake_Fail) -> [V_BCM_COM_A429_Norm_Brake_Fail]  "V_BCMA_COM_A429_Norm_Brake_Fail"
  BCM_COM_PROC_P20/332(V_BCM_COM_A429_BCM_Passivated) -> [V_BCM_COM_A429_BCM_Passivated]  "V_BCMA_COM_A429_BCM_Passivated"
  BCM_COM_PROC_P20/333(V_BCM_COM_A429_BCM_Fail) -> [V_BCM_COM_A429_BCM_Fail]  "V_BCMA_COM_A429_BCM_Fail"
  BCM_COM_PROC_P20/334(V_BCM_COM_A429_DBCU_Fail) -> [V_BCM_COM_A429_DBCU_Fail]  "V_BCMA_COM_A429_DBCU_Fail"
  BCM_COM_PROC_P20/335(V_BCM_COM_A429_Alternate_Fail) -> [V_BCM_COM_A429_Alternate_Fail]  "V_BCMA_COM_A429_Alternate_Fail"
  BCM_COM_PROC_P20/336(V_BCM_COM_A429_DBCU_LH_Brk_Cmd_Fdbk) -> [V_BCM_COM_A429_DBCU_LH_Brk_Cmd_Fdbk]  "V_BCMA_COM_A429_DBCU_LH_Brk_Cmd_Fdbk"
  BCM_COM_PROC_P20/337(V_BCM_COM_A429_DBCU_RH_Brk_Cmd_Fdbk) -> [V_BCM_COM_A429_DBCU_RH_Brk_Cmd_Fdbk]  "V_BCMA_COM_A429_DBCU_RH_Brk_Cmd_Fdbk"
  BCM_COM_PROC_P20/338(V_BCM_COM_A429_DBCU_Inhib_Opp_Side) -> [V_BCM_COM_A429_DBCU_Inhib_Opp_Side]  "V_BCMA_COM_A429_DBCU_Inhib_Opp_Side"
  BCM_COM_PROC_P20/339(V_BCM_COM_A429_DBCU_Alt_Mode) -> [V_BCM_COM_A429_DBCU_Alt_Mode]  "V_BCMA_COM_A429_DBCU_Alt_Mode"
  BCM_COM_PROC_P20/340(V_BCM_COM_A429_SSM_DFCS_Label_100) -> [V_BCM_COM_A429_SSM_DFCS_Label_100]  "V_BCMA_COM_A429_SSM_DFCS_Label_100"
  BCM_COM_PROC_P20/341(V_BCM_COM_A429_Global_Wheel_Spd) -> [V_BCM_COM_A429_Global_Wheel_Spd]  "V_BCMA_COM_A429_Global_Wheel_Spd"
  BCM_COM_PROC_P20/342(V_BCM_COM_ETH_HYD_A_PRESS) -> [ETH_HYD_A_PRESS]  "V_BCMA_COM_ETH_HYD_A_PRESS"
  BCM_COM_PROC_P20/343(V_BCM_COM_ETH_HYD_B_PRESS) -> [ETH_HYD_B_PRESS]  "V_BCMA_COM_ETH_HYD_B_PRESS"
  BCM_COM_PROC_P20/344(V_BCM_COM_ETH_ENG1_RUNNING) -> [ETH_ENG1_RUNNING]  "V_BCMA_COM_ETH_ENG1_RUNNING"
  BCM_COM_PROC_P20/345(V_BCM_COM_ETH_ENG2_RUNNING) -> [ETH_ENG2_RUNNING]  "V_BCMA_COM_ETH_ENG2_RUNNING"
  BCM_COM_PROC_P20/346(V_BCM_COM_ETH_LMLG_Dnlk) -> [ETH_LMLG_Dnlk]  "V_BCMA_COM_ETH_LMLG_Dnlk"
  BCM_COM_PROC_P20/347(V_BCM_COM_ETH_RMLG_Dnlk) -> [ETH_RMLG_Dnlk]  "V_BCMA_COM_ETH_RMLG_Dnlk"
  BCM_COM_PROC_P20/348(V_BCM_COM_ETH_Lever_Up) -> [ETH_Lever_Up]  "V_BCMA_COM_ETH_Lever_Up"
  BCM_COM_PROC_P20/349(V_BCM_COM_ETH_BCP_BCM_ALT_SW_ON_CMD) -> [ETH_BCP_BCM_ALT_SW_ON_CMD]  "V_BCMA_COM_ETH_BCP_BCM_ALT_SW_ON_CMD"
  BCM_COM_PROC_P20/350(V_BCM_COM_ETH_MP_MAINT_MODE_CMD_GND) -> [ETH_MP_MAINT_MODE_CMD_GND]  "V_BCMA_COM_ETH_MP_MAINT_MODE_CMD_GND"
  BCM_COM_PROC_P20/351(V_BCM_COM_ETH_MP_MAINT_MODE_CMD_28V) -> [ETH_MAINT_MODE_CMD_28V]  "V_BCMA_COM_ETH_MP_MAINT_MODE_CMD_28V"
  BCM_COM_PROC_P20/352(V_BCM_COM_ETH_MP_BCMA_ALT_DISP_SW) -> [ETH_BCMA_ALT_DISP_SW]  "V_BCMA_COM_ETH_MP_BCMA_ALT_DISP_SW"
  BCM_COM_PROC_P20/353(V_BCM_COM_ETH_PBSELV_ON_POS) -> [ETH_PBSELV_ON_POS]  "V_BCMA_COM_ETH_PBSELV_ON_POS"
  BCM_COM_PROC_P20/354(V_BCM_COM_ETH_DBCU_BRK_ORDER_FAIL) -> [ETH_DBCU_BRK_ORDER_FAIL]  "V_BCMA_COM_ETH_DBCU_BRK_ORDER_FAIL"
  BCM_COM_PROC_P20/355(V_BCM_COM_ETH_DISPATCH_SW_ON) -> [ETH_DISPATCH_SW_ON]  "V_BCMA_COM_ETH_DISPATCH_SW_ON"
  BCM_COM_PROC_P20/356(V_BCM_COM_ETH_LH_DBCU_BRK_CMD_FDBK) -> [ETH_LH_DBCU_BRK_CMD_FDBK]  "V_BCMA_COM_ETH_LH_DBCU_BRK_CMD_FDBK"
  BCM_COM_PROC_P20/357(V_BCM_COM_ETH_RH_DBCU_BRK_CMD_FDBK) -> [ETH_RH_DBCU_BRK_CMD_FDBK]  "V_BCMA_COM_ETH_RH_DBCU_BRK_CMD_FDBK"
  BCM_COM_PROC_P20/390(V_BCM_COM_ETH_AC_State) -> [ETH_AC_State]  "V_BCMA_COM_ETH_AC_State"
  BCM_COM_PROC_P20/391(V_BCM_COM_ETH_AC_Flight_Phase) -> [ETH_AC_Flight_Phase]  "V_BCMA_COM_ETH_AC_Flight_Phase"
  BCM_COM_PROC_P20/392(V_BCM_COM_ETH_Braking_Mode) -> [ETH_Braking_Mode]  "V_BCMA_COM_ETH_Braking_Mode"
  BCM_COM_PROC_P20/393(V_BCM_COM_ETH_Braking_Norm_FT_Seq) -> [ETH_Braking_Norm_FT_Seq]  "V_BCMA_COM_ETH_Braking_Norm_FT_Seq"
  BCM_COM_PROC_P20/394(V_BCM_COM_ETH_Braking_Alt_FT_Seq) -> [ETH_Braking_Alt_FT_Seq]  "V_BCMA_COM_ETH_Braking_Alt_FT_Seq"
  BCM_COM_PROC_P20/395(V_BCM_COM_ETH_FB_LG_LEVER_FAIL) -> [ETH_FB_LG_LEVER_FAIL]  "V_BCMA_COM_ETH_FB_LG_LEVER_FAIL"
  BCM_COM_PROC_P20/396(V_BCM_COM_ETH_FB_LMLG_DWNLOCK_FAIL) -> [ETH_FB_LMLG_DWNLOCK_FAIL]  "V_BCMA_COM_ETH_FB_LMLG_DWNLOCK_FAIL"
  BCM_COM_PROC_P20/397(V_BCM_COM_ETH_FB_RMLG_DWNLOCK_FAIL) -> [ETH_FB_RMLG_DWNLOCK_FAIL]  "V_BCMA_COM_ETH_FB_RMLG_DWNLOCK_FAIL"
  BCM_COM_PROC_P20/398(V_BCM_COM_ETH_TARGET_HW_ID) -> Terminator388/1  "V_BCMA_COM_ETH_TARGET_HW_ID"
  BCM_COM_PROC_P20/399(V_BCM_COM_ETH_Invalid_Config) -> [ETH_Invalid_Config]  "V_BCMA_COM_ETH_Invalid_Config"
  BCM_COM_PROC_P20/400(V_BCM_COM_ETH_FB_LH_OUT_TACHO_FAIL) -> [ETH_FB_LH_OUT_TACHO_FAIL]  "V_BCMA_COM_ETH_FB_LH_OUT_TACHO_FAIL"
  BCM_COM_PROC_P20/401(V_BCM_COM_ETH_FB_LH_IN_TACHO_FAIL) -> [ETH_FB_LH_IN_TACHO_FAIL]  "V_BCMA_COM_ETH_FB_LH_IN_TACHO_FAIL"
  BCM_COM_PROC_P20/402(V_BCM_COM_ETH_FB_RH_IN_TACHO_FAIL) -> [ETH_FB_RH_IN_TACHO_FAIL]  "V_BCMA_COM_ETH_FB_RH_IN_TACHO_FAIL"
  BCM_COM_PROC_P20/403(V_BCM_COM_ETH_FB_RH_OUT_TACHO_FAIL) -> [ETH_FB_RH_OUT_TACHO_FAIL]  "V_BCMA_COM_ETH_FB_RH_OUT_TACHO_FAIL"
  BCM_COM_PROC_P20/404(V_BCM_COM_ETH_TT_in_progress_id) -> [ETH_TT_in_progress_id]  "V_BCMA_COM_ETH_TT_in_progress_id"
  BCM_COM_PROC_P20/405(V_BCM_COM_ETH_TT_rejection_cause) -> [ETH_TT_rejection_cause]  "V_BCMA_COM_ETH_TT_rejection_cause"
  BCM_COM_PROC_P20/406(V_BCM_COM_ETH_TT_rejected) -> [ETH_TT_rejected]  "V_BCMA_COM_ETH_TT_rejected"
  BCM_COM_PROC_P20/407(V_BCM_COM_ETH_TT_completed) -> [ETH_TT_completed]  "V_BCMA_COM_ETH_TT_completed"
  BCM_COM_PROC_P20/408(V_BCM_COM_ETH_TT_result_significant) -> [ETH_TT_result_significant]  "V_BCMA_COM_ETH_TT_result_significant"
  [Engine1_Running_Val] -> BCM_COM_PROC_P20/110(V_BCM_COM_Engine_1_Running_Acq_Val)
  [Engine2_Running_Val] -> BCM_COM_PROC_P20/111(V_BCM_COM_Engine_2_Running_Acq_Val)
  [Hyd_A_Press_Val] -> BCM_COM_PROC_P20/112(V_BCM_COM_Hyd_A_Press_Acq_Val)
  [Hyd_B_Press_Val] -> BCM_COM_PROC_P20/113(V_BCM_COM_Hyd_B_Press_Acq_Val)
  [BCM_CCDL_Conf_Flt] -> BCM_COM_PROC_P20/103(V_BCM_COM_BCM_CCDL_Conf_Flt)
  [BCM_CCDL_Unconf_Flt] -> BCM_COM_PROC_P20/104(V_BCM_COM_BCM_CCDL_Unconf_Flt)
  [BCM_DBCU_INHIBITION_Conf_Flt] -> BCM_COM_PROC_P20/107(V_BCM_COM_BCM_DBCU_INHIBITION_Conf_Flt)
  [BCM_DBCU_INHIBITION_Unconf_Flt] -> BCM_COM_PROC_P20/108(V_BCM_COM_BCM_DBCU_INHIBITION_Unconf_Flt)
  [DBCU_BRK_ORDER_FAIL] -> Logical Operator1/1
  Constant44/1 -> BCM_COM_PROC_P20/128(V_BCM_COM_DBCU_DISPATCH_SW_ON_Acq)
  [LH_DBCU_BRK_CMD_FEEDBACK] -> BCM_COM_PROC_P20/129(V_BCM_COM_LH_DBCU_BRK_CMD_FDBK_Acq)
  [RH_DBCU_BRK_CMD_FEEDBACK] -> BCM_COM_PROC_P20/130(V_BCM_COM_RH_DBCU_BRK_CMD_FDBK_Acq)
  [DBCU_FAILED] -> Logical Operator2/1
  [DBCU_ALTERNATE_MODE] -> BCM_COM_PROC_P20/132(V_BCM_COM_DBCU_ALT_MODE_Acq)
  [DBCU_BRK_ORDER_FAIL_Conf_Flt] -> BCM_COM_PROC_P20/133(V_BCM_COM_DBCU_BRK_ORDER_FAIL_Conf_Flt)
  [DBCU_BRK_ORDER_FAIL_Unconf_Flt] -> BCM_COM_PROC_P20/134(V_BCM_COM_DBCU_BRK_ORDER_FAIL_Unconf_Flt)
  [DBCU_DISPATCH_SW_ON_Conf_Flt] -> BCM_COM_PROC_P20/135(V_BCM_COM_DBCU_DISPATCH_SW_ON_Conf_Flt)
  [DBCU_DISPATCH_SW_ON_Unconf_Flt] -> BCM_COM_PROC_P20/136(V_BCM_COM_DBCU_DISPATCH_SW_ON_Unconf_Flt)
  [RH_DBCU_BRK_CMD_FDBK_Unconf_Flt] -> BCM_COM_PROC_P20/140(V_BCM_COM_RH_DBCU_BRK_CMD_FDBK_Unconf_Flt)
  [RH_DBCU_BRK_CMD_FDBK_Conf_Flt] -> BCM_COM_PROC_P20/139(V_BCM_COM_RH_DBCU_BRK_CMD_FDBK_Conf_Flt)
  [DBCU_FAILED_Unconf_Flt] -> BCM_COM_PROC_P20/142(V_BCM_COM_DBCU_FAILED_Unconf_Flt)
  [DBCU_FAILED_Conf_Flt] -> BCM_COM_PROC_P20/141(V_BCM_COM_DBCU_FAILED_Conf_Flt)
  [DBCU_ALT_MODE_Unconf_Flt] -> BCM_COM_PROC_P20/144(V_BCM_COM_DBCU_ALT_MODE_Unconf_Flt)
  [DBCU_ALT_MODE_Conf_Flt] -> BCM_COM_PROC_P20/143(V_BCM_COM_DBCU_ALT_MODE_Conf_Flt)
  [ACCU_PT_Unconf_Flt] -> BCM_COM_PROC_P20/146(V_BCM_COM_ACCU_PT_Unconf_Flt)
  [ACCU_PT_Conf_Flt] -> BCM_COM_PROC_P20/145(V_BCM_COM_ACCU_PT_Conf_Flt)
  [ACCU_PT_PRESSURE] -> BCM_COM_PROC_P20/147(V_BCM_COM_ACCU_PT_Acq)
  [LH_BTS_Unconf_Flt] -> BCM_COM_PROC_P20/150(V_BCM_COM_LH_BTS_Unconf_Flt)
  [LH_BTS_Conf_Flt] -> BCM_COM_PROC_P20/149(V_BCM_COM_LH_BTS_Conf_Flt)
  [RH_BTS_Unconf_Flt] -> BCM_COM_PROC_P20/153(V_BCM_COM_RH_BTS_Unconf_Flt)
  [RH_BTS_Conf_Flt] -> BCM_COM_PROC_P20/152(V_BCM_COM_RH_BTS_Conf_Flt)
  [BCP_PARK_OFF_SW_CMD_Unconf_Flt] -> BCM_COM_PROC_P20/156(V_BCM_COM_BCP_PARK_OFF_SW_CMD_Unconf_Flt)
  [BCP_PARK_OFF_SW_CMD_Conf_Flt] -> BCM_COM_PROC_P20/155(V_BCM_COM_BCP_PARK_OFF_SW_CMD_Conf_Flt)
  [BCP_PARK_OFF_SW_CMD] -> BCM_COM_PROC_P20/154(V_BCM_COM_BCP_PARK_OFF_SW_CMD_Acq)
  [MP_MAINT_MODE_CMD_BCM_GND] -> BCM_COM_PROC_P20/158(V_BCM_COM_MP_MAINT_MODE_CMD_GND_Acq)
  [MP_MAINT_MODE_CMD_BCM_28V] -> BCM_COM_PROC_P20/157(V_BCM_COM_MP_MAINT_MODE_CMD_28V_Acq)
  [LNLG_Tire_Press_Unconf_Flt] -> BCM_COM_PROC_P20/161(V_BCM_COM_LNLG_Tire_Press_Unconf_Flt)
  [LNLG_Tire_Press_Conf_Flt] -> BCM_COM_PROC_P20/160(V_BCM_COM_LNLG_Tire_Press_Conf_Flt)
  [LNLG_Tyre_Pressure] -> BCM_COM_PROC_P20/159(V_BCM_COM_LNLG_Tire_Press_Acq)
  [RNLG_Tire_Press_Unconf_Flt] -> BCM_COM_PROC_P20/164(V_BCM_COM_RNLG_Tire_Press_Unconf_Flt)
  [RNLG_Tire_Press_Conf_Flt] -> BCM_COM_PROC_P20/163(V_BCM_COM_RNLG_Tire_Press_Conf_Flt)
  [RNLG_Tyre_Pressure] -> BCM_COM_PROC_P20/162(V_BCM_COM_RNLG_Tire_Press_Acq)
  [LMLG_Outboard_Tire_Press_Unconf_Flt] -> BCM_COM_PROC_P20/167(V_BCM_COM_LMLG_Outboard_Tire_Press_Unconf_Flt)
  [LMLG_Outboard_Tire_Press_Conf_Flt] -> BCM_COM_PROC_P20/166(V_BCM_COM_LMLG_Outboard_Tire_Press_Conf_Flt)
  [LMLG_Inboard_Tire_Press_Unconf_Flt] -> BCM_COM_PROC_P20/170(V_BCM_COM_LMLG_Inboard_Tire_Press_Unconf_Flt)
  [LMLG_Inboard_Tire_Press_Conf_Flt] -> BCM_COM_PROC_P20/169(V_BCM_COM_LMLG_Inboard_Tire_Press_Conf_Flt)
  [LMLG_Inboard_Tyre_Pressure] -> BCM_COM_PROC_P20/168(V_BCM_COM_LMLG_Inboard_Tire_Press_Acq)
  [RMLG_Inboard_Tire_Press_Unconf_Flt] -> BCM_COM_PROC_P20/173(V_BCM_COM_RMLG_Inboard_Tire_Press_Unconf_Flt)
  [RMLG_Inboard_Tire_Press_Conf_Flt] -> BCM_COM_PROC_P20/172(V_BCM_COM_RMLG_Inboard_Tire_Press_Conf_Flt)
  [RMLG_Inboard_Tyre_Pressure] -> BCM_COM_PROC_P20/171(V_BCM_COM_RMLG_Inboard_Tire_Press_Acq)
  [RMLG_Outboard_Tire_Press_Unconf_Flt] -> BCM_COM_PROC_P20/176(V_BCM_COM_RMLG_Outboard_Tire_Press_Unconf_Flt)
  [RMLG_Outboard_Tire_Press_Conf_Flt] -> BCM_COM_PROC_P20/175(V_BCM_COM_RMLG_Outboard_Tire_Press_Conf_Flt)
  [RMLG_Outboard_Tyre_Pressure] -> BCM_COM_PROC_P20/174(V_BCM_COM_RMLG_Outboard_Tire_Press_Acq)
  [V_BCM_COM_Whl_AS_Curr_Order] -> BCM_COM_PROC_P20/177(V_BCM_COM_Whl_AS_Curr_Order)
  [V_BCM_COM_Whl_AS_Activity] -> BCM_COM_PROC_P20/179(V_BCM_COM_Whl_AS_Activity)
  [DFCSA_ALT_Mode_1_Val] -> BCM_COM_PROC_P20/114(V_BCM_COM_DFCS_A_DBCU_ALT_Mode_1_Acq_Val)
  [DFCSA_ALT_Mode_2_Val] -> BCM_COM_PROC_P20/115(V_BCM_COM_DFCS_A_DBCU_ALT_Mode_2_Acq_Val)
  [DFCSB_ALT_Mode_1_Val] -> BCM_COM_PROC_P20/116(V_BCM_COM_DFCS_B_DBCU_ALT_Mode_1_Acq_Val)
  [DFCSB_ALT_Mode_2_Val] -> BCM_COM_PROC_P20/117(V_BCM_COM_DFCS_B_DBCU_ALT_Mode_2_Acq_Val)
  Bus Selector2/5 -> [UTC_time_hours]  "<BUS_A429_GenIO_1A_GPHS_LABEL_150_UTC_time_hours_2>"
  Bus Selector2/6 -> [UTC_time_minutes]  "<BUS_A429_GenIO_1A_GPHS_LABEL_150_UTC_time_minutes_2>"
  Bus Selector2/7 -> [UTC_time_seconds]  "<BUS_A429_GenIO_1A_GPHS_LABEL_150_UTC_time_seconds_2>"
  [UTC_time_seconds] -> BCM_COM_PROC_P20/124(V_BCM_COM_UTC_Time_Seconds_Acq)
  [UTC_time_hours] -> BCM_COM_PROC_P20/118(V_BCM_COM_UTC_Time_Hours_Acq)
  [UTC_time_minutes] -> BCM_COM_PROC_P20/121(V_BCM_COM_UTC_Time_Minutes_Acq)
  [UTC_Time_Hours_Conf_Flt] -> BCM_COM_PROC_P20/119(V_BCM_COM_UTC_Time_Hours_Conf_Flt)
  [UTC_Time_Hours_Unconf_Flt] -> BCM_COM_PROC_P20/120(V_BCM_COM_UTC_Time_Hours_Unconf_Flt)
  [UTC_Time_Minutes_Conf_Flt] -> BCM_COM_PROC_P20/122(V_BCM_COM_UTC_Time_Minutes_Conf_Flt)
  [UTC_Time_Minutes_Unconf_Flt] -> BCM_COM_PROC_P20/123(V_BCM_COM_UTC_Time_Minutes_Unconf_Flt)
  [UTC_Time_Seconds_Conf_Flt] -> BCM_COM_PROC_P20/125(V_BCM_COM_UTC_Time_Seconds_Conf_Flt)
  [UTC_Time_Seconds_Unconf_Flt] -> BCM_COM_PROC_P20/126(V_BCM_COM_UTC_Time_Seconds_Unconf_Flt)
  Mux10/1 -> BCM_COM_PROC_P20/178(V_BCM_COM_SV_Current_Readback)
  [SELV_CMD_Readback] -> BCM_COM_PROC_P20/181(V_BCM_COM_SELV_High_Side_Readback)
  [CF_LH_SV_SC] -> BCM_COM_PROC_P20/182(V_BCM_COM_CF_LH_SV_SC)
  [CF_LH_SV_OC] -> BCM_COM_PROC_P20/183(V_BCM_COM_CF_LH_SV_OC)
  [CF_SELV_SC] -> BCM_COM_PROC_P20/186(V_BCM_COM_CF_SELV_SC)
  [CF_SELV_OC] -> BCM_COM_PROC_P20/187(V_BCM_COM_CF_SELV_OC)
  [CF_RH_SV_OC] -> BCM_COM_PROC_P20/185(V_BCM_COM_CF_RH_SV_OC)
  [CF_RH_SV_SC] -> BCM_COM_PROC_P20/184(V_BCM_COM_CF_RH_SV_SC)
  [CF_SELV_JOP] -> BCM_COM_PROC_P20/188(V_BCM_COM_CF_SELV_JOP)
  [CF_SELV_JCL] -> BCM_COM_PROC_P20/189(V_BCM_COM_CF_SELV_JCL)
  [CF_PARK_BRK] -> BCM_COM_PROC_P20/190(V_BCM_COM_CF_PARK_BRK)
  [CF_RESIDUAL_PRESS] -> BCM_COM_PROC_P20/191(V_BCM_COM_CF_RESIDUAL_PRESS)
  [Avionics_Conf_Flt] -> BCM_COM_PROC_P20/192(V_BCM_COM_Avionics_Conf_Flt)
  [DFCS_A_Conf_Flt] -> BCM_COM_PROC_P20/193(V_BCM_COM_DFCS_A_Conf_Flt)
  [DFCSA_Capsule_Validity] -> BCM_COM_PROC_P20/194(V_BCM_COM_DFCS_A_DFCS_BCM_Caps_Val)
  [DFCS_B_Conf_Flt] -> BCM_COM_PROC_P20/195(V_BCM_COM_DFCS_B_Conf_Flt)
  [DFCSB_Capsule_Validity] -> BCM_COM_PROC_P20/196(V_BCM_COM_DFCS_B_DFCS_BCM_Caps_Val)
  Mux16/1 -> BCM_COM_PROC_P20/197(V_BCM_COM_PPRG_i_Acquired)
  [PIN_PROG_BCM_1] -> Mux16/1
  [PIN_PROG_BCM_2] -> Mux16/2
  [PIN_PROG_BCM_3] -> Mux16/3
  Pin_Prog/1 -> Mux16/5, Mux16/4
  [PPRG_Fault] -> BCM_COM_PROC_P20/198(V_BCM_COM_PPRG_Fault)
  [DBCU_Conf_Flt] -> BCM_COM_PROC_P20/199(V_BCM_COM_DBCU_Conf_Flt)
  [V_BCM_COM_SV_Current_Order] -> BCM_COM_PROC_P20/201(V_BCM_COM_SV_Current_Order)
  [CF_BSELV_OC] -> BCM_COM_PROC_P20/202(V_BCM_COM_CF_BSELV_OC)
  [CF_BSELV_SC] -> BCM_COM_PROC_P20/203(V_BCM_COM_CF_BSELV_SC)
  [CF_BSELV_JCL] -> BCM_COM_PROC_P20/204(V_BCM_COM_CF_BSELV_JCL)
  [CF_BSELV_JOP] -> BCM_COM_PROC_P20/205(V_BCM_COM_CF_BSELV_JOP)
  [LH_SV_PT_Conf_Flt] -> BCM_COM_PROC_P20/206(V_BCM_COM_LH_SV_PT_Conf_Flt)
  [CF_SV_DRIFT] -> BCM_COM_PROC_P20/207(V_BCM_COM_CF_SV_DRIFT)
  [CF_LH_SV_JCL] -> BCM_COM_PROC_P20/208(V_BCM_COM_CF_LH_SV_JCL)
  [CF_LH_SV_JOP] -> BCM_COM_PROC_P20/209(V_BCM_COM_CF_LH_SV_JOP)
  [RH_SV_PT_Conf_Flt] -> BCM_COM_PROC_P20/210(V_BCM_COM_RH_SV_PT_Conf_Flt)
  [CF_RH_SV_JCL] -> BCM_COM_PROC_P20/211(V_BCM_COM_CF_RH_SV_JCL)
  [CF_RH_SV_JOP] -> BCM_COM_PROC_P20/212(V_BCM_COM_CF_RH_SV_JOP)
  [V_BCM_COM_A429_SSM_Avionics_Label_005] -> Data Type Conversion12/1
  [V_BCM_COM_A429_SSM_Avionics_Label_006] -> Data Type Conversion13/1
  [V_BCM_COM_A429_SSM_Avionics_Label_021] -> Data Type Conversion21/1
  [V_BCM_COM_A429_SSM_Avionics_Label_022] -> Data Type Conversion23/1
  [V_BCM_COM_A429_SSM_Avionics_Label_030] -> Data Type Conversion22/1
  [V_BCM_COM_A429_SSM_Avionics_Label_031] -> Data Type Conversion33/1
  [V_BCM_COM_A429_SSM_Avionics_Label_032] -> Data Type Conversion34/1
  [V_BCM_COM_A429_SSM_Avionics_Label_033] -> Data Type Conversion26/1
  [V_BCM_COM_A429_SSM_Avionics_Label_040] -> Data Type Conversion32/1
  [V_BCM_COM_A429_SSM_Avionics_Label_041] -> Data Type Conversion31/1
  [V_BCM_COM_A429_SSM_Avionics_Label_042] -> Data Type Conversion35/1
  [V_BCM_COM_A429_SSM_Avionics_Label_043] -> Data Type Conversion37/1
  [V_BCM_COM_A429_SSM_Avionics_Label_050] -> Data Type Conversion36/1
  [V_BCM_COM_A429_Wheel_Speed_W34] -> Demux1/1
  [V_BCM_COM_A429_Wheel_Speed_W12] -> Demux2/1
  Demux2/1 -> BUS_A429_BCMA_DFCS13_TX/3(BCMCP_LHO_Wheel_Speed)
  Demux2/2 -> BUS_A429_BCMA_DFCS13_TX/4(BCMCP_LHI_Wheel_Speed)
  [V_BCM_COM_A429_Wheel_Speed_W34] -> Demux5/1
  [V_BCM_MON_A429_SP_Wheel_Speed_W34] -> Demux11/1
  Demux10/2 -> BUS_A429_BCMA_DFCS13_TX/18(BCMSP_LHI_Wheel_Speed)
  Demux10/1 -> BUS_A429_BCMA_DFCS13_TX/17(BCMSP_LHO_Wheel_Speed)
  [V_BCM_MON_A429_SP_Wheel_Speed_W12] -> Demux10/1
  Demux11/2 -> BUS_A429_BCMA_DFCS13_TX/20(BCMSP_RHO_Wheel_Speed)
  Demux11/1 -> BUS_A429_BCMA_DFCS13_TX/19(BCMSP_RHI_Wheel_Speed)
  [V_BCM_COM_A429_TACHO_Fail_W12] -> Demux12/1
  [V_BCM_COM_A429_TACHO_Fail_W34] -> Demux13/1
  [V_BCM_COM_A429_SSM_Avionics_Label_001] -> Data Type Conversion8/1
  [V_BCM_COM_A429_SSM_Avionics_Label_002] -> Data Type Conversion9/1
  [V_BCM_COM_A429_SSM_Avionics_Label_003] -> Data Type Conversion10/1
  [V_BCM_COM_A429_SSM_Avionics_Label_004] -> Data Type Conversion11/1
  [V_BCM_COM_A429_LH_Brake_Temp] -> BUS_A429_BCMA_GenIO_2_TX/19(BCMCP_LH_outboard_brake_temp)
  [V_BCM_COM_A429_RH_Brake_Temp] -> BUS_A429_BCMA_GenIO_2_TX/20(BCMCP_RH_outboard_brake_temp)
  [V_BCM_COM_A429_SSM_DFCS_Label_101] -> Data Type Conversion1/1
  [V_BCM_COM_A429_SSM_DFCS_Label_102] -> Data Type Conversion2/1
  [V_BCM_COM_A429_SSM_DFCS_Label_103] -> Data Type Conversion3/1
  [V_BCM_COM_A429_SSM_DFCS_Label_104] -> Data Type Conversion4/1
  [V_BCM_COM_A429_SSM_Avionics_Label_010] -> Data Type Conversion14/1
  [V_BCM_COM_A429_SSM_Avionics_Label_011] -> Data Type Conversion16/1
  [V_BCM_COM_A429_SSM_Avionics_Label_012] -> Data Type Conversion15/1
  [V_BCM_COM_A429_SSM_Avionics_Label_013] -> Data Type Conversion24/1
  [V_BCM_COM_A429_SSM_Avionics_Label_014] -> Data Type Conversion25/1
  [V_BCM_COM_A429_SSM_Avionics_Label_015] -> Data Type Conversion17/1
  [V_BCM_COM_A429_SSM_Avionics_Label_016] -> Data Type Conversion18/1
  [V_BCM_COM_A429_SSM_Avionics_Label_017] -> Data Type Conversion19/1
  [V_BCM_COM_A429_SSM_Avionics_Label_020] -> Data Type Conversion20/1
  [V_BCM_COM_A429_SSM_Avionics_Label_034] -> Data Type Conversion27/1
  [V_BCM_COM_A429_SSM_Avionics_Label_035] -> Data Type Conversion28/1
  [V_BCM_COM_A429_SSM_Avionics_Label_036] -> Data Type Conversion29/1
  [V_BCM_COM_A429_SSM_Avionics_Label_037] -> Data Type Conversion30/1
  Demux7/2 -> BUS_A429_BCMA_GenIO_2_TX/44(BCMCP_RH_antiskid_current_order)
